simulink model "SimulinkAnalysisofCheetahTail"  (R2022a)
(part 7 of 21)

t6762 = -t4173.*(t1786+t1810+t1964+t2047+t2152-t2401-t2797-t2860-t3076+t3167-t3232-t3278+t3582+t3583-t3837+t1430.*(t539+t641).*3.36554e-3+t1181.*(t105-t465).*3.372786875e-3+t11.*t381.*(t534-t546).*3.372786875e-3);
t6763 = -t4162.*(t1692+t1899+t1910+t2152+t2155-t2401-t2936-t2962-t3031-t3147+t3307-t3387+t3582+t3583-t3837+t1430.*(t539+t641).*3.36554e-3+t1181.*(t105-t465).*3.36554e-3+t11.*t381.*(t534-t546).*3.36554e-3);
t6764 = (-t1262+t1701+t9.*t868.*(t105-t465)).*(t1786+t1810+t1964+t2047+t2152-t2401-t2797-t2860-t3076+t3167-t3232-t3278+t3582+t3583-t3837+t1430.*(t539+t641).*3.36554e-3+t1181.*(t105-t465).*3.372786875e-3+t11.*t381.*(t534-t546).*3.372786875e-3);
t6770 = -t4313.*(t1692+t1899+t1910+t2152+t2155-t2401-t2936-t2962-t3031-t3147+t3307-t3387+t3582+t3583-t3837+t1430.*(t539+t641).*3.36554e-3+t1181.*(t105-t465).*3.36554e-3+t11.*t381.*(t534-t546).*3.36554e-3);
t6772 = (t1332+t2368+t1512.*(t105-t465)).*(t1786+t1810+t1964+t2047+t2152-t2401-t2797-t2860-t3076+t3167-t3232-t3278+t3582+t3583-t3837+t1430.*(t539+t641).*3.36554e-3+t1181.*(t105-t465).*3.372786875e-3+t11.*t381.*(t534-t546).*3.372786875e-3);
t6773 = -t4392.*(t1692+t1786+t1910+t1964+t2305-t2600-t2797-t2860-t2936-t3147+t3167-t3232+t3720+t3721-t3903+t1430.*(t539+t641).*3.372816795e-3+t1181.*(t105-t465).*3.36554e-3+t11.*t381.*(t534-t546).*3.36554e-3);
t6775 = t4392.*(t1692+t1786+t1910+t1964+t2305-t2600-t2797-t2860-t2936-t3147+t3167-t3232+t3720+t3721-t3903+t1430.*(t539+t641).*3.372816795e-3+t1181.*(t105-t465).*3.36554e-3+t11.*t381.*(t534-t546).*3.36554e-3);
t6776 = (-t1331+t2317+t1510.*(t103-t544)).*(t1692+t1899+t1910+t2152+t2155-t2401-t2936-t2962-t3031-t3147+t3307-t3387+t3582+t3583-t3837+t1430.*(t539+t641).*3.36554e-3+t1181.*(t105-t465).*3.36554e-3+t11.*t381.*(t534-t546).*3.36554e-3);
t6779 = -t4408.*(t1692+t1786+t1910+t1964+t2305-t2600-t2797-t2860-t2936-t3147+t3167-t3232+t3720+t3721-t3903+t1430.*(t539+t641).*3.372816795e-3+t1181.*(t105-t465).*3.36554e-3+t11.*t381.*(t534-t546).*3.36554e-3);
t6780 = t4408.*(t1692+t1786+t1910+t1964+t2305-t2600-t2797-t2860-t2936-t3147+t3167-t3232+t3720+t3721-t3903+t1430.*(t539+t641).*3.372816795e-3+t1181.*(t105-t465).*3.36554e-3+t11.*t381.*(t534-t546).*3.36554e-3);
t6781 = -t4447.*(t1692+t1786+t1910+t1964+t2305-t2600-t2797-t2860-t2936-t3147+t3167-t3232+t3720+t3721-t3903+t1430.*(t539+t641).*3.372816795e-3+t1181.*(t105-t465).*3.36554e-3+t11.*t381.*(t534-t546).*3.36554e-3);
t6792 = t2857+t3260+t3337+t4641+t4878+t5445+t6599;
t6798 = t4203+t4298+t4306+t4747+t4991+t6557+t6628;
t3827 = -t3800;
t3895 = -t3861;
t3912 = -t3876;
t3920 = -t3891;
t3972 = -t3943;
t3973 = -t3945;
t4018 = -t3988;
t4039 = -t4017;
t4127 = -t4107;
t4183 = -t4170;
t4219 = -t4202;
t4257 = -t4243;
t4291 = -t4285;
t4314 = -t4303;
t4331 = -t4321;
t4369 = -t4362;
t4391 = -t4379;
t4397 = -t4385;
t4398 = -t4386;
t4417 = t1356+t2513+t2557;
t4443 = -t4429;
t4448 = -t4439;
t4456 = -t4451;
t4463 = -t4460;
t4510 = -t4504;
t4535 = -t4531;
t4540 = t4531./2.0;
t4544 = -t4536;
t4554 = -t4548;
t4565 = -t4559;
t4568 = -t4562;
t4579 = t4572./2.0;
t4582 = -t4577;
t4586 = t4484.*3.36554e-3;
t4590 = -t4587;
t4596 = t4498.*3.36554e-3;
t4607 = -t4601;
t4609 = -t4605;
t4627 = t4531.*3.36554e-3;
t4633 = t4536.*3.36554e-3;
t4635 = -t4624;
t4642 = t4531.*3.372786875e-3;
t4644 = t4531.*9.53094055e-4;
t4656 = -t4653;
t4658 = t4556.*3.36554e-3;
t4679 = -t4674;
t4680 = t4572.*3.36554e-3;
t4688 = t4577.*3.36554e-3;
t4689 = -t4687;
t4690 = -t4683;
t4693 = t4572.*9.52624335e-4;
t4694 = t4572.*3.372816795e-3;
t4696 = t4588.*3.36554e-3;
t4726 = t2389+t3643+t3670;
t4727 = -t4720;
t4765 = -t4761;
t4791 = -t4781;
t4792 = ITail.*t4173.*t4310;
t4793 = -t4786;
t4804 = -t4799;
t4813 = -t4810;
t4814 = t2678+t2772+t2779+t2808;
t4817 = ITail.*t4173.*t4350;
t4822 = t1116+t1700+t1821+t4383;
t4824 = t1153+t1162+t2033+t2075+t2089+t2143;
t4825 = t1157+t1244+t1959+t2086+t2137+t2165;
t4827 = ITail.*t4255.*t4350;
t4833 = t1313+t1895+t1904+t4350;
t4835 = ITail.*t4310.*t4311;
t4840 = -t4831;
t4857 = -t4844;
t4861 = -t4850;
t4863 = -t4851;
t4886 = dphi1.*t4879;
t4887 = dphi2.*t4879;
t4899 = ITail.*t4310.*t4382;
t4907 = -t4903;
t4910 = t2361+t4148+t4151;
t4916 = ITail.*t4350.*t4382;
t4917 = -t4915;
t4951 = t1948+t2017+t3989+t4021;
t4952 = t1951+t2011+t3991+t4016;
t4955 = -t4948;
t4981 = -t4974;
t4984 = -ITail.*t4409.*(t1396-t2573+t1430.*(t197-t537).*2.0);
t4985 = ITail.*t3961.*t4667;
t5001 = -t4996;
t5013 = t1467+t1479+t2559+t2623+t2652+t2659;
t5025 = -t5019;
t5028 = ITail.*t4409.*t4471;
t5034 = -ITail.*t4459.*(t1396-t2573+t1430.*(t197-t537).*2.0);
t5035 = -t5026;
t5045 = ITail.*t3961.*t4712;
t5049 = -ITail.*t4409.*(t1395-t2868+t1505.*(t534-t546).*2.0);
t5068 = ITail.*t4310.*t4592;
t5069 = -t5060;
t5071 = t59+t410+t504+t1068+t1650+t2727+t3203+t3914;
t5075 = -ITail.*t4667.*(-t1262+t1701+t9.*t868.*(t105-t465));
t5079 = t4173.*t4681;
t5087 = ITail.*t4277.*t4629;
t5089 = t1691+t1744+t2555+t2585+t2655+t2661;
t5094 = ITail.*t4459.*t4471;
t5100 = ITail.*t4310.*t4618;
t5106 = ITail.*t4350.*t4592;
t5107 = -ITail.*t4667.*(-t947+t1240.*(t105-t465)+t903.*(t534-t546));
t5108 = -ITail.*t4459.*(t1395-t2868+t1505.*(t534-t546).*2.0);
t5110 = ITail.*t4277.*t4657;
t5115 = t4173.*t4704;
t5117 = ITail.*t4313.*t4629;
t5118 = ITail.*t4459.*(t1395-t2868+t1505.*(t534-t546).*2.0);
t5124 = ITail.*t4310.*t4645;
t5132 = ITail.*t4173.*t4712;
t5134 = ITail.*t4277.*t4675;
t5138 = ITail.*t4350.*t4618;
t5140 = -ITail.*t4712.*(-t1262+t1701+t9.*t868.*(t105-t465));
t5142 = -t5136;
t5145 = ITail.*t4313.*t4657;
t5148 = ITail.*t4409.*t4578;
t5157 = t4255.*t4704;
t5162 = ITail.*t4350.*t4645;
t5168 = t4311.*t4681;
t5169 = ITail.*t4313.*t4675;
t5170 = -ITail.*t4162.*(t907+t1157-t1544+t2086+t2137+(t11.*t420.*(t214-t541))./2.0);
t5175 = t1516+t1549+t2941+t2943+t2973+t2998;
t5180 = ITail.*t4162.*(t907+t1157-t1544+t2086+t2137+(t11.*t420.*(t214-t541))./2.0);
t5183 = t1015+t1643+t1782+t2354+t3826+t3892;
t5186 = -t5176;
t5187 = t1014+t1696+t1699+t2356+t3850+t3860;
t5188 = ITail.*t4452.*t4578;
t5196 = -ITail.*t4629.*(-t1331+t2317+t1510.*(t103-t544));
t5211 = ITail.*t4077.*t4785;
t5212 = ITail.*t4459.*t4578;
t5216 = t3775+t3807+t3809+t3824;
t5221 = -ITail.*t4350.*(t995+t1064-t1506+t1598-t1763-t1774);
t5222 = -ITail.*t4657.*(-t1331+t2317+t1510.*(t103-t544));
t5226 = -t5215;
t5228 = -ITail.*t4667.*(t1332+t2368+t1512.*(t105-t465));
t5231 = t4382.*t4681;
t5233 = -t4634.*(t1396-t2573+t1430.*(t197-t537).*2.0);
t5234 = ITail.*t4657.*(-t1331+t2317+t1510.*(t103-t544));
t5235 = -ITail.*t4350.*(t820+t1121-t1435+t1997+t2000+t11.*t420.*(t214-t541));
t5243 = ITail.*t4350.*(t820+t1121-t1435+t1997+t2000+t11.*t420.*(t214-t541));
t5245 = -t5237;
t5247 = -ITail.*t4310.*(t1064+t1137-t1694+t1698-t1763-t1774);
t5248 = t1134+t1780+t1783+t2525+t3891+t3894;
t5249 = -ITail.*t4675.*(-t1331+t2317+t1510.*(t103-t544));
t5252 = t1136+t1748+t1781+t2533+t3893+t3896;
t5253 = -t5246;
t5254 = ITail.*t3961.*(t1153+t2075-t4310-(t1178.*(t105-t465))./2.0);
t5258 = t3614+t4347+t4351;
t5259 = ITail.*t4162.*t4783;
t5260 = -ITail.*t4313.*(t907+t1157-t1544+t2086+t2137+(t11.*t420.*(t214-t541))./2.0);
t5262 = ITail.*t4522.*t4578;
t5264 = ITail.*t4071.*t4820;
t5269 = ITail.*t4313.*(t907+t1157-t1544+t2086+t2137+(t11.*t420.*(t214-t541))./2.0);
t5270 = t4382.*t4704;
t5276 = -ITail.*t3961.*(t1264+t1882-t4350+(t1047.*(t105-t465))./2.0);
t5277 = -t5266;
t5279 = -t5271;
t5281 = t4471.*t4634;
t5284 = ITail.*t4310.*t4738;
t5292 = -ITail.*t4712.*(t1332+t2368+t1512.*(t105-t465));
t5295 = ITail.*t3961.*t4867;
t5296 = -t5288;
t5297 = ITail.*t3938.*t4881;
t5298 = -t4634.*(t1395-t2868+t1505.*(t534-t546).*2.0);
t5305 = -ITail.*t4350.*(t867+t1059-t1646-t1705+t1938-t2002);
t5307 = ITail.*t4162.*t4816;
t5314 = -t5306;
t5322 = ITail.*t4277.*t4783;
t5330 = ITail.*t3938.*t4900;
t5332 = ITail.*t4310.*t4770;
t5333 = ITail.*t4214.*t4820;
t5337 = ITail.*t4173.*(t1153+t2075-t4310-(t1178.*(t105-t465))./2.0);
t5339 = ITail.*(-t1331+t2317+t1510.*(t103-t544)).*(t907+t1157-t1544+t2086+t2137+(t11.*t420.*(t214-t541))./2.0);
t5341 = dphi2.*t5334;
t5343 = -ITail.*(-t1262+t1701+t9.*t868.*(t105-t465)).*(t1153+t2075-t4310-(t1178.*(t105-t465))./2.0);
t5350 = -ITail.*t4820.*(-t1355+t1789+(t9.*t868.*(t105-t465))./2.0);
t5355 = -ITail.*t4173.*(t1264+t1882-t4350+(t1047.*(t105-t465))./2.0);
t5357 = dphi2.*t5348;
t5359 = ITail.*t4277.*t4816;
t5360 = ITail.*t4173.*(t1264+t1882-t4350+(t1047.*(t105-t465))./2.0);
t5361 = ITail.*(-t1262+t1701+t9.*t868.*(t105-t465)).*(t1264+t1882-t4350+(t1047.*(t105-t465))./2.0);
t5366 = t1076+t1947+t2109+t2428+t3988+t4040;
t5371 = -ITail.*t4310.*(t1060+t1138-t1883+t1932+t2088+t1179.*(t103-t544));
t5376 = -ITail.*(-t947+t1240.*(t105-t465)+t903.*(t534-t546)).*(t1153+t2075-t4310-(t1178.*(t105-t465))./2.0);
t5377 = ITail.*t4173.*t4867;
t5381 = -t5370;
t5383 = ITail.*t4310.*(t1060+t1138-t1883+t1932+t2088+t1179.*(t103-t544));
t5388 = ITail.*t3938.*t4928;
t5389 = -ITail.*t4867.*(-t1262+t1701+t9.*t868.*(t105-t465));
t5394 = t1875+t2253+t2629+t2726+t3547+t3555;
t5395 = -ITail.*t4820.*(-t1017+(t1240.*(t105-t465))./2.0+(t903.*(t534-t546))./2.0);
t5400 = -ITail.*t4310.*(t1250-t1261+t1761-t2083-t2111+t1037.*(t103-t544));
t5402 = ITail.*(-t947+t1240.*(t105-t465)+t903.*(t534-t546)).*(t1264+t1882-t4350+(t1047.*(t105-t465))./2.0);
t5403 = t4578.*t4634;
t5408 = -t5401;
t5411 = -ITail.*t4310.*(t1053+t1332+t2368+t817.*(t214-t541)+t977.*(t103-t544)+t1512.*(t105-t465));
t5414 = -t5405;
t5415 = -t4753.*(t1396-t2573+t1430.*(t197-t537).*2.0);
t5416 = -ITail.*t4350.*(t1060+t1138-t1883+t1932+t2088+t1179.*(t103-t544));
t5418 = -ITail.*t4867.*(-t947+t1240.*(t105-t465)+t903.*(t534-t546));
t5426 = -ITail.*t4783.*(-t1331+t2317+t1510.*(t103-t544));
t5434 = t1961+t2253+t2800+t2858+t3547+t3555;
t5436 = -t5429;
t5440 = -ITail.*t4350.*(t1250-t1261+t1761-t2083-t2111+t1037.*(t103-t544));
t5442 = t1875+t2386+t2629+t2726+t3639+t3690;
t5449 = -t5437;
t5450 = ITail.*t4350.*(t1250-t1261+t1761-t2083-t2111+t1037.*(t103-t544));
t5454 = -ITail.*t4350.*(t1053+t1332+t2368+t817.*(t214-t541)+t977.*(t103-t544)+t1512.*(t105-t465));
t5462 = ITail.*t4350.*(t1053+t1332+t2368+t817.*(t214-t541)+t977.*(t103-t544)+t1512.*(t105-t465));
t5465 = t4471.*t4753;
t5467 = t4592.*t4681;
t5468 = -ITail.*t4459.*(t2436-t2536+t1510.*(t197-t537)+t1505.*(t214-t541));
t5469 = -ITail.*t4816.*(-t1331+t2317+t1510.*(t103-t544));
t5471 = ITail.*t4452.*t4785;
t5478 = ITail.*t4816.*(-t1331+t2317+t1510.*(t103-t544));
t5482 = -t4753.*(t1395-t2868+t1505.*(t534-t546).*2.0);
t5483 = t3961.*t4989;
t5487 = -t5477;
t5489 = t4753.*(t1395-t2868+t1505.*(t534-t546).*2.0);
t5495 = ITail.*t4459.*t4785;
t5496 = t4618.*t4681;
t5497 = ITail.*t4077.*t4972;
t5499 = ITail.*t4409.*t4821;
t5500 = t4592.*t4704;
t5501 = t2134+t2179+t3286+t3290+t3329+t3378;
t5508 = -t5502;
t5510 = ITail.*t4409.*t4823;
t5513 = -t5509;
t5515 = t4645.*t4681;
t5520 = t4392.*t4858;
t5526 = -ITail.*t4409.*(-t1129+t1139-t2082+t2110+t2123+t8.*t872.*(t534-t546));
t5531 = -t5521;
t5532 = t4618.*t4704;
t5534 = ITail.*t4409.*t4834;
t5535 = ITail.*t4409.*(-t1129+t1139-t2082+t2110+t2123+t8.*t872.*(t534-t546));
C = ft_12({B_cg_H,ITail,Mb,Mm,Mt,T_cg_H,dphi1,dphi2,dpsi1,dth1,dth2,dx,dy,dz,t10,t1005,t1006,t1007,t1008,t1009,t1013,t1016,t1017,t1018,t1019,t1023,t1029,t103,t1037,t1047,t105,t1050,t1053,t1059,t1060,t1064,t1071,t1072,t1075,t1077,t1078,t1079,t1084,t1086,t1088,t1097,t1099,t11,t1102,t1108,t1113,t1121,t1129,t1133,t1135,t1137,t1138,t1139,t1141,t1142,t1143,t1147,t1149,t1153,t1155,t1157,t1159,t1160,t1164,t1167,t1169,t1170,t1173,t1176,t1178,t1179,t1181,t1185,t1186,t1189,t1193,t1194,t1195,t1196,t120,t1200,t1203,t1205,t1206,t1211,t1215,t1221,t1223,t1224,t1225,t1228,t1229,t1230,t1234,t1240,t1242,t1245,t1246,t1247,t1250,t1252,t1253,t1255,t1260,t1261,t1262,t1264,t1265,t1268,t1280,t1283,t1291,t130,t1301,t1302,t1303,t1304,t1305,t1307,t1309,t1322,t1328,t1331,t1332,t1334,t1337,t1338,t134,t1343,t1344,t1345,t1348,t1352,t1354,t1355,t1360,t1362,t1365,t1366,t1368,t1370,t1371,t1373,t1374,t1378,t1381,t1382,t1384,t1386,t1388,t1389,t1391,t1393,t1394,t1395,t1396,t1397,t1406,t1412,t1413,t1415,t1421,t1426,t1427,t1430,t1431,t1433,t1435,t144,t1441,t1443,t1444,t1446,t1453,t1455,t1456,t1457,t1458,t1460,t1465,t1466,t1468,t1470,t1476,t1481,t1486,t1487,t1495,t15,t1505,t1506,t1508,t1510,t1512,t1513,t1518,t1521,t1525,t1526,t1528,t1529,t1531,t1535,t1540,t1543,t1544,t1552,t1558,t1562,t1568,t1575,t1578,t1581,t1586,t1593,t1596,t1597,t1598,t1609,t161,t1612,t1618,t1619,t162,t1620,t1621,t1624,t1627,t1628,t1633,t1634,t1635,t1637,t1639,t1640,t1645,t1646,t1651,t1652,t1654,t1655,t1656,t1657,t1659,t1660,t1661,t1664,t1665,t1667,t1672,t1674,t1676,t1678,t1680,t1681,t1682,t1683,t1685,t1692,t1693,t1694,t1695,t1698,t1701,t1702,t1703,t1705,t1706,t1716,t1718,t1719,t1720,t1721,t1722,t1725,t1727,t1730,t1734,t1735,t1736,t1737,t1739,t1741,t1742,t1746,t1747,t1748,t1751,t1752,t1759,t1761,t1763,t1764,t1771,t1774,t1777,t1778,t1779,t1781,t1784,t1785,t1786,t1787,t1788,t1789,t1790,t1792,t1799,t1800,t1801,t1802,t1806,t1809,t1810,t1813,t1832,t1836,t1840,t1843,t1846,t1851,t1853,t1855,t1857,t1858,t1859,t1860,t1865,t1866,t1867,t1882,t1883,t1888,t1890,t1896,t1898,t1899,t1900,t1907,t1910,t1915,t1917,t1918,t1928,t1929,t1932,t1938,t1939,t1942,t1943,t1945,t195,t1950,t1952,t1956,t1957,t1959,t1962,t1964,t1965,t197,t1970,t1971,t1974,t1976,t1977,t1979,t1981,t1982,t1983,t1993,t1997,t1999,t2,t2000,t2002,t2004,t2007,t2008,t2009,t2012,t2013,t2015,t2016,t2018,t2020,t2023,t2024,t2032,t2037,t2038,t2047,t2049,t2050,t2057,t2058,t2059,t2061,t2062,t2064,t2065,t2067,t2068,t2069,t2072,t2075,t2076,t2081,t2082,t2083,t2086,t2087,t2088,t2096,t2104,t2106,t2107,t2108,t2110,t2111,t2113,t2117,t2119,t2123,t2130,t2131,t2134,t2135,t2137,t2139,t214,t2141,t2147,t2148,t2150,t2152,t2153,t2155,t2156,t2158,t2161,t2174,t2175,t2178,t2183,t2186,t2188,t2189,t2190,t2191,t2192,t2196,t2197,t2202,t2203,t2206,t2208,t2210,t2212,t2215,t2218,t2220,t2222,t2223,t2225,t2227,t2237,t2240,t2241,t2242,t2243,t2247,t2248,t2249,t2254,t2255,t2257,t2259,t2260,t2263,t2268,t2269,t2271,t2274,t2276,t2281,t2282,t2285,t2286,t2287,t2289,t2293,t2305,t2308,t2312,t2316,t2317,t2319,t2322,t2325,t2329,t2334,t2336,t2338,t2339,t2341,t2342,t2343,t2345,t2347,t2348,t2352,t2358,t2360,t2361,t2364,t2368,t2376,t2387,t2388,t2389,t2390,t2391,t2397,t2399,t24,t2401,t2404,t2406,t2409,t2410,t2411,t2412,t2413,t2419,t2420,t2426,t2427,t2429,t2430,t2434,t2435,t2436,t2438,t2447,t2449,t2458,t2463,t2465,t2468,t2471,t2472,t2479,t2483,t2485,t2487,t2489,t2492,t2495,t2496,t25,t2501,t2503,t2504,t2512,t2514,t2515,t2516,t2518,t2522,t2523,t2524,t2526,t2527,t2528,t2535,t2536,t2543,t2547,t2563,t2564,t2567,t2568,t2569,t2571,t2573,t2574,t2576,t2578,t2579,t2581,t2582,t2587,t2589,t259,t2590,t2591,t2597,t2599,t26,t260,t2600,t2605,t2613,t2616,t2617,t2621,t2624,t2627,t2632,t2636,t2637,t2638,t2646,t2648,t2657,t2660,t2662,t2663,t2665,t2667,t2668,t2669,t2673,t2679,t2684,t2688,t2692,t2696,t2698,t2699,t27,t2700,t2706,t2707,t2708,t2710,t2712,t2715,t2717,t2718,t2722,t2723,t2728,t2730,t2733,t2734,t2735,t2736,t2737,t2738,t2743,t2744,t2746,t2750,t2754,t2759,t276,t2763,t277,t2778,t2783,t2785,t2787,t2790,t2791,t2792,t2794,t2796,t2797,t2798,t2799,t2803,t2805,t2811,t2816,t2817,t2818,t2819,t2821,t2823,t2824,t2825,t2829,t283,t2831,t2833,t2834,t2836,t2839,t284,t2842,t2843,t2844,t2845,t2847,t2849,t285,t2853,t286,t2860,t2861,t2868,t287,t2871,t2875,t2876,t2877,t2878,t2879,t288,t2882,t2883,t2884,t2887,t2889,t289,t2899,t290,t291,t2912,t2913,t2914,t2915,t2917,t2918,t292,t2920,t2921,t2927,t2928,t293,t2930,t2936,t2937,t294,t2942,t2944,t2945,t2950,t2952,t2954,t2956,t2962,t2963,t2965,t2970,t2972,t2977,t2978,t2981,t2982,t2989,t2994,t2996,t2997,t3,t3008,t3009,t3012,t3022,t3027,t3030,t3031,t3034,t3035,t3038,t304,t3040,t3050,t3054,t3059,t3062,t3063,t3064,t3070,t3076,t3080,t3082,t3084,t3085,t3086,t3087,t3089,t3090,t3091,t3093,t3094,t3096,t3105,t3106,t3107,t3109,t3110,t3113,t3117,t3121,t3122,t3127,t3131,t3138,t3139,t3146,t3147,t3149,t3151,t3155,t3160,t3161,t3167,t3169,t3170,t3171,t3173,t3176,t3177,t3178,t3179,t3180,t3186,t3187,t3190,t3192,t3193,t3199,t3204,t3206,t3207,t3210,t3212,t3213,t3214,t3216,t3217,t3222,t3230,t3232,t3233,t3235,t3236,t3243,t3244,t3247,t3248,t3252,t3256,t3257,t3261,t3262,t3263,t3265,t3266,t3267,t3270,t3272,t3273,t3276,t3277,t3278,t3284,t3286,t3287,t3289,t3299,t3302,t3304,t3307,t3308,t3311,t3312,t3315,t3320,t3321,t3322,t3325,t3326,t3328,t3329,t3330,t3331,t3333,t3335,t3336,t3339,t3341,t3343,t3344,t3347,t3351,t3354,t3357,t3359,t3376,t3378,t3379,t3380,t3381,t3385,t3387,t3390,t3391,t3392,t3397,t3402,t3403,t3406,t3407,t3411,t3412,t3413,t3414,t3415,t3416,t3419,t3423,t3424,t3427,t3429,t3431,t3432,t3433,t3437,t3438,t3439,t3441,t3442,t3445,t3448,t3449,t3458,t3459,t3460,t3463,t3467,t3471,t3473,t3475,t3476,t3480,t3481,t3482,t3483,t3485,t3486,t3487,t3489,t3490,t3494,t3499,t3501,t3504,t3506,t3510,t3512,t3516,t3521,t3522,t3523,t3524,t3526,t3528,t3529,t3530,t3531,t3534,t3540,t3541,t3543,t3544,t3545,t3548,t3550,t3552,t3553,t3554,t3556,t3557,t3563,t3570,t3571,t3575,t3576,t3578,t3582,t3583,t3584,t3587,t3594,t3597,t3598,t3600,t3602,t3609,t3614,t3617,t3619,t3621,t3627,t3632,t3634,t3638,t3644,t3647,t3648,t3649,t3651,t3652,t3657,t3659,t3661,t3667,t3668,t3671,t3672,t3678,t3679,t3680,t3681,t3682,t3683,t3684,t3685,t3686,t3687,t3689,t3697,t3698,t3701,t3702,t3704,t3709,t3710,t3711,t3716,t3719,t3720,t3721,t3722,t3723,t3724,t3730,t3735,t3738,t3739,t3742,t3744,t3745,t3746,t3748,t3749,t3750,t3755,t3756,t3757,t3758,t3759,t376,t3764,t3766,t3769,t377,t3770,t3771,t3772,t3773,t3774,t3777,t3779,t3780,t3784,t3787,t3791,t3792,t3793,t3794,t3797,t3798,t3802,t3804,t3805,t3808,t381,t3811,t3812,t3814,t3815,t3817,t382,t3820,t3823,t3825,t3827,t3828,t383,t3832,t3834,t3836,t3837,t3838,t3841,t3845,t3847,t3848,t3849,t3851,t3855,t3856,t3858,t3859,t3862,t3867,t3868,t3870,t3871,t3879,t3880,t3882,t3883,t3885,t3887,t3889,t3893,t3895,t3896,t3898,t390,t3900,t3902,t3903,t3906,t3907,t3908,t3909,t3912,t3915,t3916,t3918,t3920,t3921,t3923,t3925,t3926,t3928,t3929,t3930,t3931,t3932,t3933,t3934,t3936,t3937,t3938,t3939,t394,t3940,t3943,t3944,t3945,t3947,t3948,t3949,t3950,t3951,t3952,t3953,t3954,t3955,t3956,t3957,t3958,t3959,t3960,t3961,t3962,t3964,t3965,t3966,t3967,t3969,t3971,t3972,t3973,t3974,t3975,t3976,t3977,t3979,t3980,t3981,t3982,t3983,t3984,t3985,t3986,t3992,t3993,t3995,t3996,t3998,t4,t4000,t4001,t4003,t4005,t4006,t4007,t4008,t4009,t4010,t4012,t4014,t4017,t4018,t4019,t4020,t4022,t4023,t4024,t4025,t4026,t4027,t4028,t4029,t4033,t4034,t4035,t4036,t4037,t4038,t4039,t4041,t4042,t4044,t4046,t4047,t4048,t4050,t4051,t4052,t4053,t4054,t4056,t4058,t4059,t4061,t4062,t4064,t4065,t4066,t4068,t4070,t4071,t4072,t4073,t4074,t4077,t4078,t4081,t4083,t4084,t4085,t4086,t4087,t4089,t4090,t4091,t4092,t4094,t4095,t4096,t4097,t4098,t4099,t410,t4100,t4104,t4105,t4107,t4108,t4109,t411,t4111,t4112,t4115,t4116,t4117,t4119,t412,t4120,t4121,t4122,t4126,t4127,t4129,t413,t4132,t4133,t4135,t4137,t4138,t4139,t414,t4140,t4141,t4143,t4144,t4145,t4147,t415,t4152,t4153,t4154,t4155,t4156,t4157,t4160,t4162,t4164,t4165,t4169,t4170,t4171,t4173,t4174,t4179,t4182,t4183,t4184,t4186,t4187,t4188,t4189,t4190,t4195,t4196,t4197,t420,t4200,t4201,t4204,t4205,t4206,t4208,t4209,t421,t4210,t4211,t4212,t4213,t4214,t4215,t4216,t4217,t4218,t4219,t4220,t4221,t4222,t4223,t4224,t4225,t4226,t4227,t4228,t4231,t4232,t4233,t4234,t4236,t4237,t4238,t4239,t4240,t4241,t4243,t4244,t4245,t4246,t4247,t4248,t4249,t425,t4250,t4252,t4253,t4255,t4256,t4257,t4258,t4259,t4260,t4261,t4262,t4263,t4265,t4266,t4268,t4269,t4271,t4272,t4273,t4274,t4276,t4277,t4278,t4280,t4281,t4282,t4286,t4290,t4291,t4295,t4296,t430,t4300,t4301,t4302,t4303,t4304,t4305,t4307,t4308,t4309,t431,t4310,t4311,t4312,t4313,t4314,t4315,t4316,t4317,t4318,t4319,t4320,t4321,t4322,t4323,t4324,t4326,t4327,t4329,t433,t4330,t4331,t4332,t4333,t4334,t4337,t4339,t4340,t4341,t4342,t4343,t4344,t4345,t4346,t4348,t4349,t4350,t4352,t4354,t4355,t4356,t4357,t4358,t4359,t436,t4360,t4361,t4364,t4365,t4367,t4368,t4369,t4370,t4371,t4372,t4373,t4374,t4375,t4376,t4377,t4378,t4379,t4380,t4382,t4384,t4385,t4386,t4387,t4388,t4389,t4391,t4392,t4393,t4394,t4395,t4397,t4398,t4399,t44,t4400,t4401,t4402,t4403,t4404,t4405,t4406,t4407,t4408,t4409,t4411,t4412,t4413,t4414,t4415,t4416,t4417,t4418,t4419,t4420,t4421,t4422,t4424,t4425,t4427,t4428,t4429,t4431,t4432,t4433,t4434,t4435,t4437,t4438,t4439,t4440,t4442,t4443,t4444,t4447,t4448,t4449,t445,t4450,t4451,t4452,t4453,t4454,t4455,t4456,t4457,t4458,t4459,t4460,t4461,t4462,t4463,t4465,t4467,t4469,t4470,t4471,t4472,t4473,t4475,t4476,t4477,t4478,t4479,t4480,t4481,t4482,t4483,t4484,t4485,t4486,t4487,t4488,t4489,t4490,t4492,t4493,t4495,t4496,t4497,t4498,t4499,t4500,t4501,t4502,t4503,t4505,t4506,t4507,t451,t4510,t4511,t4512,t4514,t4515,t4517,t4518,t4519,t4520,t4521,t4522,t4523,t4524,t4525,t4526,t4528,t4529,t4530,t4531,t4532,t4533,t4534,t4535,t4536,t4537,t4538,t4540,t4541,t4542,t4544,t4545,t4546,t4547,t4549,t4550,t4551,t4552,t4553,t4554,t4555,t4556,t4557,t4558,t4559,t4560,t4561,t4562,t4563,t4565,t4566,t4567,t4568,t4570,t4571,t4572,t4573,t4574,t4575,t4576,t4577,t4578,t4579,t4580,t4581,t4582,t4583,t4584,t4585,t4586,t4588,t4589,t459,t4590,t4591,t4592,t4596,t4597,t4598,t4600,t4601,t4602,t4603,t4604,t4605,t4606,t4607,t4608,t4609,t4610,t4613,t4614,t4615,t4616,t4617,t4618,t4619,t4620,t4621,t4622,t4623,t4624,t4625,t4626,t4627,t4629,t4630,t4633,t4634,t4635,t4636,t4637,t4638,t4639,t4642,t4644,t4645,t4646,t4647,t4649,t465,t4651,t4652,t4655,t4656,t4657,t4658,t4659,t4660,t4661,t4662,t4663,t4664,t4665,t4666,t4667,t4668,t4669,t4672,t4673,t4674,t4675,t4678,t4679,t4680,t4681,t4682,t4684,t4685,t4686,t4688,t4689,t4690,t4693,t4694,t4695,t4696,t4697,t4698,t4700,t4701,t4702,t4704,t4705,t4706,t4707,t4708,t4709,t4710,t4711,t4712,t4713,t4722,t4723,t4724,t4727,t4729,t4732,t4733,t4735,t4736,t4737,t4738,t4742,t4746,t4749,t4750,t4751,t4752,t4753,t4754,t4755,t4756,t4758,t4759,t4761,t4764,t4765,t4766,t4769,t4770,t4771,t4772,t4773,t4775,t4776,t4780,t4783,t4784,t4785,t4786,t4787,t4788,t4789,t4790,t4791,t4792,t4793,t4796,t4799,t48,t4800,t4801,t4802,t4803,t4804,t4805,t4806,t4807,t4809,t4811,t4813,t4814,t4815,t4816,t4817,t4820,t4821,t4823,t4826,t4827,t4830,t4832,t4834,t4835,t4836,t4838,t4840,t4841,t4843,t4845,t4846,t4847,t4848,t4849,t485,t4850,t4851,t4852,t4853,t4857,t4858,t4861,t4862,t4863,t4864,t4865,t4867,t4870,t4871,t4873,t4874,t4877,t488,t4880,t4881,t4882,t4883,t4884,t4886,t4887,t4888,t4889,t4890,t4892,t4895,t4897,t4899,t49,t4900,t4901,t4904,t4906,t4907,t4908,t4909,t4911,t4912,t4913,t4914,t4916,t4917,t4922,t4923,t4924,t4925,t4926,t4927,t4928,t4929,t4931,t4932,t4933,t4934,t4936,t4937,t4938,t4939,t4940,t4941,t4942,t4943,t4944,t4945,t4946,t4947,t4949,t4950,t4951,t4952,t4953,t4954,t4955,t496,t4960,t4961,t4963,t4964,t4966,t4967,t4968,t4969,t4972,t4973,t4975,t4976,t4977,t4978,t4979,t4980,t4981,t4982,t4983,t4984,t4985,t4986,t4987,t4988,t4989,t4990,t4993,t4995,t4997,t4998,t4999,t5,t50,t5000,t5001,t5002,t5004,t5005,t5006,t5007,t5008,t5009,t501,t5010,t5012,t5013,t5014,t5016,t5017,t5018,t502,t5021,t5022,t5023,t5024,t5025,t5027,t5028,t5030,t5031,t5032,t5033,t5034,t5035,t5036,t5038,t5039,t504,t5040,t5041,t5042,t5045,t5046,t5047,t5048,t5049,t5050,t5051,t5052,t5053,t5054,t5055,t5057,t5058,t5059,t5061,t5062,t5063,t5064,t5066,t5067,t5068,t5069,t5071,t5072,t5074,t5075,t5076,t5077,t5078,t5079,t5080,t5082,t5083,t5084,t5085,t5087,t5088,t5089,t5090,t5092,t5093,t5094,t5095,t5098,t5099,t51,t5100,t5101,t5102,t5103,t5104,t5106,t5107,t5109,t5110,t5111,t5112,t5114,t5115,t5117,t5118,t5120,t5121,t5123,t5124,t5126,t5128,t5131,t5132,t5134,t5135,t5136,t5137,t5138,t5139,t5140,t5142,t5143,t5144,t5145,t5146,t5148,t5149,t5150,t5152,t5153,t5154,t5155,t5156,t5157,t5158,t5161,t5162,t5163,t5165,t5166,t5167,t5168,t5169,t5171,t5172,t5173,t5174,t5175,t5177,t5178,t5179,t5180,t5182,t5183,t5184,t5185,t5186,t5187,t5188,t519,t5190,t5191,t5193,t5194,t5196,t5197,t5198,t5199,t5202,t5203,t5204,t5205,t5206,t5207,t5208,t5211,t5212,t5214,t5216,t5217,t5218,t5220,t5221,t5223,t5224,t5225,t5226,t5227,t5228,t5229,t523,t5231,t5232,t5233,t5234,t5235,t5238,t5239,t524,t5240,t5241,t5243,t5244,t5245,t5247,t5248,t5249,t5250,t5251,t5252,t5253,t5254,t5256,t5259,t5260,t5262,t5263,t5264,t5265,t5266,t5268,t5269,t527,t5270,t5272,t5274,t5275,t5276,t5277,t5279,t5280,t5281,t5284,t5285,t5286,t5287,t5288,t5289,t5290,t5291,t5292,t5293,t5294,t5295,t5296,t5297,t5298,t5299,t530,t5300,t5301,t5302,t5304,t5305,t5306,t5307,t5308,t5309,t5310,t5311,t5312,t5313,t5314,t5316,t5317,t5318,t5319,t5321,t5322,t5324,t5325,t5326,t5327,t5328,t5329,t5330,t5332,t5333,t5335,t5336,t5337,t5338,t5339,t534,t5340,t5341,t5343,t5344,t5345,t5346,t5347,t5349,t5350,t5351,t5352,t5353,t5354,t5356,t5357,t5358,t5359,t5360,t5361,t5363,t5364,t5366,t5368,t5369,t537,t5370,t5371,t5372,t5374,t5376,t5377,t5378,t5379,t5380,t5381,t5382,t5383,t5384,t5385,t5386,t5388,t5389,t539,t5391,t5392,t5393,t5394,t5395,t5396,t5398,t5399,t54,t5400,t5402,t5403,t5404,t5405,t5406,t5407,t5408,t5409,t541,t5411,t5412,t5413,t5414,t5415,t5416,t5417,t5418,t5419,t542,t5420,t5421,t5422,t5423,t5425,t5426,t5427,t5428,t5430,t5431,t5434,t5435,t5436,t5438,t5439,t544,t5441,t5442,t5443,t5444,t5447,t5448,t5449,t5450,t5452,t5453,t5455,t5456,t5458,t5459,t546,t5460,t5461,t5462,t5463,t5464,t5465,t5467,t5468,t5470,t5471,t5474,t5475,t5476,t5478,t5480,t5481,t5483,t5484,t5486,t5487,t5488,t5489,t5490,t5492,t5493,t5494,t5495,t5496,t5497,t5498,t5499,t55,t550,t5500,t5502,t5508,t5509,t5510,t5511,t5513,t5514,t5515,t5516,t5519,t5520,t5521,t5523,t5524,t5527,t5528,t553,t5530,t5531,t5532,t5533,t5534,t5535,t5536,t5538,t5539,t5540,t5542,t5543,t5546,t5547,t5548,t5550,t5551,t5552,t5553,t5556,t5557,t5563,t5565,t5566,t5569,t557,t5571,t5573,t5575,t5576,t5578,t558,t5580,t5582,t5585,t5588,t5592,t5597,t5598,t5599,t56,t5601,t5602,t5603,t5606,t5607,t5616,t5618,t5619,t5620,t5622,t5623,t5627,t5629,t5631,t5632,t5633,t5638,t5642,t5644,t5648,t5657,t5658,t5659,t5660,t5661,t5662,t5663,t5664,t5667,t5668,t5670,t5672,t5674,t5677,t5678,t5682,t5684,t5685,t5686,t5687,t5688,t5689,t5690,t5691,t5692,t5693,t5694,t5696,t5697,t5699,t5704,t5705,t5706,t5707,t5709,t5710,t5712,t5713,t5715,t5717,t5721,t5722,t5724,t5726,t573,t5730,t5731,t5733,t5734,t5738,t574,t5741,t5745,t5749,t575,t5754,t5756,t5761,t5763,t5771,t5772,t5776,t5778,t5779,t5780,t5781,t5785,t5786,t5788,t5789,t5791,t5792,t5793,t5795,t5798,t5800,t5805,t5808,t5809,t5814,t5815,t5818,t5820,t5823,t5824,t5826,t5829,t5832,t5835,t5837,t5840,t5841,t5843,t5845,t5846,t5847,t5848,t5855,t5857,t5859,t5862,t5867,t5868,t5869,t587,t5870,t5874,t5880,t5881,t5887,t5889,t5891,t5894,t5895,t5897,t59,t5901,t5905,t5908,t5909,t5910,t5915,t5916,t5917,t5919,t5923,t5925,t5926,t5932,t5933,t5935,t5936,t5939,t5941,t5947,t5949,t595,t5959,t5960,t5963,t5964,t5967,t5970,t5971,t5973,t5980,t5981,t5982,t5983,t5984,t5985,t5986,t5988,t5989,t5990,t5991,t5992,t5996,t5998,t6000,t6001,t6009,t6010,t6013,t6014,t6015,t6021,t6024,t6026,t6029,t603,t6030,t6036,t6039,t6042,t6045,t6049,t6051,t6052,t6056,t6057,t6058,t6066,t6069,t6074,t6075,t6086,t6089,t6090,t6091,t6099,t61,t6101,t6104,t6105,t6106,t6111,t6117,t6125,t6128,t6129,t6138,t614,t6140,t6143,t6150,t6158,t6161,t6164,t6166,t6171,t6174,t6176,t6182,t6183,t6191,t6195,t6196,t6197,t6198,t6199,t6204,t6205,t6211,t6219,t6221,t6222,t6225,t6229,t6230,t6231,t6234,t6236,t6240,t6241,t6249,t6253,t6258,t6261,t6264,t6268,t6273,t6274,t6275,t6277,t6278,t628,t6281,t6282,t6284,t629,t6290,t6292,t6295,t6296,t6303,t6304,t6309,t6311,t6314,t6315,t6316,t6317,t6320,t6330,t6332,t634,t6345,t6347,t6351,t6354,t6356,t6361,t6365,t6369,t6370,t6372,t6385,t6388,t6389,t6391,t6393,t6399,t6400,t6405,t6406,t6409,t641,t6410,t6413,t6421,t6422,t6430,t6433,t6434,t6439,t6443,t6446,t6447,t6448,t6449,t6450,t6455,t6460,t6471,t6482,t6483,t6484,t6485,t6486,t6487,t6495,t6497,t65,t650,t6501,t6506,t651,t6510,t6526,t6531,t6538,t6539,t6549,t655,t6550,t6552,t6555,t6562,t6565,t6567,t657,t6571,t6580,t6581,t6584,t6588,t6602,t6611,t6612,t6613,t6614,t6615,t6616,t6617,t6618,t6619,t6620,t6629,t6630,t6634,t6635,t6636,t6637,t6638,t664,t6640,t6641,t6645,t6646,t6647,t665,t6653,t6656,t666,t6669,t667,t6673,t6677,t668,t6681,t669,t6699,t6709,t6729,t6739,t6743,t6745,t675,t6754,t6755,t6756,t6762,t6763,t6764,t6770,t6772,t6773,t6775,t6776,t6779,t6780,t6781,t6792,t6798,t68,t693,t7,t71,t721,t724,t73,t731,t732,t736,t741,t753,t754,t755,t757,t765,t769,t772,t774,t776,t778,t795,t797,t799,t8,t802,t803,t806,t817,t818,t820,t828,t831,t838,t843,t846,t847,t850,t851,t852,t853,t855,t865,t867,t868,t870,t871,t872,t876,t886,t888,t9,t901,t902,t903,t904,t907,t909,t914,t925,t926,t947,t949,t952,t955,t957,t964,t972,t977,t983,t991,t992,t993,t994,t995});
end
function C = ft_12(ct)
B_cg_H = ct{1};
ITail = ct{2};
Mb = ct{3};
Mm = ct{4};
Mt = ct{5};
T_cg_H = ct{6};
dphi1 = ct{7};
dphi2 = ct{8};
dpsi1 = ct{9};
dth1 = ct{10};
dth2 = ct{11};
dx = ct{12};
dy = ct{13};
dz = ct{14};
t10 = ct{15};
t1005 = ct{16};
t1006 = ct{17};
t1007 = ct{18};
t1008 = ct{19};
t1009 = ct{20};
t1013 = ct{21};
t1016 = ct{22};
t1017 = ct{23};
t1018 = ct{24};
t1019 = ct{25};
t1023 = ct{26};
t1029 = ct{27};
t103 = ct{28};
t1037 = ct{29};
t1047 = ct{30};
t105 = ct{31};
t1050 = ct{32};
t1053 = ct{33};
t1059 = ct{34};
t1060 = ct{35};
t1064 = ct{36};
t1071 = ct{37};
t1072 = ct{38};
t1075 = ct{39};
t1077 = ct{40};
t1078 = ct{41};
t1079 = ct{42};
t1084 = ct{43};
t1086 = ct{44};
t1088 = ct{45};
t1097 = ct{46};
t1099 = ct{47};
t11 = ct{48};
t1102 = ct{49};
t1108 = ct{50};
t1113 = ct{51};
t1121 = ct{52};
t1129 = ct{53};
t1133 = ct{54};
t1135 = ct{55};
t1137 = ct{56};
t1138 = ct{57};
t1139 = ct{58};
t1141 = ct{59};
t1142 = ct{60};
t1143 = ct{61};
t1147 = ct{62};
t1149 = ct{63};
t1153 = ct{64};
t1155 = ct{65};
t1157 = ct{66};
t1159 = ct{67};
t1160 = ct{68};
t1164 = ct{69};
t1167 = ct{70};
t1169 = ct{71};
t1170 = ct{72};
t1173 = ct{73};
t1176 = ct{74};
t1178 = ct{75};
t1179 = ct{76};
t1181 = ct{77};
t1185 = ct{78};
t1186 = ct{79};
t1189 = ct{80};
t1193 = ct{81};
t1194 = ct{82};
t1195 = ct{83};
t1196 = ct{84};
t120 = ct{85};
t1200 = ct{86};
t1203 = ct{87};
t1205 = ct{88};
t1206 = ct{89};
t1211 = ct{90};
t1215 = ct{91};
t1221 = ct{92};
t1223 = ct{93};
t1224 = ct{94};
t1225 = ct{95};
t1228 = ct{96};
t1229 = ct{97};
t1230 = ct{98};
t1234 = ct{99};
t1240 = ct{100};
t1242 = ct{101};
t1245 = ct{102};
t1246 = ct{103};
t1247 = ct{104};
t1250 = ct{105};
t1252 = ct{106};
t1253 = ct{107};
t1255 = ct{108};
t1260 = ct{109};
t1261 = ct{110};
t1262 = ct{111};
t1264 = ct{112};
t1265 = ct{113};
t1268 = ct{114};
t1280 = ct{115};
t1283 = ct{116};
t1291 = ct{117};
t130 = ct{118};
t1301 = ct{119};
t1302 = ct{120};
t1303 = ct{121};
t1304 = ct{122};
t1305 = ct{123};
t1307 = ct{124};
t1309 = ct{125};
t1322 = ct{126};
t1328 = ct{127};
t1331 = ct{128};
t1332 = ct{129};
t1334 = ct{130};
t1337 = ct{131};
t1338 = ct{132};
t134 = ct{133};
t1343 = ct{134};
t1344 = ct{135};
t1345 = ct{136};
t1348 = ct{137};
t1352 = ct{138};
t1354 = ct{139};
t1355 = ct{140};
t1360 = ct{141};
t1362 = ct{142};
t1365 = ct{143};
t1366 = ct{144};
t1368 = ct{145};
t1370 = ct{146};
t1371 = ct{147};
t1373 = ct{148};
t1374 = ct{149};
t1378 = ct{150};
t1381 = ct{151};
t1382 = ct{152};
t1384 = ct{153};
t1386 = ct{154};
t1388 = ct{155};
t1389 = ct{156};
t1391 = ct{157};
t1393 = ct{158};
t1394 = ct{159};
t1395 = ct{160};
t1396 = ct{161};
t1397 = ct{162};
t1406 = ct{163};
t1412 = ct{164};
t1413 = ct{165};
t1415 = ct{166};
t1421 = ct{167};
t1426 = ct{168};
t1427 = ct{169};
t1430 = ct{170};
t1431 = ct{171};
t1433 = ct{172};
t1435 = ct{173};
t144 = ct{174};
t1441 = ct{175};
t1443 = ct{176};
t1444 = ct{177};
t1446 = ct{178};
t1453 = ct{179};
t1455 = ct{180};
t1456 = ct{181};
t1457 = ct{182};
t1458 = ct{183};
t1460 = ct{184};
t1465 = ct{185};
t1466 = ct{186};
t1468 = ct{187};
t1470 = ct{188};
t1476 = ct{189};
t1481 = ct{190};
t1486 = ct{191};
t1487 = ct{192};
t1495 = ct{193};
t15 = ct{194};
t1505 = ct{195};
t1506 = ct{196};
t1508 = ct{197};
t1510 = ct{198};
t1512 = ct{199};
t1513 = ct{200};
t1518 = ct{201};
t1521 = ct{202};
t1525 = ct{203};
t1526 = ct{204};
t1528 = ct{205};
t1529 = ct{206};
t1531 = ct{207};
t1535 = ct{208};
t1540 = ct{209};
t1543 = ct{210};
t1544 = ct{211};
t1552 = ct{212};
t1558 = ct{213};
t1562 = ct{214};
t1568 = ct{215};
t1575 = ct{216};
t1578 = ct{217};
t1581 = ct{218};
t1586 = ct{219};
t1593 = ct{220};
t1596 = ct{221};
t1597 = ct{222};
t1598 = ct{223};
t1609 = ct{224};
t161 = ct{225};
t1612 = ct{226};
t1618 = ct{227};
t1619 = ct{228};
t162 = ct{229};
t1620 = ct{230};
t1621 = ct{231};
t1624 = ct{232};
t1627 = ct{233};
t1628 = ct{234};
t1633 = ct{235};
t1634 = ct{236};
t1635 = ct{237};
t1637 = ct{238};
t1639 = ct{239};
t1640 = ct{240};
t1645 = ct{241};
t1646 = ct{242};
t1651 = ct{243};
t1652 = ct{244};
t1654 = ct{245};
t1655 = ct{246};
t1656 = ct{247};
t1657 = ct{248};
t1659 = ct{249};
t1660 = ct{250};
t1661 = ct{251};
t1664 = ct{252};
t1665 = ct{253};
t1667 = ct{254};
t1672 = ct{255};
t1674 = ct{256};
t1676 = ct{257};
t1678 = ct{258};
t1680 = ct{259};
t1681 = ct{260};
t1682 = ct{261};
t1683 = ct{262};
t1685 = ct{263};
t1692 = ct{264};
t1693 = ct{265};
t1694 = ct{266};
t1695 = ct{267};
t1698 = ct{268};
t1701 = ct{269};
t1702 = ct{270};
t1703 = ct{271};
t1705 = ct{272};
t1706 = ct{273};
t1716 = ct{274};
t1718 = ct{275};
t1719 = ct{276};
t1720 = ct{277};
t1721 = ct{278};
t1722 = ct{279};
t1725 = ct{280};
t1727 = ct{281};
t1730 = ct{282};
t1734 = ct{283};
t1735 = ct{284};
t1736 = ct{285};
t1737 = ct{286};
t1739 = ct{287};
t1741 = ct{288};
t1742 = ct{289};
t1746 = ct{290};
t1747 = ct{291};
t1748 = ct{292};
t1751 = ct{293};
t1752 = ct{294};
t1759 = ct{295};
t1761 = ct{296};
t1763 = ct{297};
t1764 = ct{298};
t1771 = ct{299};
t1774 = ct{300};
t1777 = ct{301};
t1778 = ct{302};
t1779 = ct{303};
t1781 = ct{304};
t1784 = ct{305};
t1785 = ct{306};
t1786 = ct{307};
t1787 = ct{308};
t1788 = ct{309};
t1789 = ct{310};
t1790 = ct{311};
t1792 = ct{312};
t1799 = ct{313};
t1800 = ct{314};
t1801 = ct{315};
t1802 = ct{316};
t1806 = ct{317};
t1809 = ct{318};
t1810 = ct{319};
t1813 = ct{320};
t1832 = ct{321};
t1836 = ct{322};
t1840 = ct{323};
t1843 = ct{324};
t1846 = ct{325};
t1851 = ct{326};
t1853 = ct{327};
t1855 = ct{328};
t1857 = ct{329};
t1858 = ct{330};
t1859 = ct{331};
t1860 = ct{332};
t1865 = ct{333};
t1866 = ct{334};
t1867 = ct{335};
t1882 = ct{336};
t1883 = ct{337};
t1888 = ct{338};
t1890 = ct{339};
t1896 = ct{340};
t1898 = ct{341};
t1899 = ct{342};
t1900 = ct{343};
t1907 = ct{344};
t1910 = ct{345};
t1915 = ct{346};
t1917 = ct{347};
t1918 = ct{348};
t1928 = ct{349};
t1929 = ct{350};
t1932 = ct{351};
t1938 = ct{352};
t1939 = ct{353};
t1942 = ct{354};
t1943 = ct{355};
t1945 = ct{356};
t195 = ct{357};
t1950 = ct{358};
t1952 = ct{359};
t1956 = ct{360};
t1957 = ct{361};
t1959 = ct{362};
t1962 = ct{363};
t1964 = ct{364};
t1965 = ct{365};
t197 = ct{366};
t1970 = ct{367};
t1971 = ct{368};
t1974 = ct{369};
t1976 = ct{370};
t1977 = ct{371};
t1979 = ct{372};
t1981 = ct{373};
t1982 = ct{374};
t1983 = ct{375};
t1993 = ct{376};
t1997 = ct{377};
t1999 = ct{378};
t2 = ct{379};
t2000 = ct{380};
t2002 = ct{381};
t2004 = ct{382};
t2007 = ct{383};
t2008 = ct{384};
t2009 = ct{385};
t2012 = ct{386};
t2013 = ct{387};
t2015 = ct{388};
t2016 = ct{389};
t2018 = ct{390};
t2020 = ct{391};
t2023 = ct{392};
t2024 = ct{393};
t2032 = ct{394};
t2037 = ct{395};
t2038 = ct{396};
t2047 = ct{397};
t2049 = ct{398};
t2050 = ct{399};
t2057 = ct{400};
t2058 = ct{401};
t2059 = ct{402};
t2061 = ct{403};
t2062 = ct{404};
t2064 = ct{405};
t2065 = ct{406};
t2067 = ct{407};
t2068 = ct{408};
t2069 = ct{409};
t2072 = ct{410};
t2075 = ct{411};
t2076 = ct{412};
t2081 = ct{413};
t2082 = ct{414};
t2083 = ct{415};
t2086 = ct{416};
t2087 = ct{417};
t2088 = ct{418};
t2096 = ct{419};
t2104 = ct{420};
t2106 = ct{421};
t2107 = ct{422};
t2108 = ct{423};
t2110 = ct{424};
t2111 = ct{425};
t2113 = ct{426};
t2117 = ct{427};
t2119 = ct{428};
t2123 = ct{429};
t2130 = ct{430};
t2131 = ct{431};
t2134 = ct{432};
t2135 = ct{433};
t2137 = ct{434};
t2139 = ct{435};
t214 = ct{436};
t2141 = ct{437};
t2147 = ct{438};
t2148 = ct{439};
t2150 = ct{440};
t2152 = ct{441};
t2153 = ct{442};
t2155 = ct{443};
t2156 = ct{444};
t2158 = ct{445};
t2161 = ct{446};
t2174 = ct{447};
t2175 = ct{448};
t2178 = ct{449};
t2183 = ct{450};
t2186 = ct{451};
t2188 = ct{452};
t2189 = ct{453};
t2190 = ct{454};
t2191 = ct{455};
t2192 = ct{456};
t2196 = ct{457};
t2197 = ct{458};
t2202 = ct{459};
t2203 = ct{460};
t2206 = ct{461};
t2208 = ct{462};
t2210 = ct{463};
t2212 = ct{464};
t2215 = ct{465};
t2218 = ct{466};
t2220 = ct{467};
t2222 = ct{468};
t2223 = ct{469};
t2225 = ct{470};
t2227 = ct{471};
t2237 = ct{472};
t2240 = ct{473};
t2241 = ct{474};
t2242 = ct{475};
t2243 = ct{476};
t2247 = ct{477};
t2248 = ct{478};
t2249 = ct{479};
t2254 = ct{480};
t2255 = ct{481};
t2257 = ct{482};
t2259 = ct{483};
t2260 = ct{484};
t2263 = ct{485};
t2268 = ct{486};
t2269 = ct{487};
t2271 = ct{488};
t2274 = ct{489};
t2276 = ct{490};
t2281 = ct{491};
t2282 = ct{492};
t2285 = ct{493};
t2286 = ct{494};
t2287 = ct{495};
t2289 = ct{496};
t2293 = ct{497};
t2305 = ct{498};
t2308 = ct{499};
t2312 = ct{500};
t2316 = ct{501};
t2317 = ct{502};
t2319 = ct{503};
t2322 = ct{504};
t2325 = ct{505};
t2329 = ct{506};
t2334 = ct{507};
t2336 = ct{508};
t2338 = ct{509};
t2339 = ct{510};
t2341 = ct{511};
t2342 = ct{512};
t2343 = ct{513};
t2345 = ct{514};
t2347 = ct{515};
t2348 = ct{516};
t2352 = ct{517};
t2358 = ct{518};
t2360 = ct{519};
t2361 = ct{520};
t2364 = ct{521};
t2368 = ct{522};
t2376 = ct{523};
t2387 = ct{524};
t2388 = ct{525};
t2389 = ct{526};
t2390 = ct{527};
t2391 = ct{528};
t2397 = ct{529};
t2399 = ct{530};
t24 = ct{531};
t2401 = ct{532};
t2404 = ct{533};
t2406 = ct{534};
t2409 = ct{535};
t2410 = ct{536};
t2411 = ct{537};
t2412 = ct{538};
t2413 = ct{539};
t2419 = ct{540};
t2420 = ct{541};
t2426 = ct{542};
t2427 = ct{543};
t2429 = ct{544};
t2430 = ct{545};
t2434 = ct{546};
t2435 = ct{547};
t2436 = ct{548};
t2438 = ct{549};
t2447 = ct{550};
t2449 = ct{551};
t2458 = ct{552};
t2463 = ct{553};
t2465 = ct{554};
t2468 = ct{555};
t2471 = ct{556};
t2472 = ct{557};
t2479 = ct{558};
t2483 = ct{559};
t2485 = ct{560};
t2487 = ct{561};
t2489 = ct{562};
t2492 = ct{563};
t2495 = ct{564};
t2496 = ct{565};
t25 = ct{566};
t2501 = ct{567};
t2503 = ct{568};
t2504 = ct{569};
t2512 = ct{570};
t2514 = ct{571};
t2515 = ct{572};
t2516 = ct{573};
t2518 = ct{574};
t2522 = ct{575};
t2523 = ct{576};
t2524 = ct{577};
t2526 = ct{578};
t2527 = ct{579};
t2528 = ct{580};
t2535 = ct{581};
t2536 = ct{582};
t2543 = ct{583};
t2547 = ct{584};
t2563 = ct{585};
t2564 = ct{586};
t2567 = ct{587};
t2568 = ct{588};
t2569 = ct{589};
t2571 = ct{590};
t2573 = ct{591};
t2574 = ct{592};
t2576 = ct{593};
t2578 = ct{594};
t2579 = ct{595};
t2581 = ct{596};
t2582 = ct{597};
t2587 = ct{598};
t2589 = ct{599};
t259 = ct{600};
t2590 = ct{601};
t2591 = ct{602};
t2597 = ct{603};
t2599 = ct{604};
t26 = ct{605};
t260 = ct{606};
t2600 = ct{607};
t2605 = ct{608};
t2613 = ct{609};
t2616 = ct{610};
t2617 = ct{611};
t2621 = ct{612};
t2624 = ct{613};
t2627 = ct{614};
t2632 = ct{615};
t2636 = ct{616};
t2637 = ct{617};
t2638 = ct{618};
t2646 = ct{619};
t2648 = ct{620};
t2657 = ct{621};
t2660 = ct{622};
t2662 = ct{623};
t2663 = ct{624};
t2665 = ct{625};
t2667 = ct{626};
t2668 = ct{627};
t2669 = ct{628};
t2673 = ct{629};
t2679 = ct{630};
t2684 = ct{631};
t2688 = ct{632};
t2692 = ct{633};
t2696 = ct{634};
t2698 = ct{635};
t2699 = ct{636};
t27 = ct{637};
t2700 = ct{638};
t2706 = ct{639};
t2707 = ct{640};
t2708 = ct{641};
t2710 = ct{642};
t2712 = ct{643};
t2715 = ct{644};
t2717 = ct{645};
t2718 = ct{646};
t2722 = ct{647};
t2723 = ct{648};
t2728 = ct{649};
t2730 = ct{650};
t2733 = ct{651};
t2734 = ct{652};
t2735 = ct{653};
t2736 = ct{654};
t2737 = ct{655};
t2738 = ct{656};
t2743 = ct{657};
t2744 = ct{658};
t2746 = ct{659};
t2750 = ct{660};
t2754 = ct{661};
t2759 = ct{662};
t276 = ct{663};
t2763 = ct{664};
t277 = ct{665};
t2778 = ct{666};
t2783 = ct{667};
t2785 = ct{668};
t2787 = ct{669};
t2790 = ct{670};
t2791 = ct{671};
t2792 = ct{672};
t2794 = ct{673};
t2796 = ct{674};
t2797 = ct{675};
t2798 = ct{676};
t2799 = ct{677};
t2803 = ct{678};
t2805 = ct{679};
t2811 = ct{680};
t2816 = ct{681};
t2817 = ct{682};
t2818 = ct{683};
t2819 = ct{684};
t2821 = ct{685};
t2823 = ct{686};
t2824 = ct{687};
t2825 = ct{688};
t2829 = ct{689};
t283 = ct{690};
t2831 = ct{691};
t2833 = ct{692};
t2834 = ct{693};
t2836 = ct{694};
t2839 = ct{695};
t284 = ct{696};
t2842 = ct{697};
t2843 = ct{698};
t2844 = ct{699};
t2845 = ct{700};
t2847 = ct{701};
t2849 = ct{702};
t285 = ct{703};
t2853 = ct{704};
t286 = ct{705};
t2860 = ct{706};
t2861 = ct{707};
t2868 = ct{708};
t287 = ct{709};
t2871 = ct{710};
t2875 = ct{711};
t2876 = ct{712};
t2877 = ct{713};
t2878 = ct{714};
t2879 = ct{715};
t288 = ct{716};
t2882 = ct{717};
t2883 = ct{718};
t2884 = ct{719};
t2887 = ct{720};
t2889 = ct{721};
t289 = ct{722};
t2899 = ct{723};
t290 = ct{724};
t291 = ct{725};
t2912 = ct{726};
t2913 = ct{727};
t2914 = ct{728};
t2915 = ct{729};
t2917 = ct{730};
t2918 = ct{731};
t292 = ct{732};
t2920 = ct{733};
t2921 = ct{734};
t2927 = ct{735};
t2928 = ct{736};
t293 = ct{737};
t2930 = ct{738};
t2936 = ct{739};
t2937 = ct{740};
t294 = ct{741};
t2942 = ct{742};
t2944 = ct{743};
t2945 = ct{744};
t2950 = ct{745};
t2952 = ct{746};
t2954 = ct{747};
t2956 = ct{748};
t2962 = ct{749};
t2963 = ct{750};
t2965 = ct{751};
t2970 = ct{752};
t2972 = ct{753};
t2977 = ct{754};
t2978 = ct{755};
t2981 = ct{756};
t2982 = ct{757};
t2989 = ct{758};
t2994 = ct{759};
t2996 = ct{760};
t2997 = ct{761};
t3 = ct{762};
t3008 = ct{763};
t3009 = ct{764};
t3012 = ct{765};
t3022 = ct{766};
t3027 = ct{767};
t3030 = ct{768};
t3031 = ct{769};
t3034 = ct{770};
t3035 = ct{771};
t3038 = ct{772};
t304 = ct{773};
t3040 = ct{774};
t3050 = ct{775};
t3054 = ct{776};
t3059 = ct{777};
t3062 = ct{778};
t3063 = ct{779};
t3064 = ct{780};
t3070 = ct{781};
t3076 = ct{782};
t3080 = ct{783};
t3082 = ct{784};
t3084 = ct{785};
t3085 = ct{786};
t3086 = ct{787};
t3087 = ct{788};
t3089 = ct{789};
t3090 = ct{790};
t3091 = ct{791};
t3093 = ct{792};
t3094 = ct{793};
t3096 = ct{794};
t3105 = ct{795};
t3106 = ct{796};
t3107 = ct{797};
t3109 = ct{798};
t3110 = ct{799};
t3113 = ct{800};
t3117 = ct{801};
t3121 = ct{802};
t3122 = ct{803};
t3127 = ct{804};
t3131 = ct{805};
t3138 = ct{806};
t3139 = ct{807};
t3146 = ct{808};
t3147 = ct{809};
t3149 = ct{810};
t3151 = ct{811};
t3155 = ct{812};
t3160 = ct{813};
t3161 = ct{814};
t3167 = ct{815};
t3169 = ct{816};
t3170 = ct{817};
t3171 = ct{818};
t3173 = ct{819};
t3176 = ct{820};
t3177 = ct{821};
t3178 = ct{822};
t3179 = ct{823};
t3180 = ct{824};
t3186 = ct{825};
t3187 = ct{826};
t3190 = ct{827};
t3192 = ct{828};
t3193 = ct{829};
t3199 = ct{830};
t3204 = ct{831};
t3206 = ct{832};
t3207 = ct{833};
t3210 = ct{834};
t3212 = ct{835};
t3213 = ct{836};
t3214 = ct{837};
t3216 = ct{838};
t3217 = ct{839};
t3222 = ct{840};
t3230 = ct{841};
t3232 = ct{842};
t3233 = ct{843};
t3235 = ct{844};
t3236 = ct{845};
t3243 = ct{846};
t3244 = ct{847};
t3247 = ct{848};
t3248 = ct{849};
t3252 = ct{850};
t3256 = ct{851};
t3257 = ct{852};
t3261 = ct{853};
t3262 = ct{854};
t3263 = ct{855};
t3265 = ct{856};
t3266 = ct{857};
t3267 = ct{858};
t3270 = ct{859};
t3272 = ct{860};
t3273 = ct{861};
t3276 = ct{862};
t3277 = ct{863};
t3278 = ct{864};
t3284 = ct{865};
t3286 = ct{866};
t3287 = ct{867};
t3289 = ct{868};
t3299 = ct{869};
t3302 = ct{870};
t3304 = ct{871};
t3307 = ct{872};
t3308 = ct{873};
t3311 = ct{874};
t3312 = ct{875};
t3315 = ct{876};
t3320 = ct{877};
t3321 = ct{878};
t3322 = ct{879};
t3325 = ct{880};
t3326 = ct{881};
t3328 = ct{882};
t3329 = ct{883};
t3330 = ct{884};
t3331 = ct{885};
t3333 = ct{886};
t3335 = ct{887};
t3336 = ct{888};
t3339 = ct{889};
t3341 = ct{890};
t3343 = ct{891};
t3344 = ct{892};
t3347 = ct{893};
t3351 = ct{894};
t3354 = ct{895};
t3357 = ct{896};
t3359 = ct{897};
t3376 = ct{898};
t3378 = ct{899};
t3379 = ct{900};
t3380 = ct{901};
t3381 = ct{902};
t3385 = ct{903};
t3387 = ct{904};
t3390 = ct{905};
t3391 = ct{906};
t3392 = ct{907};
t3397 = ct{908};
t3402 = ct{909};
t3403 = ct{910};
t3406 = ct{911};
t3407 = ct{912};
t3411 = ct{913};
t3412 = ct{914};
t3413 = ct{915};
t3414 = ct{916};
t3415 = ct{917};
t3416 = ct{918};
t3419 = ct{919};
t3423 = ct{920};
t3424 = ct{921};
t3427 = ct{922};
t3429 = ct{923};
t3431 = ct{924};
t3432 = ct{925};
t3433 = ct{926};
t3437 = ct{927};
t3438 = ct{928};
t3439 = ct{929};
t3441 = ct{930};
t3442 = ct{931};
t3445 = ct{932};
t3448 = ct{933};
t3449 = ct{934};
t3458 = ct{935};
t3459 = ct{936};
t3460 = ct{937};
t3463 = ct{938};
t3467 = ct{939};
t3471 = ct{940};
t3473 = ct{941};
t3475 = ct{942};
t3476 = ct{943};
t3480 = ct{944};
t3481 = ct{945};
t3482 = ct{946};
t3483 = ct{947};
t3485 = ct{948};
t3486 = ct{949};
t3487 = ct{950};
t3489 = ct{951};
t3490 = ct{952};
t3494 = ct{953};
t3499 = ct{954};
t3501 = ct{955};
t3504 = ct{956};
t3506 = ct{957};
t3510 = ct{958};
t3512 = ct{959};
t3516 = ct{960};
t3521 = ct{961};
t3522 = ct{962};
t3523 = ct{963};
t3524 = ct{964};
t3526 = ct{965};
t3528 = ct{966};
t3529 = ct{967};
t3530 = ct{968};
t3531 = ct{969};
t3534 = ct{970};
t3540 = ct{971};
t3541 = ct{972};
t3543 = ct{973};
t3544 = ct{974};
t3545 = ct{975};
t3548 = ct{976};
t3550 = ct{977};
t3552 = ct{978};
t3553 = ct{979};
t3554 = ct{980};
t3556 = ct{981};
t3557 = ct{982};
t3563 = ct{983};
t3570 = ct{984};
t3571 = ct{985};
t3575 = ct{986};
t3576 = ct{987};
t3578 = ct{988};
t3582 = ct{989};
t3583 = ct{990};
t3584 = ct{991};
t3587 = ct{992};
t3594 = ct{993};
t3597 = ct{994};
t3598 = ct{995};
t3600 = ct{996};
t3602 = ct{997};
t3609 = ct{998};
t3614 = ct{999};
t3617 = ct{1000};
t3619 = ct{1001};
t3621 = ct{1002};
t3627 = ct{1003};
t3632 = ct{1004};
t3634 = ct{1005};
t3638 = ct{1006};
t3644 = ct{1007};
t3647 = ct{1008};
t3648 = ct{1009};
t3649 = ct{1010};
t3651 = ct{1011};
t3652 = ct{1012};
t3657 = ct{1013};
t3659 = ct{1014};
t3661 = ct{1015};
t3667 = ct{1016};
t3668 = ct{1017};
t3671 = ct{1018};
t3672 = ct{1019};
t3678 = ct{1020};
t3679 = ct{1021};
t3680 = ct{1022};
t3681 = ct{1023};
t3682 = ct{1024};
t3683 = ct{1025};
t3684 = ct{1026};
t3685 = ct{1027};
t3686 = ct{1028};
t3687 = ct{1029};
t3689 = ct{1030};
t3697 = ct{1031};
t3698 = ct{1032};
t3701 = ct{1033};
t3702 = ct{1034};
t3704 = ct{1035};
t3709 = ct{1036};
t3710 = ct{1037};
t3711 = ct{1038};
t3716 = ct{1039};
t3719 = ct{1040};
t3720 = ct{1041};
t3721 = ct{1042};
t3722 = ct{1043};
t3723 = ct{1044};
t3724 = ct{1045};
t3730 = ct{1046};
t3735 = ct{1047};
t3738 = ct{1048};
t3739 = ct{1049};
t3742 = ct{1050};
t3744 = ct{1051};
t3745 = ct{1052};
t3746 = ct{1053};
t3748 = ct{1054};
t3749 = ct{1055};
t3750 = ct{1056};
t3755 = ct{1057};
t3756 = ct{1058};
t3757 = ct{1059};
t3758 = ct{1060};
t3759 = ct{1061};
t376 = ct{1062};
t3764 = ct{1063};
t3766 = ct{1064};
t3769 = ct{1065};
t377 = ct{1066};
t3770 = ct{1067};
t3771 = ct{1068};
t3772 = ct{1069};
t3773 = ct{1070};
t3774 = ct{1071};
t3777 = ct{1072};
t3779 = ct{1073};
t3780 = ct{1074};
t3784 = ct{1075};
t3787 = ct{1076};
t3791 = ct{1077};
t3792 = ct{1078};
t3793 = ct{1079};
t3794 = ct{1080};
t3797 = ct{1081};
t3798 = ct{1082};
t3802 = ct{1083};
t3804 = ct{1084};
t3805 = ct{1085};
t3808 = ct{1086};
t381 = ct{1087};
t3811 = ct{1088};
t3812 = ct{1089};
t3814 = ct{1090};
t3815 = ct{1091};
t3817 = ct{1092};
t382 = ct{1093};
t3820 = ct{1094};
t3823 = ct{1095};
t3825 = ct{1096};
t3827 = ct{1097};
t3828 = ct{1098};
t383 = ct{1099};
t3832 = ct{1100};
t3834 = ct{1101};
t3836 = ct{1102};
t3837 = ct{1103};
t3838 = ct{1104};
t3841 = ct{1105};
t3845 = ct{1106};
t3847 = ct{1107};
t3848 = ct{1108};
t3849 = ct{1109};
t3851 = ct{1110};
t3855 = ct{1111};
t3856 = ct{1112};
t3858 = ct{1113};
t3859 = ct{1114};
t3862 = ct{1115};
t3867 = ct{1116};
t3868 = ct{1117};
t3870 = ct{1118};
t3871 = ct{1119};
t3879 = ct{1120};
t3880 = ct{1121};
t3882 = ct{1122};
t3883 = ct{1123};
t3885 = ct{1124};
t3887 = ct{1125};
t3889 = ct{1126};
t3893 = ct{1127};
t3895 = ct{1128};
t3896 = ct{1129};
t3898 = ct{1130};
t390 = ct{1131};
t3900 = ct{1132};
t3902 = ct{1133};
t3903 = ct{1134};
t3906 = ct{1135};
t3907 = ct{1136};
t3908 = ct{1137};
t3909 = ct{1138};
t3912 = ct{1139};
t3915 = ct{1140};
t3916 = ct{1141};
t3918 = ct{1142};
t3920 = ct{1143};
t3921 = ct{1144};
t3923 = ct{1145};
t3925 = ct{1146};
t3926 = ct{1147};
t3928 = ct{1148};
t3929 = ct{1149};
t3930 = ct{1150};
t3931 = ct{1151};
t3932 = ct{1152};
t3933 = ct{1153};
t3934 = ct{1154};
t3936 = ct{1155};
t3937 = ct{1156};
t3938 = ct{1157};
t3939 = ct{1158};
t394 = ct{1159};
t3940 = ct{1160};
t3943 = ct{1161};
t3944 = ct{1162};
t3945 = ct{1163};
t3947 = ct{1164};
t3948 = ct{1165};
t3949 = ct{1166};
t3950 = ct{1167};
t3951 = ct{1168};
t3952 = ct{1169};
t3953 = ct{1170};
t3954 = ct{1171};
t3955 = ct{1172};
t3956 = ct{1173};
t3957 = ct{1174};
t3958 = ct{1175};
t3959 = ct{1176};
t3960 = ct{1177};
t3961 = ct{1178};
t3962 = ct{1179};
t3964 = ct{1180};
t3965 = ct{1181};
t3966 = ct{1182};
t3967 = ct{1183};
t3969 = ct{1184};
t3971 = ct{1185};
t3972 = ct{1186};
t3973 = ct{1187};
t3974 = ct{1188};
t3975 = ct{1189};
t3976 = ct{1190};
t3977 = ct{1191};
t3979 = ct{1192};
t3980 = ct{1193};
t3981 = ct{1194};
t3982 = ct{1195};
t3983 = ct{1196};
t3984 = ct{1197};
t3985 = ct{1198};
t3986 = ct{1199};
t3992 = ct{1200};
t3993 = ct{1201};
t3995 = ct{1202};
t3996 = ct{1203};
t3998 = ct{1204};
t4 = ct{1205};
t4000 = ct{1206};
t4001 = ct{1207};
t4003 = ct{1208};
t4005 = ct{1209};
t4006 = ct{1210};
t4007 = ct{1211};
t4008 = ct{1212};
t4009 = ct{1213};
t4010 = ct{1214};
t4012 = ct{1215};
t4014 = ct{1216};
t4017 = ct{1217};
t4018 = ct{1218};
t4019 = ct{1219};
t4020 = ct{1220};
t4022 = ct{1221};
t4023 = ct{1222};
t4024 = ct{1223};
t4025 = ct{1224};
t4026 = ct{1225};
t4027 = ct{1226};
t4028 = ct{1227};
t4029 = ct{1228};
t4033 = ct{1229};
t4034 = ct{1230};
t4035 = ct{1231};
t4036 = ct{1232};
t4037 = ct{1233};
t4038 = ct{1234};
t4039 = ct{1235};
t4041 = ct{1236};
t4042 = ct{1237};
t4044 = ct{1238};
t4046 = ct{1239};
t4047 = ct{1240};
t4048 = ct{1241};
t4050 = ct{1242};
t4051 = ct{1243};
t4052 = ct{1244};
t4053 = ct{1245};
t4054 = ct{1246};
t4056 = ct{1247};
t4058 = ct{1248};
t4059 = ct{1249};
t4061 = ct{1250};
t4062 = ct{1251};
t4064 = ct{1252};
t4065 = ct{1253};
t4066 = ct{1254};
t4068 = ct{1255};
t4070 = ct{1256};
t4071 = ct{1257};
t4072 = ct{1258};
t4073 = ct{1259};
t4074 = ct{1260};
t4077 = ct{1261};
t4078 = ct{1262};
t4081 = ct{1263};
t4083 = ct{1264};
t4084 = ct{1265};
t4085 = ct{1266};
t4086 = ct{1267};
t4087 = ct{1268};
t4089 = ct{1269};
t4090 = ct{1270};
t4091 = ct{1271};
t4092 = ct{1272};
t4094 = ct{1273};
t4095 = ct{1274};
t4096 = ct{1275};
t4097 = ct{1276};
t4098 = ct{1277};
t4099 = ct{1278};
t410 = ct{1279};
t4100 = ct{1280};
t4104 = ct{1281};
t4105 = ct{1282};
t4107 = ct{1283};
t4108 = ct{1284};
t4109 = ct{1285};
t411 = ct{1286};
t4111 = ct{1287};
t4112 = ct{1288};
t4115 = ct{1289};
t4116 = ct{1290};
t4117 = ct{1291};
t4119 = ct{1292};
t412 = ct{1293};
t4120 = ct{1294};
t4121 = ct{1295};
t4122 = ct{1296};
t4126 = ct{1297};
t4127 = ct{1298};
t4129 = ct{1299};
t413 = ct{1300};
t4132 = ct{1301};
t4133 = ct{1302};
t4135 = ct{1303};
t4137 = ct{1304};
t4138 = ct{1305};
t4139 = ct{1306};
t414 = ct{1307};
t4140 = ct{1308};
t4141 = ct{1309};
t4143 = ct{1310};
t4144 = ct{1311};
t4145 = ct{1312};
t4147 = ct{1313};
t415 = ct{1314};
t4152 = ct{1315};
t4153 = ct{1316};
t4154 = ct{1317};
t4155 = ct{1318};
t4156 = ct{1319};
t4157 = ct{1320};
t4160 = ct{1321};
t4162 = ct{1322};
t4164 = ct{1323};
t4165 = ct{1324};
t4169 = ct{1325};
t4170 = ct{1326};
t4171 = ct{1327};
t4173 = ct{1328};
t4174 = ct{1329};
t4179 = ct{1330};
t4182 = ct{1331};
t4183 = ct{1332};
t4184 = ct{1333};
t4186 = ct{1334};
t4187 = ct{1335};
t4188 = ct{1336};
t4189 = ct{1337};
t4190 = ct{1338};
t4195 = ct{1339};
t4196 = ct{1340};
t4197 = ct{1341};
t420 = ct{1342};
t4200 = ct{1343};
t4201 = ct{1344};
t4204 = ct{1345};
t4205 = ct{1346};
t4206 = ct{1347};
t4208 = ct{1348};
t4209 = ct{1349};
t421 = ct{1350};
t4210 = ct{1351};
t4211 = ct{1352};
t4212 = ct{1353};
t4213 = ct{1354};
t4214 = ct{1355};
t4215 = ct{1356};
t4216 = ct{1357};
t4217 = ct{1358};
t4218 = ct{1359};
t4219 = ct{1360};
t4220 = ct{1361};
t4221 = ct{1362};
t4222 = ct{1363};
t4223 = ct{1364};
t4224 = ct{1365};
t4225 = ct{1366};
t4226 = ct{1367};
t4227 = ct{1368};
t4228 = ct{1369};
t4231 = ct{1370};
t4232 = ct{1371};
t4233 = ct{1372};
t4234 = ct{1373};
t4236 = ct{1374};
t4237 = ct{1375};
t4238 = ct{1376};
t4239 = ct{1377};
t4240 = ct{1378};
t4241 = ct{1379};
t4243 = ct{1380};
t4244 = ct{1381};
t4245 = ct{1382};
t4246 = ct{1383};
t4247 = ct{1384};
t4248 = ct{1385};
t4249 = ct{1386};
t425 = ct{1387};
t4250 = ct{1388};
t4252 = ct{1389};
t4253 = ct{1390};
t4255 = ct{1391};
t4256 = ct{1392};
t4257 = ct{1393};
t4258 = ct{1394};
t4259 = ct{1395};
t4260 = ct{1396};
t4261 = ct{1397};
t4262 = ct{1398};
t4263 = ct{1399};
t4265 = ct{1400};
t4266 = ct{1401};
t4268 = ct{1402};
t4269 = ct{1403};
t4271 = ct{1404};
t4272 = ct{1405};
t4273 = ct{1406};
t4274 = ct{1407};
t4276 = ct{1408};
t4277 = ct{1409};
t4278 = ct{1410};
t4280 = ct{1411};
t4281 = ct{1412};
t4282 = ct{1413};
t4286 = ct{1414};
t4290 = ct{1415};
t4291 = ct{1416};
t4295 = ct{1417};
t4296 = ct{1418};
t430 = ct{1419};
t4300 = ct{1420};
t4301 = ct{1421};
t4302 = ct{1422};
t4303 = ct{1423};
t4304 = ct{1424};
t4305 = ct{1425};
t4307 = ct{1426};
t4308 = ct{1427};
t4309 = ct{1428};
t431 = ct{1429};
t4310 = ct{1430};
t4311 = ct{1431};
t4312 = ct{1432};
t4313 = ct{1433};
t4314 = ct{1434};
t4315 = ct{1435};
t4316 = ct{1436};
t4317 = ct{1437};
t4318 = ct{1438};
t4319 = ct{1439};
t4320 = ct{1440};
t4321 = ct{1441};
t4322 = ct{1442};
t4323 = ct{1443};
t4324 = ct{1444};
t4326 = ct{1445};
t4327 = ct{1446};
t4329 = ct{1447};
t433 = ct{1448};
t4330 = ct{1449};
t4331 = ct{1450};
t4332 = ct{1451};
t4333 = ct{1452};
t4334 = ct{1453};
t4337 = ct{1454};
t4339 = ct{1455};
t4340 = ct{1456};
t4341 = ct{1457};
t4342 = ct{1458};
t4343 = ct{1459};
t4344 = ct{1460};
t4345 = ct{1461};
t4346 = ct{1462};
t4348 = ct{1463};
t4349 = ct{1464};
t4350 = ct{1465};
t4352 = ct{1466};
t4354 = ct{1467};
t4355 = ct{1468};
t4356 = ct{1469};
t4357 = ct{1470};
t4358 = ct{1471};
t4359 = ct{1472};
t436 = ct{1473};
t4360 = ct{1474};
t4361 = ct{1475};
t4364 = ct{1476};
t4365 = ct{1477};
t4367 = ct{1478};
t4368 = ct{1479};
t4369 = ct{1480};
t4370 = ct{1481};
t4371 = ct{1482};
t4372 = ct{1483};
t4373 = ct{1484};
t4374 = ct{1485};
t4375 = ct{1486};
t4376 = ct{1487};
t4377 = ct{1488};
t4378 = ct{1489};
t4379 = ct{1490};
t4380 = ct{1491};
t4382 = ct{1492};
t4384 = ct{1493};
t4385 = ct{1494};
t4386 = ct{1495};
t4387 = ct{1496};
t4388 = ct{1497};
t4389 = ct{1498};
t4391 = ct{1499};
t4392 = ct{1500};
t4393 = ct{1501};
t4394 = ct{1502};
t4395 = ct{1503};
t4397 = ct{1504};
t4398 = ct{1505};
t4399 = ct{1506};
t44 = ct{1507};
t4400 = ct{1508};
t4401 = ct{1509};
t4402 = ct{1510};
t4403 = ct{1511};
t4404 = ct{1512};
t4405 = ct{1513};
t4406 = ct{1514};
t4407 = ct{1515};
t4408 = ct{1516};
t4409 = ct{1517};
t4411 = ct{1518};
t4412 = ct{1519};
t4413 = ct{1520};
t4414 = ct{1521};
t4415 = ct{1522};
t4416 = ct{1523};
t4417 = ct{1524};
t4418 = ct{1525};
t4419 = ct{1526};
t4420 = ct{1527};
t4421 = ct{1528};
t4422 = ct{1529};
t4424 = ct{1530};
t4425 = ct{1531};
t4427 = ct{1532};
t4428 = ct{1533};
t4429 = ct{1534};
t4431 = ct{1535};
t4432 = ct{1536};
t4433 = ct{1537};
t4434 = ct{1538};
t4435 = ct{1539};
t4437 = ct{1540};
t4438 = ct{1541};
t4439 = ct{1542};
t4440 = ct{1543};
t4442 = ct{1544};
t4443 = ct{1545};
t4444 = ct{1546};
t4447 = ct{1547};
t4448 = ct{1548};
t4449 = ct{1549};
t445 = ct{1550};
t4450 = ct{1551};
t4451 = ct{1552};
t4452 = ct{1553};
t4453 = ct{1554};
t4454 = ct{1555};
t4455 = ct{1556};
t4456 = ct{1557};
t4457 = ct{1558};
t4458 = ct{1559};
t4459 = ct{1560};
t4460 = ct{1561};
t4461 = ct{1562};
t4462 = ct{1563};
t4463 = ct{1564};
t4465 = ct{1565};
t4467 = ct{1566};
t4469 = ct{1567};
t4470 = ct{1568};
t4471 = ct{1569};
t4472 = ct{1570};
t4473 = ct{1571};
t4475 = ct{1572};
t4476 = ct{1573};
t4477 = ct{1574};
t4478 = ct{1575};
t4479 = ct{1576};
t4480 = ct{1577};
t4481 = ct{1578};
t4482 = ct{1579};
t4483 = ct{1580};
t4484 = ct{1581};
t4485 = ct{1582};
t4486 = ct{1583};
t4487 = ct{1584};
t4488 = ct{1585};
t4489 = ct{1586};
t4490 = ct{1587};
t4492 = ct{1588};
t4493 = ct{1589};
t4495 = ct{1590};
t4496 = ct{1591};
t4497 = ct{1592};
t4498 = ct{1593};
t4499 = ct{1594};
t4500 = ct{1595};
t4501 = ct{1596};
t4502 = ct{1597};
t4503 = ct{1598};
t4505 = ct{1599};
t4506 = ct{1600};
t4507 = ct{1601};
t451 = ct{1602};
t4510 = ct{1603};
t4511 = ct{1604};
t4512 = ct{1605};
t4514 = ct{1606};
t4515 = ct{1607};
t4517 = ct{1608};
t4518 = ct{1609};
t4519 = ct{1610};
t4520 = ct{1611};
t4521 = ct{1612};
t4522 = ct{1613};
t4523 = ct{1614};
t4524 = ct{1615};
t4525 = ct{1616};
t4526 = ct{1617};
t4528 = ct{1618};
t4529 = ct{1619};
t4530 = ct{1620};
t4531 = ct{1621};
t4532 = ct{1622};
t4533 = ct{1623};
t4534 = ct{1624};
t4535 = ct{1625};
t4536 = ct{1626};
t4537 = ct{1627};
t4538 = ct{1628};
t4540 = ct{1629};
t4541 = ct{1630};
t4542 = ct{1631};
t4544 = ct{1632};
t4545 = ct{1633};
t4546 = ct{1634};
t4547 = ct{1635};
t4549 = ct{1636};
t4550 = ct{1637};
t4551 = ct{1638};
t4552 = ct{1639};
t4553 = ct{1640};
t4554 = ct{1641};
t4555 = ct{1642};
t4556 = ct{1643};
t4557 = ct{1644};
t4558 = ct{1645};
t4559 = ct{1646};
t4560 = ct{1647};
t4561 = ct{1648};
t4562 = ct{1649};
t4563 = ct{1650};
t4565 = ct{1651};
t4566 = ct{1652};
t4567 = ct{1653};
t4568 = ct{1654};
t4570 = ct{1655};
t4571 = ct{1656};
t4572 = ct{1657};
t4573 = ct{1658};
t4574 = ct{1659};
t4575 = ct{1660};
t4576 = ct{1661};
t4577 = ct{1662};
t4578 = ct{1663};
t4579 = ct{1664};
t4580 = ct{1665};
t4581 = ct{1666};
t4582 = ct{1667};
t4583 = ct{1668};
t4584 = ct{1669};
t4585 = ct{1670};
t4586 = ct{1671};
t4588 = ct{1672};
t4589 = ct{1673};
t459 = ct{1674};
t4590 = ct{1675};
t4591 = ct{1676};
t4592 = ct{1677};
t4596 = ct{1678};
t4597 = ct{1679};
t4598 = ct{1680};
t4600 = ct{1681};
t4601 = ct{1682};
t4602 = ct{1683};
t4603 = ct{1684};
t4604 = ct{1685};
t4605 = ct{1686};
t4606 = ct{1687};
t4607 = ct{1688};
t4608 = ct{1689};
t4609 = ct{1690};
t4610 = ct{1691};
t4613 = ct{1692};
t4614 = ct{1693};
t4615 = ct{1694};
t4616 = ct{1695};
t4617 = ct{1696};
t4618 = ct{1697};
t4619 = ct{1698};
t4620 = ct{1699};
t4621 = ct{1700};
t4622 = ct{1701};
t4623 = ct{1702};
t4624 = ct{1703};
t4625 = ct{1704};
t4626 = ct{1705};
t4627 = ct{1706};
t4629 = ct{1707};
t4630 = ct{1708};
t4633 = ct{1709};
t4634 = ct{1710};
t4635 = ct{1711};
t4636 = ct{1712};
t4637 = ct{1713};
t4638 = ct{1714};
t4639 = ct{1715};
t4642 = ct{1716};
t4644 = ct{1717};
t4645 = ct{1718};
t4646 = ct{1719};
t4647 = ct{1720};
t4649 = ct{1721};
t465 = ct{1722};
t4651 = ct{1723};
t4652 = ct{1724};
t4655 = ct{1725};
t4656 = ct{1726};
t4657 = ct{1727};
t4658 = ct{1728};
t4659 = ct{1729};
t4660 = ct{1730};
t4661 = ct{1731};
t4662 = ct{1732};
t4663 = ct{1733};
t4664 = ct{1734};
t4665 = ct{1735};
t4666 = ct{1736};
t4667 = ct{1737};
t4668 = ct{1738};
t4669 = ct{1739};
t4672 = ct{1740};
t4673 = ct{1741};
t4674 = ct{1742};
t4675 = ct{1743};
t4678 = ct{1744};
t4679 = ct{1745};
t4680 = ct{1746};
t4681 = ct{1747};
t4682 = ct{1748};
t4684 = ct{1749};
t4685 = ct{1750};
t4686 = ct{1751};
t4688 = ct{1752};
t4689 = ct{1753};
t4690 = ct{1754};
t4693 = ct{1755};
t4694 = ct{1756};
t4695 = ct{1757};
t4696 = ct{1758};
t4697 = ct{1759};
t4698 = ct{1760};
t4700 = ct{1761};
t4701 = ct{1762};
t4702 = ct{1763};
t4704 = ct{1764};
t4705 = ct{1765};
t4706 = ct{1766};
t4707 = ct{1767};
t4708 = ct{1768};
t4709 = ct{1769};
t4710 = ct{1770};
t4711 = ct{1771};
t4712 = ct{1772};
t4713 = ct{1773};
t4722 = ct{1774};
t4723 = ct{1775};
t4724 = ct{1776};
t4727 = ct{1777};
t4729 = ct{1778};
t4732 = ct{1779};
t4733 = ct{1780};
t4735 = ct{1781};
t4736 = ct{1782};
t4737 = ct{1783};
t4738 = ct{1784};
t4742 = ct{1785};
t4746 = ct{1786};
t4749 = ct{1787};
t4750 = ct{1788};
t4751 = ct{1789};
t4752 = ct{1790};
t4753 = ct{1791};
t4754 = ct{1792};
t4755 = ct{1793};
t4756 = ct{1794};
t4758 = ct{1795};
t4759 = ct{1796};
t4761 = ct{1797};
t4764 = ct{1798};
t4765 = ct{1799};
t4766 = ct{1800};
t4769 = ct{1801};
t4770 = ct{1802};
t4771 = ct{1803};
t4772 = ct{1804};
t4773 = ct{1805};
t4775 = ct{1806};
t4776 = ct{1807};
t4780 = ct{1808};
t4783 = ct{1809};
t4784 = ct{1810};
t4785 = ct{1811};
t4786 = ct{1812};
t4787 = ct{1813};
t4788 = ct{1814};
t4789 = ct{1815};
t4790 = ct{1816};
t4791 = ct{1817};
t4792 = ct{1818};
t4793 = ct{1819};
t4796 = ct{1820};
t4799 = ct{1821};
t48 = ct{1822};
t4800 = ct{1823};
t4801 = ct{1824};
t4802 = ct{1825};
t4803 = ct{1826};
t4804 = ct{1827};
t4805 = ct{1828};
t4806 = ct{1829};
t4807 = ct{1830};
t4809 = ct{1831};
t4811 = ct{1832};
t4813 = ct{1833};
t4814 = ct{1834};
t4815 = ct{1835};
t4816 = ct{1836};
t4817 = ct{1837};
t4820 = ct{1838};
t4821 = ct{1839};
t4823 = ct{1840};
t4826 = ct{1841};
t4827 = ct{1842};
t4830 = ct{1843};
t4832 = ct{1844};
t4834 = ct{1845};
t4835 = ct{1846};
t4836 = ct{1847};
t4838 = ct{1848};
t4840 = ct{1849};
t4841 = ct{1850};
t4843 = ct{1851};
t4845 = ct{1852};
t4846 = ct{1853};
t4847 = ct{1854};
t4848 = ct{1855};
t4849 = ct{1856};
t485 = ct{1857};
t4850 = ct{1858};
t4851 = ct{1859};
t4852 = ct{1860};
t4853 = ct{1861};
t4857 = ct{1862};
t4858 = ct{1863};
t4861 = ct{1864};
t4862 = ct{1865};
t4863 = ct{1866};
t4864 = ct{1867};
t4865 = ct{1868};
t4867 = ct{1869};
t4870 = ct{1870};
t4871 = ct{1871};
t4873 = ct{1872};
t4874 = ct{1873};
t4877 = ct{1874};
t488 = ct{1875};
t4880 = ct{1876};
t4881 = ct{1877};
t4882 = ct{1878};
t4883 = ct{1879};
t4884 = ct{1880};
t4886 = ct{1881};
t4887 = ct{1882};
t4888 = ct{1883};
t4889 = ct{1884};
t4890 = ct{1885};
t4892 = ct{1886};
t4895 = ct{1887};
t4897 = ct{1888};
t4899 = ct{1889};
t49 = ct{1890};
t4900 = ct{1891};
t4901 = ct{1892};
t4904 = ct{1893};
t4906 = ct{1894};
t4907 = ct{1895};
t4908 = ct{1896};
t4909 = ct{1897};
t4911 = ct{1898};
t4912 = ct{1899};
t4913 = ct{1900};
t4914 = ct{1901};
t4916 = ct{1902};
t4917 = ct{1903};
t4922 = ct{1904};
t4923 = ct{1905};
t4924 = ct{1906};
t4925 = ct{1907};
t4926 = ct{1908};
t4927 = ct{1909};
t4928 = ct{1910};
t4929 = ct{1911};
t4931 = ct{1912};
t4932 = ct{1913};
t4933 = ct{1914};
t4934 = ct{1915};
t4936 = ct{1916};
t4937 = ct{1917};
t4938 = ct{1918};
t4939 = ct{1919};
t4940 = ct{1920};
t4941 = ct{1921};
t4942 = ct{1922};
t4943 = ct{1923};
t4944 = ct{1924};
t4945 = ct{1925};
t4946 = ct{1926};
t4947 = ct{1927};
t4949 = ct{1928};
t4950 = ct{1929};
t4951 = ct{1930};
t4952 = ct{1931};
t4953 = ct{1932};
t4954 = ct{1933};
t4955 = ct{1934};
t496 = ct{1935};
t4960 = ct{1936};
t4961 = ct{1937};
t4963 = ct{1938};
t4964 = ct{1939};
t4966 = ct{1940};
t4967 = ct{1941};
t4968 = ct{1942};
t4969 = ct{1943};
t4972 = ct{1944};
t4973 = ct{1945};
t4975 = ct{1946};
t4976 = ct{1947};
t4977 = ct{1948};
t4978 = ct{1949};
t4979 = ct{1950};
t4980 = ct{1951};
t4981 = ct{1952};
t4982 = ct{1953};
t4983 = ct{1954};
t4984 = ct{1955};
t4985 = ct{1956};
t4986 = ct{1957};
t4987 = ct{1958};
t4988 = ct{1959};
t4989 = ct{1960};
t4990 = ct{1961};
t4993 = ct{1962};
t4995 = ct{1963};
t4997 = ct{1964};
t4998 = ct{1965};
t4999 = ct{1966};
t5 = ct{1967};
t50 = ct{1968};
t5000 = ct{1969};
t5001 = ct{1970};
t5002 = ct{1971};
t5004 = ct{1972};
t5005 = ct{1973};
t5006 = ct{1974};
t5007 = ct{1975};
t5008 = ct{1976};
t5009 = ct{1977};
t501 = ct{1978};
t5010 = ct{1979};
t5012 = ct{1980};
t5013 = ct{1981};
t5014 = ct{1982};
t5016 = ct{1983};
t5017 = ct{1984};
t5018 = ct{1985};
t502 = ct{1986};
t5021 = ct{1987};
t5022 = ct{1988};
t5023 = ct{1989};
t5024 = ct{1990};
t5025 = ct{1991};
t5027 = ct{1992};
t5028 = ct{1993};
t5030 = ct{1994};
t5031 = ct{1995};
t5032 = ct{1996};
t5033 = ct{1997};
t5034 = ct{1998};
t5035 = ct{1999};
t5036 = ct{2000};
t5038 = ct{2001};
t5039 = ct{2002};
t504 = ct{2003};
t5040 = ct{2004};
t5041 = ct{2005};
t5042 = ct{2006};
t5045 = ct{2007};
t5046 = ct{2008};
t5047 = ct{2009};
t5048 = ct{2010};
t5049 = ct{2011};
t5050 = ct{2012};
t5051 = ct{2013};
t5052 = ct{2014};
t5053 = ct{2015};
t5054 = ct{2016};
t5055 = ct{2017};
t5057 = ct{2018};
t5058 = ct{2019};
t5059 = ct{2020};
t5061 = ct{2021};
t5062 = ct{2022};
t5063 = ct{2023};
t5064 = ct{2024};
t5066 = ct{2025};
t5067 = ct{2026};
t5068 = ct{2027};
t5069 = ct{2028};
t5071 = ct{2029};
t5072 = ct{2030};
t5074 = ct{2031};
t5075 = ct{2032};
t5076 = ct{2033};
t5077 = ct{2034};
t5078 = ct{2035};
t5079 = ct{2036};
t5080 = ct{2037};
t5082 = ct{2038};
t5083 = ct{2039};
t5084 = ct{2040};
t5085 = ct{2041};
t5087 = ct{2042};
t5088 = ct{2043};
t5089 = ct{2044};
t5090 = ct{2045};
t5092 = ct{2046};
t5093 = ct{2047};
t5094 = ct{2048};
t5095 = ct{2049};
t5098 = ct{2050};
t5099 = ct{2051};
t51 = ct{2052};
t5100 = ct{2053};
t5101 = ct{2054};
t5102 = ct{2055};
t5103 = ct{2056};
t5104 = ct{2057};
t5106 = ct{2058};
t5107 = ct{2059};
t5109 = ct{2060};
t5110 = ct{2061};
t5111 = ct{2062};
t5112 = ct{2063};
t5114 = ct{2064};
t5115 = ct{2065};
t5117 = ct{2066};
t5118 = ct{2067};
t5120 = ct{2068};
t5121 = ct{2069};
t5123 = ct{2070};
t5124 = ct{2071};
t5126 = ct{2072};
t5128 = ct{2073};
t5131 = ct{2074};
t5132 = ct{2075};
t5134 = ct{2076};
t5135 = ct{2077};
t5136 = ct{2078};
t5137 = ct{2079};
t5138 = ct{2080};
t5139 = ct{2081};
t5140 = ct{2082};
t5142 = ct{2083};
t5143 = ct{2084};
t5144 = ct{2085};
t5145 = ct{2086};
t5146 = ct{2087};
t5148 = ct{2088};
t5149 = ct{2089};
t5150 = ct{2090};
t5152 = ct{2091};
t5153 = ct{2092};
t5154 = ct{2093};
t5155 = ct{2094};
t5156 = ct{2095};
t5157 = ct{2096};
t5158 = ct{2097};
t5161 = ct{2098};
t5162 = ct{2099};
t5163 = ct{2100};
t5165 = ct{2101};
t5166 = ct{2102};
t5167 = ct{2103};
t5168 = ct{2104};
t5169 = ct{2105};
t5171 = ct{2106};
t5172 = ct{2107};
t5173 = ct{2108};
t5174 = ct{2109};
t5175 = ct{2110};
t5177 = ct{2111};
t5178 = ct{2112};
t5179 = ct{2113};
t5180 = ct{2114};
t5182 = ct{2115};
t5183 = ct{2116};
t5184 = ct{2117};
t5185 = ct{2118};
t5186 = ct{2119};
t5187 = ct{2120};
t5188 = ct{2121};
t519 = ct{2122};
t5190 = ct{2123};
t5191 = ct{2124};
t5193 = ct{2125};
t5194 = ct{2126};
t5196 = ct{2127};
t5197 = ct{2128};
t5198 = ct{2129};
t5199 = ct{2130};
t5202 = ct{2131};
t5203 = ct{2132};
t5204 = ct{2133};
t5205 = ct{2134};
t5206 = ct{2135};
t5207 = ct{2136};
t5208 = ct{2137};
t5211 = ct{2138};
t5212 = ct{2139};
t5214 = ct{2140};
t5216 = ct{2141};
t5217 = ct{2142};
t5218 = ct{2143};
t5220 = ct{2144};
t5221 = ct{2145};
t5223 = ct{2146};
t5224 = ct{2147};
t5225 = ct{2148};
t5226 = ct{2149};
t5227 = ct{2150};
t5228 = ct{2151};
t5229 = ct{2152};
t523 = ct{2153};
t5231 = ct{2154};
t5232 = ct{2155};
t5233 = ct{2156};
t5234 = ct{2157};
t5235 = ct{2158};
t5238 = ct{2159};
t5239 = ct{2160};
t524 = ct{2161};
t5240 = ct{2162};
t5241 = ct{2163};
t5243 = ct{2164};
t5244 = ct{2165};
t5245 = ct{2166};
t5247 = ct{2167};
t5248 = ct{2168};
t5249 = ct{2169};
t5250 = ct{2170};
t5251 = ct{2171};
t5252 = ct{2172};
t5253 = ct{2173};
t5254 = ct{2174};
t5256 = ct{2175};
t5259 = ct{2176};
t5260 = ct{2177};
t5262 = ct{2178};
t5263 = ct{2179};
t5264 = ct{2180};
t5265 = ct{2181};
t5266 = ct{2182};
t5268 = ct{2183};
t5269 = ct{2184};
t527 = ct{2185};
t5270 = ct{2186};
t5272 = ct{2187};
t5274 = ct{2188};
t5275 = ct{2189};
t5276 = ct{2190};
t5277 = ct{2191};
t5279 = ct{2192};
t5280 = ct{2193};
t5281 = ct{2194};
t5284 = ct{2195};
t5285 = ct{2196};
t5286 = ct{2197};
t5287 = ct{2198};
t5288 = ct{2199};
t5289 = ct{2200};
t5290 = ct{2201};
t5291 = ct{2202};
t5292 = ct{2203};
t5293 = ct{2204};
t5294 = ct{2205};
t5295 = ct{2206};
t5296 = ct{2207};
t5297 = ct{2208};
t5298 = ct{2209};
t5299 = ct{2210};
t530 = ct{2211};
t5300 = ct{2212};
t5301 = ct{2213};
t5302 = ct{2214};
t5304 = ct{2215};
t5305 = ct{2216};
t5306 = ct{2217};
t5307 = ct{2218};
t5308 = ct{2219};
t5309 = ct{2220};
t5310 = ct{2221};
t5311 = ct{2222};
t5312 = ct{2223};
t5313 = ct{2224};
t5314 = ct{2225};
t5316 = ct{2226};
t5317 = ct{2227};
t5318 = ct{2228};
t5319 = ct{2229};
t5321 = ct{2230};
t5322 = ct{2231};
t5324 = ct{2232};
t5325 = ct{2233};
t5326 = ct{2234};
t5327 = ct{2235};
t5328 = ct{2236};
t5329 = ct{2237};
t5330 = ct{2238};
t5332 = ct{2239};
t5333 = ct{2240};
t5335 = ct{2241};
t5336 = ct{2242};
t5337 = ct{2243};
t5338 = ct{2244};
t5339 = ct{2245};
t534 = ct{2246};
t5340 = ct{2247};
t5341 = ct{2248};
t5343 = ct{2249};
t5344 = ct{2250};
t5345 = ct{2251};
t5346 = ct{2252};
t5347 = ct{2253};
t5349 = ct{2254};
t5350 = ct{2255};
t5351 = ct{2256};
t5352 = ct{2257};
t5353 = ct{2258};
t5354 = ct{2259};
t5356 = ct{2260};
t5357 = ct{2261};
t5358 = ct{2262};
t5359 = ct{2263};
t5360 = ct{2264};
t5361 = ct{2265};
t5363 = ct{2266};
t5364 = ct{2267};
t5366 = ct{2268};
t5368 = ct{2269};
t5369 = ct{2270};
t537 = ct{2271};
t5370 = ct{2272};
t5371 = ct{2273};
t5372 = ct{2274};
t5374 = ct{2275};
t5376 = ct{2276};
t5377 = ct{2277};
t5378 = ct{2278};
t5379 = ct{2279};
t5380 = ct{2280};
t5381 = ct{2281};
t5382 = ct{2282};
t5383 = ct{2283};
t5384 = ct{2284};
t5385 = ct{2285};
t5386 = ct{2286};
t5388 = ct{2287};
t5389 = ct{2288};
t539 = ct{2289};
t5391 = ct{2290};
t5392 = ct{2291};
t5393 = ct{2292};
t5394 = ct{2293};
t5395 = ct{2294};
t5396 = ct{2295};
t5398 = ct{2296};
t5399 = ct{2297};
t54 = ct{2298};
t5400 = ct{2299};
t5402 = ct{2300};
t5403 = ct{2301};
t5404 = ct{2302};
t5405 = ct{2303};
t5406 = ct{2304};
t5407 = ct{2305};
t5408 = ct{2306};
t5409 = ct{2307};
t541 = ct{2308};
t5411 = ct{2309};
t5412 = ct{2310};
t5413 = ct{2311};
t5414 = ct{2312};
t5415 = ct{2313};
t5416 = ct{2314};
t5417 = ct{2315};
t5418 = ct{2316};
t5419 = ct{2317};
t542 = ct{2318};
t5420 = ct{2319};
t5421 = ct{2320};
t5422 = ct{2321};
t5423 = ct{2322};
t5425 = ct{2323};
t5426 = ct{2324};
t5427 = ct{2325};
t5428 = ct{2326};
t5430 = ct{2327};
t5431 = ct{2328};
t5434 = ct{2329};
t5435 = ct{2330};
t5436 = ct{2331};
t5438 = ct{2332};
t5439 = ct{2333};
t544 = ct{2334};
t5441 = ct{2335};
t5442 = ct{2336};
t5443 = ct{2337};
t5444 = ct{2338};
t5447 = ct{2339};
t5448 = ct{2340};
t5449 = ct{2341};
t5450 = ct{2342};
t5452 = ct{2343};
t5453 = ct{2344};
t5455 = ct{2345};
t5456 = ct{2346};
t5458 = ct{2347};
t5459 = ct{2348};
t546 = ct{2349};
t5460 = ct{2350};
t5461 = ct{2351};
t5462 = ct{2352};
t5463 = ct{2353};
t5464 = ct{2354};
t5465 = ct{2355};
t5467 = ct{2356};
t5468 = ct{2357};
t5470 = ct{2358};
t5471 = ct{2359};
t5474 = ct{2360};
t5475 = ct{2361};
t5476 = ct{2362};
t5478 = ct{2363};
t5480 = ct{2364};
t5481 = ct{2365};
t5483 = ct{2366};
t5484 = ct{2367};
t5486 = ct{2368};
t5487 = ct{2369};
t5488 = ct{2370};
t5489 = ct{2371};
t5490 = ct{2372};
t5492 = ct{2373};
t5493 = ct{2374};
t5494 = ct{2375};
t5495 = ct{2376};
t5496 = ct{2377};
t5497 = ct{2378};
t5498 = ct{2379};
t5499 = ct{2380};
t55 = ct{2381};
t550 = ct{2382};
t5500 = ct{2383};
t5502 = ct{2384};
t5508 = ct{2385};
t5509 = ct{2386};
t5510 = ct{2387};
t5511 = ct{2388};
t5513 = ct{2389};
t5514 = ct{2390};
t5515 = ct{2391};
t5516 = ct{2392};
t5519 = ct{2393};
t5520 = ct{2394};
t5521 = ct{2395};
t5523 = ct{2396};
t5524 = ct{2397};
t5527 = ct{2398};
t5528 = ct{2399};
t553 = ct{2400};
t5530 = ct{2401};
t5531 = ct{2402};
t5532 = ct{2403};
t5533 = ct{2404};
t5534 = ct{2405};
t5535 = ct{2406};
t5536 = ct{2407};
t5538 = ct{2408};
t5539 = ct{2409};
t5540 = ct{2410};
t5542 = ct{2411};
t5543 = ct{2412};
t5546 = ct{2413};
t5547 = ct{2414};
t5548 = ct{2415};
t5550 = ct{2416};
t5551 = ct{2417};
t5552 = ct{2418};
t5553 = ct{2419};
t5556 = ct{2420};
t5557 = ct{2421};
t5563 = ct{2422};
t5565 = ct{2423};
t5566 = ct{2424};
t5569 = ct{2425};
t557 = ct{2426};
t5571 = ct{2427};
t5573 = ct{2428};
t5575 = ct{2429};
t5576 = ct{2430};
t5578 = ct{2431};
t558 = ct{2432};
t5580 = ct{2433};
t5582 = ct{2434};
t5585 = ct{2435};
t5588 = ct{2436};
t5592 = ct{2437};
t5597 = ct{2438};
t5598 = ct{2439};
t5599 = ct{2440};
t56 = ct{2441};
t5601 = ct{2442};
t5602 = ct{2443};
t5603 = ct{2444};
t5606 = ct{2445};
t5607 = ct{2446};
t5616 = ct{2447};
t5618 = ct{2448};
t5619 = ct{2449};
t5620 = ct{2450};
t5622 = ct{2451};
t5623 = ct{2452};
t5627 = ct{2453};
t5629 = ct{2454};
t5631 = ct{2455};
t5632 = ct{2456};
t5633 = ct{2457};
t5638 = ct{2458};
t5642 = ct{2459};
t5644 = ct{2460};
t5648 = ct{2461};
t5657 = ct{2462};
t5658 = ct{2463};
t5659 = ct{2464};
t5660 = ct{2465};
t5661 = ct{2466};
t5662 = ct{2467};
t5663 = ct{2468};
t5664 = ct{2469};
t5667 = ct{2470};
t5668 = ct{2471};
t5670 = ct{2472};
t5672 = ct{2473};
t5674 = ct{2474};
t5677 = ct{2475};
t5678 = ct{2476};
t5682 = ct{2477};
t5684 = ct{2478};
t5685 = ct{2479};
t5686 = ct{2480};
t5687 = ct{2481};
t5688 = ct{2482};
t5689 = ct{2483};
t5690 = ct{2484};
t5691 = ct{2485};
t5692 = ct{2486};
t5693 = ct{2487};
t5694 = ct{2488};
t5696 = ct{2489};
t5697 = ct{2490};
t5699 = ct{2491};
t5704 = ct{2492};
t5705 = ct{2493};
t5706 = ct{2494};
t5707 = ct{2495};
t5709 = ct{2496};
t5710 = ct{2497};
t5712 = ct{2498};
t5713 = ct{2499};
t5715 = ct{2500};
t5717 = ct{2501};
t5721 = ct{2502};
t5722 = ct{2503};
t5724 = ct{2504};
t5726 = ct{2505};
t573 = ct{2506};
t5730 = ct{2507};
t5731 = ct{2508};
t5733 = ct{2509};
t5734 = ct{2510};
t5738 = ct{2511};
t574 = ct{2512};
t5741 = ct{2513};
t5745 = ct{2514};
t5749 = ct{2515};
t575 = ct{2516};
t5754 = ct{2517};
t5756 = ct{2518};
t5761 = ct{2519};
t5763 = ct{2520};
t5771 = ct{2521};
t5772 = ct{2522};
t5776 = ct{2523};
t5778 = ct{2524};
t5779 = ct{2525};
t5780 = ct{2526};
t5781 = ct{2527};
t5785 = ct{2528};
t5786 = ct{2529};
t5788 = ct{2530};
t5789 = ct{2531};
t5791 = ct{2532};
t5792 = ct{2533};
t5793 = ct{2534};
t5795 = ct{2535};
t5798 = ct{2536};
t5800 = ct{2537};
t5805 = ct{2538};
t5808 = ct{2539};
t5809 = ct{2540};
t5814 = ct{2541};
t5815 = ct{2542};
t5818 = ct{2543};
t5820 = ct{2544};
t5823 = ct{2545};
t5824 = ct{2546};
t5826 = ct{2547};
t5829 = ct{2548};
t5832 = ct{2549};
t5835 = ct{2550};
t5837 = ct{2551};
t5840 = ct{2552};
t5841 = ct{2553};
t5843 = ct{2554};
t5845 = ct{2555};
t5846 = ct{2556};
t5847 = ct{2557};
t5848 = ct{2558};
t5855 = ct{2559};
t5857 = ct{2560};
t5859 = ct{2561};
t5862 = ct{2562};
t5867 = ct{2563};
t5868 = ct{2564};
t5869 = ct{2565};
t587 = ct{2566};
t5870 = ct{2567};
t5874 = ct{2568};
t5880 = ct{2569};
t5881 = ct{2570};
t5887 = ct{2571};
t5889 = ct{2572};
t5891 = ct{2573};
t5894 = ct{2574};
t5895 = ct{2575};
t5897 = ct{2576};
t59 = ct{2577};
t5901 = ct{2578};
t5905 = ct{2579};
t5908 = ct{2580};
t5909 = ct{2581};
t5910 = ct{2582};
t5915 = ct{2583};
t5916 = ct{2584};
t5917 = ct{2585};
t5919 = ct{2586};
t5923 = ct{2587};
t5925 = ct{2588};
t5926 = ct{2589};
t5932 = ct{2590};
t5933 = ct{2591};
t5935 = ct{2592};
t5936 = ct{2593};
t5939 = ct{2594};
t5941 = ct{2595};
t5947 = ct{2596};
t5949 = ct{2597};
t595 = ct{2598};
t5959 = ct{2599};
t5960 = ct{2600};
t5963 = ct{2601};
t5964 = ct{2602};
t5967 = ct{2603};
t5970 = ct{2604};
t5971 = ct{2605};
t5973 = ct{2606};
t5980 = ct{2607};
t5981 = ct{2608};
t5982 = ct{2609};
t5983 = ct{2610};
t5984 = ct{2611};
t5985 = ct{2612};
t5986 = ct{2613};
t5988 = ct{2614};
t5989 = ct{2615};
t5990 = ct{2616};
t5991 = ct{2617};
t5992 = ct{2618};
t5996 = ct{2619};
t5998 = ct{2620};
t6000 = ct{2621};
t6001 = ct{2622};
t6009 = ct{2623};
t6010 = ct{2624};
t6013 = ct{2625};
t6014 = ct{2626};
t6015 = ct{2627};
t6021 = ct{2628};
t6024 = ct{2629};
t6026 = ct{2630};
t6029 = ct{2631};
t603 = ct{2632};
t6030 = ct{2633};
t6036 = ct{2634};
t6039 = ct{2635};
t6042 = ct{2636};
t6045 = ct{2637};
t6049 = ct{2638};
t6051 = ct{2639};
t6052 = ct{2640};
t6056 = ct{2641};
t6057 = ct{2642};
t6058 = ct{2643};
t6066 = ct{2644};
t6069 = ct{2645};
t6074 = ct{2646};
t6075 = ct{2647};
t6086 = ct{2648};
t6089 = ct{2649};
t6090 = ct{2650};
t6091 = ct{2651};
t6099 = ct{2652};
t61 = ct{2653};
t6101 = ct{2654};
t6104 = ct{2655};
t6105 = ct{2656};
t6106 = ct{2657};
t6111 = ct{2658};
t6117 = ct{2659};
t6125 = ct{2660};
t6128 = ct{2661};
t6129 = ct{2662};
t6138 = ct{2663};
t614 = ct{2664};
t6140 = ct{2665};
t6143 = ct{2666};
t6150 = ct{2667};
t6158 = ct{2668};
t6161 = ct{2669};
t6164 = ct{2670};
t6166 = ct{2671};
t6171 = ct{2672};
t6174 = ct{2673};
t6176 = ct{2674};
t6182 = ct{2675};
t6183 = ct{2676};
t6191 = ct{2677};
t6195 = ct{2678};
t6196 = ct{2679};
t6197 = ct{2680};
t6198 = ct{2681};
t6199 = ct{2682};
t6204 = ct{2683};
t6205 = ct{2684};
t6211 = ct{2685};
t6219 = ct{2686};
t6221 = ct{2687};
t6222 = ct{2688};
t6225 = ct{2689};
t6229 = ct{2690};
t6230 = ct{2691};
t6231 = ct{2692};
t6234 = ct{2693};
t6236 = ct{2694};
t6240 = ct{2695};
t6241 = ct{2696};
t6249 = ct{2697};
t6253 = ct{2698};
t6258 = ct{2699};
t6261 = ct{2700};
t6264 = ct{2701};
t6268 = ct{2702};
t6273 = ct{2703};
t6274 = ct{2704};
t6275 = ct{2705};
t6277 = ct{2706};
t6278 = ct{2707};
t628 = ct{2708};
t6281 = ct{2709};
t6282 = ct{2710};
t6284 = ct{2711};
t629 = ct{2712};
t6290 = ct{2713};
t6292 = ct{2714};
t6295 = ct{2715};
t6296 = ct{2716};
t6303 = ct{2717};
t6304 = ct{2718};
t6309 = ct{2719};
t6311 = ct{2720};
t6314 = ct{2721};
t6315 = ct{2722};
t6316 = ct{2723};
t6317 = ct{2724};
t6320 = ct{2725};
t6330 = ct{2726};
t6332 = ct{2727};
t634 = ct{2728};
t6345 = ct{2729};
t6347 = ct{2730};
t6351 = ct{2731};
t6354 = ct{2732};
t6356 = ct{2733};
t6361 = ct{2734};
t6365 = ct{2735};
t6369 = ct{2736};
t6370 = ct{2737};
t6372 = ct{2738};
t6385 = ct{2739};
t6388 = ct{2740};
t6389 = ct{2741};
t6391 = ct{2742};
t6393 = ct{2743};
t6399 = ct{2744};
t6400 = ct{2745};
t6405 = ct{2746};
t6406 = ct{2747};
t6409 = ct{2748};
t641 = ct{2749};
t6410 = ct{2750};
t6413 = ct{2751};
t6421 = ct{2752};
t6422 = ct{2753};
t6430 = ct{2754};
t6433 = ct{2755};
t6434 = ct{2756};
t6439 = ct{2757};
t6443 = ct{2758};
t6446 = ct{2759};
t6447 = ct{2760};
t6448 = ct{2761};
t6449 = ct{2762};
t6450 = ct{2763};
t6455 = ct{2764};
t6460 = ct{2765};
t6471 = ct{2766};
t6482 = ct{2767};
t6483 = ct{2768};
t6484 = ct{2769};
t6485 = ct{2770};
t6486 = ct{2771};
t6487 = ct{2772};
t6495 = ct{2773};
t6497 = ct{2774};
t65 = ct{2775};
t650 = ct{2776};
t6501 = ct{2777};
t6506 = ct{2778};
t651 = ct{2779};
t6510 = ct{2780};
t6526 = ct{2781};
t6531 = ct{2782};
t6538 = ct{2783};
t6539 = ct{2784};
t6549 = ct{2785};
t655 = ct{2786};
t6550 = ct{2787};
t6552 = ct{2788};
t6555 = ct{2789};
t6562 = ct{2790};
t6565 = ct{2791};
t6567 = ct{2792};
t657 = ct{2793};
t6571 = ct{2794};
t6580 = ct{2795};
t6581 = ct{2796};
t6584 = ct{2797};
t6588 = ct{2798};
t6602 = ct{2799};
t6611 = ct{2800};
t6612 = ct{2801};
t6613 = ct{2802};
t6614 = ct{2803};
t6615 = ct{2804};
t6616 = ct{2805};
t6617 = ct{2806};
t6618 = ct{2807};
t6619 = ct{2808};
t6620 = ct{2809};
t6629 = ct{2810};
t6630 = ct{2811};
t6634 = ct{2812};
t6635 = ct{2813};
t6636 = ct{2814};
t6637 = ct{2815};
t6638 = ct{2816};
t664 = ct{2817};
t6640 = ct{2818};
t6641 = ct{2819};
t6645 = ct{2820};
t6646 = ct{2821};
t6647 = ct{2822};
t665 = ct{2823};
t6653 = ct{2824};
t6656 = ct{2825};
t666 = ct{2826};
t6669 = ct{2827};
t667 = ct{2828};
t6673 = ct{2829};
t6677 = ct{2830};
t668 = ct{2831};
t6681 = ct{2832};
t669 = ct{2833};
t6699 = ct{2834};
t6709 = ct{2835};
t6729 = ct{2836};
t6739 = ct{2837};
t6743 = ct{2838};
t6745 = ct{2839};
t675 = ct{2840};
t6754 = ct{2841};
t6755 = ct{2842};
t6756 = ct{2843};
t6762 = ct{2844};
t6763 = ct{2845};
t6764 = ct{2846};
t6770 = ct{2847};
t6772 = ct{2848};
t6773 = ct{2849};
t6775 = ct{2850};
t6776 = ct{2851};
t6779 = ct{2852};
t6780 = ct{2853};
t6781 = ct{2854};
t6792 = ct{2855};
t6798 = ct{2856};
t68 = ct{2857};
t693 = ct{2858};
t7 = ct{2859};
t71 = ct{2860};
t721 = ct{2861};
t724 = ct{2862};
t73 = ct{2863};
t731 = ct{2864};
t732 = ct{2865};
t736 = ct{2866};
t741 = ct{2867};
t753 = ct{2868};
t754 = ct{2869};
t755 = ct{2870};
t757 = ct{2871};
t765 = ct{2872};
t769 = ct{2873};
t772 = ct{2874};
t774 = ct{2875};
t776 = ct{2876};
t778 = ct{2877};
t795 = ct{2878};
t797 = ct{2879};
t799 = ct{2880};
t8 = ct{2881};
t802 = ct{2882};
t803 = ct{2883};
t806 = ct{2884};
t817 = ct{2885};
t818 = ct{2886};
t820 = ct{2887};
t828 = ct{2888};
t831 = ct{2889};
t838 = ct{2890};
t843 = ct{2891};
t846 = ct{2892};
t847 = ct{2893};
t850 = ct{2894};
t851 = ct{2895};
t852 = ct{2896};
t853 = ct{2897};
t855 = ct{2898};
t865 = ct{2899};
t867 = ct{2900};
t868 = ct{2901};
t870 = ct{2902};
t871 = ct{2903};
t872 = ct{2904};
t876 = ct{2905};
t886 = ct{2906};
t888 = ct{2907};
t9 = ct{2908};
t901 = ct{2909};
t902 = ct{2910};
t903 = ct{2911};
t904 = ct{2912};
t907 = ct{2913};
t909 = ct{2914};
t914 = ct{2915};
t925 = ct{2916};
t926 = ct{2917};
t947 = ct{2918};
t949 = ct{2919};
t952 = ct{2920};
t955 = ct{2921};
t957 = ct{2922};
t964 = ct{2923};
t972 = ct{2924};
t977 = ct{2925};
t983 = ct{2926};
t991 = ct{2927};
t992 = ct{2928};
t993 = ct{2929};
t994 = ct{2930};
t995 = ct{2931};
t5541 = ITail.*t4522.*t4785;
t5544 = t4408.*t4858;
t5545 = ITail.*t4409.*t4849;
t5549 = -t5540;
t5554 = t4578.*t4737;
t5555 = t4645.*t4704;
t5558 = ITail.*t4459.*t4821;
t5560 = ITail.*t4077.*t5022;
t5561 = -t5550;
t5562 = t2255+t2343+t3315+t3402+t3429+t3459;
t5570 = -t5563;
t5574 = -t4989.*(-t1262+t1701+t9.*t868.*(t105-t465));
t5577 = ITail.*t4408.*t4881;
t5581 = ITail.*t4392.*t4900;
t5584 = t4447.*t4858;
t5586 = t4500.*t4820;
t5589 = -t5580;
t5590 = t4555.*t4785;
t5591 = t4578.*t4753;
t5593 = ITail.*t4459.*t4830;
t5594 = -ITail.*t4459.*(-t1129+t1139-t2082+t2110+t2123+t8.*t872.*(t534-t546));
t5600 = ITail.*t4459.*t4834;
t5604 = ITail.*t4447.*t4881;
t5605 = t2249+t2515+t3059+t3187+t3730+t3755;
t5609 = ITail.*t4409.*t4897;
t5610 = t3570+t4520+t4528;
t5611 = -t5603;
t5613 = -t4989.*(-t947+t1240.*(t105-t465)+t903.*(t534-t546));
t5615 = ITail.*t4459.*t4849;
t5617 = t4277.*t4980;
t5621 = -t4704.*(t995+t1064-t1506+t1598-t1763-t1774);
t5624 = ITail.*t4447.*t4900;
t5625 = t4476.*t4858;
t5628 = -t4704.*(t820+t1121-t1435+t1997+t2000+t11.*t420.*(t214-t541));
t5630 = t4578.*t4787;
t5634 = -t5627;
t5635 = ITail.*t4392.*t4928;
t5636 = t4704.*(t820+t1121-t1435+t1997+t2000+t11.*t420.*(t214-t541));
t5637 = t4551.*t4820;
t5639 = t846+t955+t957+t1716+t1943+t1950+t4749;
t5640 = -t4681.*(t1064+t1137-t1694+t1698-t1763-t1774);
t5641 = t4277.*t5006;
t5643 = t4313.*t4980;
t5649 = ITail.*t4476.*t4881;
t5653 = ITail.*t4409.*t4923;
t5656 = ITail.*t4409.*t4922;
t5665 = ITail.*t4408.*t4928;
t5669 = t4277.*t5023;
t5675 = -t5667;
t5679 = ITail.*t4476.*t4900;
t5681 = t4681.*t4738;
t5683 = t4313.*t5006;
t5695 = -t5686;
t5698 = -t5693;
t5700 = t4313.*t5023;
t5701 = -t4704.*(t867+t1059-t1646-t1705+t1938-t2002);
t5711 = ITail.*t4459.*t4922;
t5714 = -t5710;
t5718 = -t4980.*(-t1331+t2317+t1510.*(t103-t544));
t5719 = -t4989.*(t1332+t2368+t1512.*(t105-t465));
t5720 = t4681.*t4770;
t5723 = -t4820.*(-t2388+t3008+t9.*t868.*(t105-t465).*9.53094055e-4);
t5725 = ITail.*t4409.*t4972;
t5727 = dphi1.*t5721;
t5728 = dphi1.*t5722;
t5729 = dx.*t5722;
t5732 = ITail.*t4476.*t4928;
t5735 = t4634.*t4821;
t5736 = -t5006.*(-t1331+t2317+t1510.*(t103-t544));
t5737 = -t5733;
t5739 = t5006.*(-t1331+t2317+t1510.*(t103-t544));
t5742 = -t4820.*(-t1974+t1240.*(t105-t465).*9.53094055e-4+t903.*(t534-t546).*9.53094055e-4);
t5743 = t4634.*t4823;
t5746 = -t5741;
t5748 = -t4681.*(t1060+t1138-t1883+t1932+t2088+t1179.*(t103-t544));
t5750 = -t5023.*(-t1331+t2317+t1510.*(t103-t544));
t5751 = t2590+t2616+t3668+t3698+t3738+t3764;
t5752 = -t4634.*(-t1129+t1139-t2082+t2110+t2123+t8.*t872.*(t534-t546));
t5753 = t4681.*(t1060+t1138-t1883+t1932+t2088+t1179.*(t103-t544));
t5755 = t4634.*t4834;
t5758 = ITail.*t4459.*t4972;
t5759 = t4634.*(-t1129+t1139-t2082+t2110+t2123+t8.*t872.*(t534-t546));
t5760 = -ITail.*t4409.*(t1176-t1366+t2434+t2435-t2899+t1430.*(t539+t641));
t5762 = ITail.*t4409.*t5022;
t5765 = -t4681.*(t1250-t1261+t1761-t2083-t2111+t1037.*(t103-t544));
t5766 = ITail.*t4409.*(t1176-t1366+t2434+t2435-t2899+t1430.*(t539+t641));
t5767 = -t5761;
t5768 = t4634.*t4849;
t5769 = t3961.*t5304;
t5770 = t3938.*t5313;
t5774 = -t4681.*(t1053+t1332+t2368+t817.*(t214-t541)+t977.*(t103-t544)+t1512.*(t105-t465));
t5775 = -t4704.*(t1060+t1138-t1883+t1932+t2088+t1179.*(t103-t544));
t5782 = t3900+t4572+t4589;
t5783 = ITail.*t4452.*t5022;
t5794 = -t4704.*(t1250-t1261+t1761-t2083-t2111+t1037.*(t103-t544));
t5797 = ITail.*t4522.*t4972;
t5799 = t2884+t2954+t3689+t3723+t3742+t3766;
t5801 = -t4753.*(t2436-t2536+t1510.*(t197-t537)+t1505.*(t214-t541));
t5802 = t4704.*(t1250-t1261+t1761-t2083-t2111+t1037.*(t103-t544));
t5803 = t4737.*t4785;
t5804 = -t4704.*(t1053+t1332+t2368+t817.*(t214-t541)+t977.*(t103-t544)+t1512.*(t105-t465));
t5807 = -ITail.*t4459.*(t1176-t1366+t2434+t2435-t2899+t1430.*(t539+t641));
t5811 = t4634.*t4897;
t5813 = t4704.*(t1053+t1332+t2368+t817.*(t214-t541)+t977.*(t103-t544)+t1512.*(t105-t465));
t5821 = dth1.*t5818;
t5827 = t4753.*t4785;
t5828 = t4555.*t4972;
t5831 = -ITail.*t4409.*(t1365-t1443+t2829-t2831-t2833+t1505.*(t534-t546));
t5833 = t4173.*t5304;
t5834 = -t5304.*(-t1262+t1701+t9.*t868.*(t105-t465));
t5836 = ITail.*t4522.*t5022;
t5838 = t4634.*t4923;
t5839 = t4634.*t4922;
t5850 = t4785.*t4787;
t5852 = -t5848;
t5853 = t2648+t2707+t3867+t3871+t3885+t3898;
t5856 = t4753.*t4821;
t5858 = t4555.*t5022;
t5860 = -ITail.*t4459.*(t1365-t1443+t2829-t2831-t2833+t1505.*(t534-t546));
t5863 = -t5859;
t5865 = ITail.*t4459.*(t1365-t1443+t2829-t2831-t2833+t1505.*(t534-t546));
t5871 = t4753.*t4830;
t5872 = -t4753.*(-t1129+t1139-t2082+t2110+t2123+t8.*t872.*(t534-t546));
t5873 = t4162.*t5392;
t5875 = t4753.*t4834;
t5883 = t4634.*t4972;
t5885 = t4753.*t4849;
t5890 = t3961.*(t2134-t2147+t3286+t3329+t3378-t1178.*(t105-t465).*9.53094055e-4);
t5898 = -t5891;
t5902 = -t5897;
t5904 = t3961.*t5519;
t5911 = -t4634.*(t1176-t1366+t2434+t2435-t2899+t1430.*(t539+t641));
t5912 = t4634.*t5022;
t5913 = -t5304.*(t1332+t2368+t1512.*(t105-t465));
t5914 = t4634.*(t1176-t1366+t2434+t2435-t2899+t1430.*(t539+t641));
t5920 = t4162.*t5474;
t5921 = -t5916;
t5924 = t4313.*t5392;
t5928 = -t5919;
t5930 = -t5923;
t5937 = t4408.*t5313;
t5938 = t3938.*t5597;
t5945 = t4753.*t4922;
t5946 = t4173.*(t2134-t2147+t3286+t3329+t3378-t1178.*(t105-t465).*9.53094055e-4);
t5948 = -(-t1262+t1701+t9.*t868.*(t105-t465)).*(t2134-t2147+t3286+t3329+t3378-t1178.*(t105-t465).*9.53094055e-4);
t5951 = t4162.*t5514;
t5953 = t4447.*t5313;
t5955 = t4173.*t5519;
t5956 = t4277.*t5474;
t5958 = -t5519.*(-t1262+t1701+t9.*t868.*(t105-t465));
t5962 = -(-t947+t1240.*(t105-t465)+t903.*(t534-t546)).*(t2134-t2147+t3286+t3329+t3378-t1178.*(t105-t465).*9.53094055e-4);
t5965 = -t4634.*(t1365-t1443+t2829-t2831-t2833+t1505.*(t534-t546));
t5968 = -t5392.*(-t1331+t2317+t1510.*(t103-t544));
t5969 = -t5964;
t5972 = -t5967;
t5974 = t4476.*t5313;
t5975 = -t5519.*(-t947+t1240.*(t105-t465)+t903.*(t534-t546));
t5976 = t4277.*t5514;
t5977 = t5519.*(-t947+t1240.*(t105-t465)+t903.*(t534-t546));
t5978 = t4753.*t4972;
t5987 = t4737.*t5022;
t5993 = t4787.*t4972;
t5994 = -t4753.*(t1176-t1366+t2434+t2435-t2899+t1430.*(t539+t641));
t5995 = -t5474.*(-t1331+t2317+t1510.*(t103-t544));
t6002 = t3938.*(t2590+t2616-t3627+t3698+t3738+t3764);
t6003 = -t5514.*(-t1331+t2317+t1510.*(t103-t544));
t6004 = -t6001;
t6006 = t4787.*t5022;
t6008 = t5514.*(-t1331+t2317+t1510.*(t103-t544));
t6011 = dphi1.*t6009;
t6016 = t650+t1406+t1476+t1508+t2673+t3322+t3473+t4157+t4195;
t6017 = -t4753.*(t1365-t1443+t2829-t2831-t2833+t1505.*(t534-t546));
t6018 = -t6015;
t6022 = t4753.*(t1365-t1443+t2829-t2831-t2833+t1505.*(t534-t546));
t6023 = t3938.*t5793;
t6027 = t4392.*t5597;
t6028 = -t6026;
t6031 = -t6030;
t6032 = t3961.*t5823;
t6037 = t4447.*t5597;
t6043 = t4162.*t5780;
t6054 = t4476.*t5597;
t6059 = t4173.*t5823;
t6060 = -t6056;
t6062 = -t5823.*(-t1262+t1701+t9.*t868.*(t105-t465));
t6064 = t4277.*t5780;
t6071 = -t5823.*(-t947+t1240.*(t105-t465)+t903.*(t534-t546));
t6073 = t4313.*t5780;
t6079 = t4392.*(t2590+t2616-t3627+t3698+t3738+t3764);
t6088 = t4447.*(t2590+t2616-t3627+t3698+t3738+t3764);
t6092 = -t5780.*(-t1331+t2317+t1510.*(t103-t544));
t6095 = t4392.*t5793;
t6103 = t4408.*t5793;
t6110 = t1982+t2004+t2358+t3146+t3151+t3193+t3236+t3820+t3838;
t6113 = t4476.*(t2590+t2616-t3627+t3698+t3738+t3764);
t6114 = t4392.*t5829;
t6116 = t4447.*t5793;
t6118 = t4408.*t5829;
t6120 = t1971+t2004+t2543+t3193+t3236+t3351+t3359+t3794+t3817;
t6121 = t1865+t2186+t2543+t3212+t3217+t3336+t3390+t3794+t3817;
t6122 = t1865+t2004+t2750+t3193+t3212+t3217+t3236+t3845+t3870;
t6124 = t1982+t2004+t2599+t3146+t3151+t3193+t3236+t3887+t3918;
t6127 = t4447.*t5829;
t6137 = t2130+t2178+t2358+t3277+t3284+t3328+t3376+t3820+t3838;
t6144 = t4476.*t5829;
t6160 = dth1.*(-t1077+t1748+t1781-t2429+t3893+t3896-t4987);
t6173 = t1133+t2012+t2018+t2523+t4017+t4022+t4979;
t6181 = -t4578.*(t2449.*3.36554e-3+t3490+t3544+t3545-t4001-t4034);
t6184 = t3967.*t6104;
t6188 = t4173.*t6090;
t6189 = t4162.*t6089;
t6190 = t4164.*t6089;
t6201 = -t6197;
t6202 = -t6198;
t6203 = -t6199;
t6206 = t4173.*t6105;
t6207 = t4162.*t6104;
t6208 = t4237.*t6089;
t6210 = t4162.*t6111;
t6212 = t4255.*t6090;
t6216 = t3961.*t6138;
t6217 = t2824+t3522+t4272+t4281+t4524+t4534;
t6218 = t4237.*t6104;
t6220 = t4255.*t6105;
t6223 = -t6219;
t6224 = -t6221;
t6228 = t4311.*t6090;
t6233 = t4277.*t6111;
t6235 = -t6231;
t6238 = -t6236;
t6239 = t3521+t3571+t4290+t4308+t4483+t4498;
t6243 = t4313.*t6111;
t6245 = t4173.*t6138;
t6248 = -t6138.*(-t1262+t1701+t9.*t868.*(t105-t465));
t6250 = -t6089.*(t1260-t2364+t1430.*(t105-t465));
t6251 = t6089.*(t1260-t2364+t1430.*(t105-t465));
t6252 = t2823+t3235+t4387+t4399+t4484+t4499;
t6255 = -t6138.*(-t947+t1240.*(t105-t465)+t903.*(t534-t546));
t6257 = t6138.*(-t947+t1240.*(t105-t465)+t903.*(t534-t546));
t6259 = -t6104.*(t1260-t2364+t1430.*(t105-t465));
t6260 = t4382.*t6105;
t6265 = -t6091.*(t1396-t2573+t1430.*(t197-t537).*2.0);
t6267 = -t6111.*(-t1331+t2317+t1510.*(t103-t544));
t6269 = t6091.*(t1396-t2573+t1430.*(t197-t537).*2.0);
t6271 = t6111.*(-t1331+t2317+t1510.*(t103-t544));
t6272 = -t6268;
t6276 = -t4820.*(t2449.*3.372786875e-3+t3544+t3545+t3598-t3934-t3966);
t6279 = -t6275;
t6280 = -t6106.*(t1396-t2573+t1430.*(t197-t537).*2.0);
t6283 = -t6282;
t6285 = t4471.*t6091;
t6286 = t4454.*t6104;
t6289 = t4392.*t6125;
t6293 = -t6091.*(t1395-t2868+t1505.*(t534-t546).*2.0);
t6294 = -t6292;
t6298 = t4408.*t6125;
t6299 = t6091.*(t1395-t2868+t1505.*(t534-t546).*2.0);
t6302 = t4471.*t6106;
t6305 = -t6104.*(-t1018+t1426+t1431-t1446+t3.*t496.*(t105-t465));
t6307 = t4447.*t6125;
t6308 = -t6106.*(t1395-t2868+t1505.*(t534-t546).*2.0);
t6310 = t6106.*(t1395-t2868+t1505.*(t534-t546).*2.0);
t6312 = t3499+t3805+t4352+t4364+t4530+t4542;
t6319 = t4476.*t6125;
t6322 = -t6320;
t6323 = t4575.*t6089;
t6324 = t4578.*t6091;
t6325 = t4581.*t6089;
t6328 = t4592.*t6090;
t6333 = t4575.*t6104;
t6334 = t4578.*t6106;
t6335 = t4618.*t6090;
t6336 = t4592.*t6105;
t6337 = -t6104.*(t1019-t1651+t1702+t3.*t818.*(t105-t465)+t3.*t872.*(t103-t544));
t6339 = t4638.*t6089;
t6340 = t4645.*t6090;
t6341 = -t6089.*(t1751+t2308+t964.*(t105-t465)+t1430.*(t103-t544));
t6343 = t6089.*(t1751+t2308+t964.*(t105-t465)+t1430.*(t103-t544));
t6344 = t4618.*t6105;
t6346 = -t4578.*(-t1865+t1970+t2708+t3161-t3236-t3845-t3870+t1240.*(t105-t465).*3.36554e-3+t903.*(t534-t546).*3.36554e-3);
t6348 = t4638.*t6104;
t6349 = -t4972.*(t2449.*3.36554e-3+t3490+t3544+t3545-t4001-t4034);
t6350 = t4645.*t6105;
t6353 = -t6104.*(t1751+t2308+t964.*(t105-t465)+t1430.*(t103-t544));
t6355 = t4672.*t6089;
t6358 = t4686.*t6089;
t6359 = -t6090.*(t995+t1064-t1506+t1598-t1763-t1774);
t6360 = t4695.*t6089;
t6362 = t6090.*(t995+t1064-t1506+t1598-t1763-t1774);
t6363 = -t6090.*(t820+t1121-t1435+t1997+t2000+t11.*t420.*(t214-t541));
t6364 = t4672.*t6104;
t6366 = t6090.*(t820+t1121-t1435+t1997+t2000+t11.*t420.*(t214-t541));
t6367 = t4686.*t6104;
t6368 = -t6089.*(t1260-t1328-t1427-t1441+t1706+t9.*t870.*(t105-t465));
t6371 = -t5022.*(t2449.*3.36554e-3+t3490+t3544+t3545-t4001-t4034);
t6373 = -t6369;
t6375 = -t6105.*(t995+t1064-t1506+t1598-t1763-t1774);
t6378 = -t6105.*(t820+t1121-t1435+t1997+t2000+t11.*t420.*(t214-t541));
t6379 = t6105.*(t820+t1121-t1435+t1997+t2000+t11.*t420.*(t214-t541));
t6380 = -t6089.*(t753+t991-t1771-t1957+t1181.*(t105-t465)+t11.*t381.*(t534-t546));
t6381 = -t6090.*(t1064+t1137-t1694+t1698-t1763-t1774);
t6382 = t6090.*(t1064+t1137-t1694+t1698-t1763-t1774);
t6383 = -t6090.*(t867+t1059-t1646-t1705+t1938-t2002);
t6386 = -t6104.*(t753+t991-t1771-t1957+t1181.*(t105-t465)+t11.*t381.*(t534-t546));
t6387 = t4738.*t6090;
t6392 = -t6105.*(t867+t1059-t1646-t1705+t1938-t2002);
t6394 = -t6391;
t6395 = -t6091.*(t2436-t2536+t1510.*(t197-t537)+t1505.*(t214-t541));
t6396 = t6091.*(t2436-t2536+t1510.*(t197-t537)+t1505.*(t214-t541));
t6397 = t3339+t3804+t4478+t4480+t4556+t4563;
t6398 = t4770.*t6090;
t6401 = -t6400;
t6402 = t4785.*t6091;
t6403 = -t6106.*(t2436-t2536+t1510.*(t197-t537)+t1505.*(t214-t541));
t6404 = t6089.*(t1079+t1956-t4277-t1178.*(t105-t465));
t6407 = t4785.*t6106;
t6408 = -t6089.*(t1185+t1813-t4313+t1047.*(t105-t465));
t6411 = t6104.*(t1079+t1956-t4277-t1178.*(t105-t465));
t6412 = t4820.*t6089;
t6414 = t4821.*t6091;
t6416 = -t6105.*(t1060+t1138-t1883+t1932+t2088+t1179.*(t103-t544));
t6418 = -t6104.*(t1185+t1813-t4313+t1047.*(t105-t465));
t6420 = t4823.*t6091;
t6423 = -t4785.*(-t1865+t1970+t2708+t3161-t3236-t3845-t3870+t1240.*(t105-t465).*3.36554e-3+t903.*(t534-t546).*3.36554e-3);
t6424 = -t6105.*(t1250-t1261+t1761-t2083-t2111+t1037.*(t103-t544));
t6425 = t4830.*t6091;
t6426 = t4820.*t6104;
t6427 = t6105.*(t1250-t1261+t1761-t2083-t2111+t1037.*(t103-t544));
t6428 = t4821.*t6106;
t6429 = -t6105.*(t1053+t1332+t2368+t817.*(t214-t541)+t977.*(t103-t544)+t1512.*(t105-t465));
t6432 = t6105.*(t1053+t1332+t2368+t817.*(t214-t541)+t977.*(t103-t544)+t1512.*(t105-t465));
t6435 = t4830.*t6106;
t6436 = -t6106.*(-t1129+t1139-t2082+t2110+t2123+t8.*t872.*(t534-t546));
t6437 = -t6434;
t6438 = t4834.*t6106;
t6440 = -t4820.*(t1970-t1971+t2487+t3161-t3236-t3794-t3817+t1240.*(t105-t465).*3.372786875e-3+t903.*(t534-t546).*3.372786875e-3);
t6441 = t4849.*t6106;
t6442 = -t6439;
t6444 = -t6443;
t6445 = t4897.*t6091;
t6451 = t4923.*t6091;
t6452 = t4922.*t6091;
t6454 = t4922.*t6106;
t6456 = t2982+t2989+t3035+t3038+t3179+t3213+t3214+t3257+t3779+t3808+t3812+t3825;
t6457 = t2982+t2989+t3173+t3176+t3179+t3214+t3381+t3411+t3651+t3710+t3711+t3748;
t6458 = t3035+t3038+t3117+t3127+t3213+t3257+t3273+t3354+t3651+t3710+t3711+t3748;
t6461 = t4972.*t6106;
t6463 = -t6091.*(t1176-t1366+t2434+t2435-t2899+t1430.*(t539+t641));
t6464 = t5022.*t6091;
t6469 = -t4972.*(-t1865+t1970+t2708+t3161-t3236-t3845-t3870+t1240.*(t105-t465).*3.36554e-3+t903.*(t534-t546).*3.36554e-3);
t6470 = -t6106.*(t1176-t1366+t2434+t2435-t2899+t1430.*(t539+t641));
t6473 = t1160+t1211+t1621+t1659+t2817+t2853+t3925+t3958+t4029+t4053+t4377+t4380;
t6474 = t1164+t1200+t1621+t1659+t2792+t2882+t3925+t3958+t4035+t4046+t4377+t4380;
t6478 = t3961.*t6388;
t6479 = -t5022.*(-t1865+t1970+t2708+t3161-t3236-t3845-t3870+t1240.*(t105-t465).*3.36554e-3+t903.*(t534-t546).*3.36554e-3);
t6480 = -t6091.*(t1365-t1443+t2829-t2831-t2833+t1505.*(t534-t546));
t6481 = t6091.*(t1365-t1443+t2829-t2831-t2833+t1505.*(t534-t546));
t6488 = t3938.*t6399;
t6489 = -t6106.*(t1365-t1443+t2829-t2831-t2833+t1505.*(t534-t546));
t6491 = t6106.*(t1365-t1443+t2829-t2831-t2833+t1505.*(t534-t546));
t6498 = t4162.*t6389;
t6499 = t4173.*t6388;
t6500 = t3961.*t6409;
t6502 = -t6388.*(-t947+t1240.*(t105-t465)+t903.*(t534-t546));
t6503 = t3938.*t6422;
t6504 = t6388.*(-t947+t1240.*(t105-t465)+t903.*(t534-t546));
t6505 = t4277.*t6389;
t6507 = t4162.*t6410;
t6508 = t4173.*t6409;
t6509 = -t6409.*(-t1262+t1701+t9.*t868.*(t105-t465));
t6511 = t1415+t1529+t1656+t1721+t3091+t3171+t3945+t3984+t4092+t4109+t4386+t4389;
t6512 = -t6510;
t6513 = t1458+t1486+t1655+t1719+t3107+t3149+t3943+t3979+t4095+t4104+t4385+t4388;
t6516 = -t6388.*(t1332+t2368+t1512.*(t105-t465));
t6519 = -t6389.*(-t1331+t2317+t1510.*(t103-t544));
t6520 = t6388.*(t1332+t2368+t1512.*(t105-t465));
t6523 = t6389.*(-t1331+t2317+t1510.*(t103-t544));
t6525 = t4313.*t6410;
t6527 = t4392.*t6399;
t6529 = t4408.*t6399;
t6532 = -t6531;
t6533 = -t6409.*(t1332+t2368+t1512.*(t105-t465));
t6534 = -t6410.*(-t1331+t2317+t1510.*(t103-t544));
t6536 = t6410.*(-t1331+t2317+t1510.*(t103-t544));
t6540 = t4392.*t6422;
t6541 = dth1.*t6539;
t6542 = dth1.*t6538;
t6543 = t4476.*t6399;
t6547 = t4408.*t6422;
t6551 = t4447.*t6422;
t6561 = t3938.*t6487;
t6563 = t3961.*t6486;
t6569 = t4433+t4754+t4766+t5662;
t6572 = -t6486.*(-t1262+t1701+t9.*t868.*(t105-t465));
t6577 = -t6486.*(-t947+t1240.*(t105-t465)+t903.*(t534-t546));
t6578 = t4277.*t6485;
t6583 = t4313.*t6485;
t6585 = t1836+t1999+t2064+t2081+t2119+t2613+t2696+t2723+t2783+t3093+t3190+t3210+t3230+t3272+t3276+t3320+t3343;
t6586 = t1674+t2064+t2081+t2183+t2263+t2409+t2483+t2504+t2581+t3244+t3272+t3276+t3320+t3335+t3343+t3380+t3385;
t6587 = t1674+t1999+t2119+t2242+t2260+t2409+t2483+t2504+t2581+t3093+t3190+t3210+t3230+t3441+t3442+t3476+t3480;
t6590 = t1737+t1739+t1859+t2009+t3681+t3759+t4044+t4066+t4244+t4261+t4411+t4413;
t6591 = t1680+t1801+t1859+t2009+t3683+t3758+t4044+t4066+t4246+t4260+t4411+t4413;
t6592 = t1736+t1741+t1900+t1945+t3619+t3798+t4050+t4062+t4226+t4266+t4405+t4419;
t6593 = t1683+t1800+t1900+t1945+t3687+t3757+t4050+t4062+t4249+t4259+t4405+t4419;
t6598 = -t6486.*(t1332+t2368+t1512.*(t105-t465));
t6601 = -t6485.*(-t1331+t2317+t1510.*(t103-t544));
t6603 = t6485.*(-t1331+t2317+t1510.*(t103-t544));
t6604 = t2050+t2257+t2287+t2411+t2495+t2698+t2710+t2736+t2744+t2928+t3063+t3089+t3090+t3267+t3308+t3326+t3344;
t6605 = t4408.*t6487;
t6607 = t1888+t2399+t2411+t2430+t2485+t2492+t2495+t2522+t2535+t3063+t3085+t3089+t3243+t3267+t3308+t3482+t3485;
t6608 = t1888+t2257+t2287+t2485+t2492+t2522+t2535+t2624+t2722+t2928+t3090+t3204+t3233+t3326+t3344+t3406+t3463;
t6609 = t4447.*t6487;
t6610 = t4476.*t6487;
t6631 = t850+t1006+t1457+t1468+t1543+t1562+t1633+t2223+t2668+t3106+t3216+t3416+t3540+t3702+t4094+t4122+t4174+t4209;
t6632 = dy.*t6630;
t6654 = t847+t851+t1627+t1634+t1637+t1678+t1682+t1735+t2662+t2669+t3554+t3685+t3686+t3797+t4221+t4248+t4252+t4265;
t6658 = t3938.*t6613;
t6659 = dphi1.*t6656;
t6661 = t3961.*t6611;
t6664 = t3938.*t6617;
t6666 = t3938.*t6619;
t6668 = t3961.*t6615;
t6675 = t4173.*t6611;
t6676 = t4162.*t6612;
t6679 = -t6611.*(-t1262+t1701+t9.*t868.*(t105-t465));
t6682 = -t3938.*(t1832.*3.36554e-3+t1866.*3.372816795e-3-t1962+t1983+t2287-t2322-t2472+t2479+t2512+t2571+t2722+t2803+t3122+t3326+t3344-t3357+t3423+t496.*(t214-t541).*3.36554e-3);
t6683 = t6611.*(-t1262+t1701+t9.*t868.*(t105-t465));
t6684 = t4173.*t6614;
t6685 = t3961.*t6620;
t6686 = -t3961.*(t1832.*3.372786875e-3+t1866.*3.36554e-3-t1962+t2131+t2287+t2339-t2463+t2495+t2571-t2679+t2692+t2945+t2981-t3252+t3311+t3326+t3344+t496.*(t214-t541).*3.36554e-3);
t6689 = -t6614.*(-t1262+t1701+t9.*t868.*(t105-t465));
t6690 = t4173.*t6615;
t6691 = t4162.*t6616;
t6693 = t4162.*t6618;
t6694 = t3961.*(t1832.*3.372786875e-3+t1866.*3.36554e-3-t1962+t2131+t2287+t2339-t2463+t2495+t2571-t2679+t2692+t2945+t2981-t3252+t3311+t3326+t3344+t496.*(t214-t541).*3.36554e-3);
t6700 = -t6614.*(-t947+t1240.*(t105-t465)+t903.*(t534-t546));
t6701 = -t6615.*(-t947+t1240.*(t105-t465)+t903.*(t534-t546));
t6702 = t6615.*(-t947+t1240.*(t105-t465)+t903.*(t534-t546));
t6703 = t4277.*t6616;
t6704 = t4277.*t6618;
t6706 = t4313.*t6612;
t6710 = t4173.*t6620;
t6711 = -t4173.*(t1832.*3.372786875e-3+t1866.*3.36554e-3-t1962+t2131+t2287+t2339-t2463+t2495+t2571-t2679+t2692+t2945+t2981-t3252+t3311+t3326+t3344+t496.*(t214-t541).*3.36554e-3);
t6712 = -t4162.*(t1832.*3.36554e-3+t1866.*3.36554e-3+t1983-t2150-t2322+t2339+t2430-t2472+t2479+t2495+t2785+t2803+t2981-t3252+t3311+t3482+t3485+t496.*(t214-t541).*3.367829185e-3);
t6713 = -t6620.*(-t1262+t1701+t9.*t868.*(t105-t465));
t6714 = t4173.*(t1832.*3.372786875e-3+t1866.*3.36554e-3-t1962+t2131+t2287+t2339-t2463+t2495+t2571-t2679+t2692+t2945+t2981-t3252+t3311+t3326+t3344+t496.*(t214-t541).*3.36554e-3);
t6715 = t4162.*(t1832.*3.36554e-3+t1866.*3.36554e-3+t1983-t2150-t2322+t2339+t2430-t2472+t2479+t2495+t2785+t2803+t2981-t3252+t3311+t3482+t3485+t496.*(t214-t541).*3.367829185e-3);
t6716 = t4313.*t6618;
t6718 = (-t947+t1240.*(t105-t465)+t903.*(t534-t546)).*(t1832.*3.372786875e-3+t1866.*3.36554e-3-t1962+t2131+t2287+t2339-t2463+t2495+t2571-t2679+t2692+t2945+t2981-t3252+t3311+t3326+t3344+t496.*(t214-t541).*3.36554e-3);
t6720 = -t6611.*(t1332+t2368+t1512.*(t105-t465));
t6721 = t4392.*t6613;
t6722 = -t4277.*(t1832.*3.36554e-3+t1866.*3.36554e-3+t1983-t2150-t2322+t2339+t2430-t2472+t2479+t2495+t2785+t2803+t2981-t3252+t3311+t3482+t3485+t496.*(t214-t541).*3.367829185e-3);
t6723 = -t6612.*(-t1331+t2317+t1510.*(t103-t544));
t6724 = -t6614.*(t1332+t2368+t1512.*(t105-t465));
t6725 = t4408.*t6613;
t6726 = -t6615.*(t1332+t2368+t1512.*(t105-t465));
t6727 = t4392.*t6617;
t6728 = t4392.*t6619;
t6730 = t6615.*(t1332+t2368+t1512.*(t105-t465));
t6731 = -t6616.*(-t1331+t2317+t1510.*(t103-t544));
t6732 = t4447.*t6613;
t6733 = t3938.*t6637;
t6734 = t4408.*t6617;
t6736 = t3961.*t6635;
t6737 = t4447.*t6619;
t6738 = -t6620.*(t1332+t2368+t1512.*(t105-t465));
t6740 = (t1332+t2368+t1512.*(t105-t465)).*(t1832.*3.372786875e-3+t1866.*3.36554e-3-t1962+t2131+t2287+t2339-t2463+t2495+t2571-t2679+t2692+t2945+t2981-t3252+t3311+t3326+t3344+t496.*(t214-t541).*3.36554e-3);
t6741 = -t4392.*(t1832.*3.36554e-3+t1866.*3.372816795e-3-t1962+t1983+t2287-t2322-t2472+t2479+t2512+t2571+t2722+t2803+t3122+t3326+t3344-t3357+t3423+t496.*(t214-t541).*3.36554e-3);
t6742 = -t6739;
t6744 = (-t1331+t2317+t1510.*(t103-t544)).*(t1832.*3.36554e-3+t1866.*3.36554e-3+t1983-t2150-t2322+t2339+t2430-t2472+t2479+t2495+t2785+t2803+t2981-t3252+t3311+t3482+t3485+t496.*(t214-t541).*3.367829185e-3);
t6746 = t4476.*t6617;
t6747 = t4476.*t6619;
t6748 = -t4408.*(t1832.*3.36554e-3+t1866.*3.372816795e-3-t1962+t1983+t2287-t2322-t2472+t2479+t2512+t2571+t2722+t2803+t3122+t3326+t3344-t3357+t3423+t496.*(t214-t541).*3.36554e-3);
t6750 = t4162.*t6636;
t6751 = t4173.*t6635;
t6757 = -t6635.*(-t947+t1240.*(t105-t465)+t903.*(t534-t546));
t6758 = t6635.*(-t947+t1240.*(t105-t465)+t903.*(t534-t546));
t6759 = t4277.*t6636;
t6760 = -t4476.*(t1832.*3.36554e-3+t1866.*3.372816795e-3-t1962+t1983+t2287-t2322-t2472+t2479+t2512+t2571+t2722+t2803+t3122+t3326+t3344-t3357+t3423+t496.*(t214-t541).*3.36554e-3);
t6761 = t4476.*(t1832.*3.36554e-3+t1866.*3.372816795e-3-t1962+t1983+t2287-t2322-t2472+t2479+t2512+t2571+t2722+t2803+t3122+t3326+t3344-t3357+t3423+t496.*(t214-t541).*3.36554e-3);
t6765 = -t6635.*(t1332+t2368+t1512.*(t105-t465));
t6766 = t4392.*t6637;
t6767 = -t6636.*(-t1331+t2317+t1510.*(t103-t544));
t6768 = t6636.*(-t1331+t2317+t1510.*(t103-t544));
t6769 = t4408.*t6637;
t6774 = t4476.*t6637;
t6778 = -t6776;
t6785 = t4871+t4884+t5660+t5824;
t6797 = t4188+t4295+t4304+t4746+t4999+t6555+t6629;
t4543 = -t4540;
t4631 = -t4627;
t4640 = -t4633;
t4648 = -t4642;
t4650 = -t4644;
t4691 = -t4688;
t4797 = -t4792;
t4819 = -t4817;
t4868 = t1695+t1752+t3849+t3895;
t4869 = t1155+t1788+t1890+t4417;
t4893 = -t4886;
C = ft_13({B_cg_H,ITail,Mb,Mm,Mt,T_cg_H,dphi1,dphi2,dpsi1,dth1,dth2,dx,dy,dz,t10,t1005,t1007,t1008,t1009,t1013,t1016,t1017,t1018,t1019,t1023,t1029,t103,t1037,t1047,t105,t1050,t1053,t1059,t1060,t1064,t1071,t1072,t1075,t1078,t1079,t1084,t1086,t1088,t1097,t1099,t11,t1102,t1108,t1113,t1121,t1129,t1135,t1137,t1138,t1139,t1141,t1142,t1143,t1147,t1149,t1153,t1157,t1159,t1167,t1169,t1170,t1173,t1176,t1178,t1179,t1181,t1185,t1186,t1189,t1193,t1194,t1195,t1196,t120,t1203,t1205,t1206,t1215,t1221,t1223,t1224,t1225,t1228,t1229,t1230,t1234,t1240,t1242,t1245,t1246,t1247,t1250,t1252,t1253,t1255,t1260,t1261,t1262,t1264,t1265,t1268,t1280,t1283,t1291,t130,t1301,t1302,t1303,t1304,t1305,t1307,t1309,t1322,t1328,t1331,t1332,t1334,t1337,t1338,t134,t1343,t1344,t1345,t1348,t1352,t1354,t1355,t1360,t1362,t1365,t1366,t1368,t1370,t1371,t1373,t1374,t1378,t1381,t1382,t1384,t1386,t1388,t1389,t1391,t1393,t1394,t1395,t1396,t1397,t1412,t1413,t1415,t1421,t1426,t1427,t1430,t1431,t1433,t1435,t144,t1441,t1443,t1444,t1446,t1453,t1455,t1456,t1458,t1460,t1465,t1466,t1470,t1481,t1486,t1487,t1495,t15,t1505,t1506,t1510,t1512,t1513,t1518,t1521,t1525,t1526,t1528,t1529,t1531,t1535,t1540,t1544,t1552,t1558,t1568,t1575,t1578,t1581,t1586,t1593,t1596,t1597,t1598,t1609,t161,t1612,t1618,t1619,t162,t1620,t1624,t1628,t1635,t1639,t1640,t1645,t1646,t1651,t1652,t1654,t1657,t1660,t1661,t1664,t1665,t1667,t1672,t1676,t1681,t1685,t1692,t1693,t1694,t1698,t1701,t1702,t1703,t1705,t1706,t1718,t1720,t1722,t1725,t1727,t1730,t1734,t1735,t1742,t1746,t1747,t1751,t1759,t1761,t1763,t1764,t1771,t1774,t1777,t1778,t1779,t1784,t1785,t1786,t1787,t1789,t1790,t1792,t1799,t1802,t1806,t1809,t1810,t1813,t1832,t1840,t1843,t1846,t1851,t1853,t1855,t1857,t1858,t1860,t1865,t1866,t1867,t1882,t1883,t1896,t1898,t1899,t1907,t1910,t1915,t1917,t1918,t1928,t1929,t1932,t1938,t1939,t1942,t195,t1952,t1956,t1957,t1959,t1962,t1964,t1965,t197,t1970,t1971,t1974,t1976,t1977,t1979,t1981,t1983,t1993,t1997,t2,t2000,t2002,t2007,t2008,t2013,t2015,t2016,t2020,t2023,t2024,t2032,t2037,t2038,t2047,t2049,t2057,t2058,t2059,t2061,t2062,t2064,t2065,t2067,t2068,t2069,t2072,t2075,t2076,t2082,t2083,t2086,t2087,t2088,t2096,t2104,t2106,t2107,t2108,t2110,t2111,t2113,t2117,t2123,t2131,t2134,t2135,t2137,t2139,t214,t2141,t2147,t2148,t2150,t2152,t2153,t2155,t2156,t2158,t2161,t2174,t2175,t2188,t2189,t2190,t2191,t2192,t2196,t2197,t2202,t2203,t2206,t2208,t2210,t2212,t2215,t2218,t2220,t2222,t2225,t2227,t2237,t2240,t2241,t2242,t2243,t2247,t2248,t2254,t2259,t2268,t2269,t2271,t2274,t2276,t2281,t2282,t2285,t2286,t2287,t2289,t2293,t2305,t2308,t2312,t2316,t2317,t2319,t2322,t2325,t2329,t2334,t2336,t2338,t2339,t2341,t2342,t2345,t2347,t2348,t2352,t2360,t2361,t2364,t2368,t2376,t2387,t2388,t2389,t2390,t2391,t2397,t24,t2401,t2404,t2406,t2409,t2410,t2412,t2413,t2419,t2420,t2426,t2427,t2430,t2434,t2435,t2436,t2438,t2447,t2449,t2458,t2463,t2465,t2468,t2471,t2472,t2479,t2483,t2487,t2489,t2495,t2496,t25,t2501,t2503,t2504,t2512,t2514,t2516,t2518,t2524,t2526,t2527,t2528,t2536,t2547,t2563,t2564,t2567,t2568,t2569,t2571,t2573,t2574,t2576,t2578,t2579,t2582,t2587,t2589,t259,t2590,t2591,t2597,t26,t260,t2600,t2605,t2613,t2616,t2617,t2621,t2627,t2632,t2636,t2637,t2638,t2646,t2657,t2660,t2663,t2665,t2667,t2669,t2679,t2684,t2688,t2692,t2696,t2699,t27,t2700,t2706,t2708,t2712,t2715,t2717,t2718,t2722,t2723,t2728,t2730,t2733,t2734,t2735,t2737,t2738,t2743,t2746,t2754,t2759,t276,t2763,t277,t2778,t2785,t2787,t2790,t2791,t2794,t2796,t2797,t2798,t2799,t2803,t2805,t2811,t2816,t2818,t2819,t2821,t2823,t2824,t2825,t2829,t283,t2831,t2833,t2834,t2836,t2839,t284,t2842,t2843,t2844,t2845,t2847,t2849,t285,t286,t2860,t2861,t2868,t287,t2871,t2875,t2876,t2877,t2878,t2879,t288,t2883,t2887,t2889,t289,t2899,t290,t291,t2912,t2913,t2914,t2915,t2917,t2918,t292,t2920,t2921,t2927,t293,t2930,t2936,t2937,t294,t2942,t2944,t2945,t2950,t2952,t2956,t2962,t2963,t2965,t2970,t2972,t2977,t2978,t2981,t2994,t2996,t2997,t3,t3008,t3009,t3012,t3022,t3027,t3030,t3031,t3034,t304,t3040,t3050,t3054,t3062,t3064,t3070,t3076,t3080,t3082,t3084,t3086,t3087,t3091,t3093,t3094,t3096,t3105,t3107,t3109,t3110,t3113,t3121,t3122,t3131,t3138,t3139,t3147,t3149,t3155,t3160,t3161,t3167,t3169,t3170,t3171,t3177,t3178,t3180,t3186,t3192,t3199,t3206,t3207,t3222,t3232,t3235,t3236,t3244,t3247,t3248,t3252,t3256,t3261,t3262,t3263,t3265,t3266,t3270,t3276,t3278,t3286,t3287,t3289,t3299,t3302,t3304,t3307,t3311,t3312,t3315,t3321,t3325,t3326,t3329,t3330,t3331,t3333,t3341,t3344,t3347,t3357,t3378,t3379,t3387,t3390,t3391,t3392,t3397,t3403,t3407,t3412,t3413,t3414,t3415,t3419,t3423,t3424,t3427,t3431,t3432,t3433,t3437,t3438,t3439,t3442,t3445,t3448,t3449,t3458,t3460,t3467,t3471,t3475,t3481,t3482,t3483,t3485,t3486,t3487,t3489,t3490,t3494,t3499,t3501,t3504,t3506,t3510,t3512,t3516,t3521,t3522,t3523,t3524,t3526,t3528,t3529,t3530,t3531,t3534,t3541,t3543,t3544,t3545,t3548,t3550,t3552,t3553,t3556,t3557,t3563,t3575,t3576,t3578,t3582,t3583,t3584,t3587,t3594,t3597,t3598,t3600,t3602,t3609,t3614,t3617,t3621,t3627,t3632,t3634,t3638,t3644,t3647,t3648,t3649,t3652,t3657,t3659,t3661,t3667,t3671,t3672,t3678,t3679,t3680,t3682,t3684,t3697,t3698,t3701,t3704,t3709,t3716,t3719,t3720,t3721,t3722,t3724,t3735,t3738,t3739,t3744,t3745,t3746,t3749,t3750,t3756,t376,t3764,t3769,t377,t3770,t3771,t3772,t3773,t3774,t3777,t3780,t3784,t3787,t3791,t3792,t3793,t3794,t3802,t381,t3811,t3814,t3815,t3817,t382,t3823,t3827,t3828,t383,t3832,t3834,t3836,t3837,t3841,t3845,t3847,t3848,t3851,t3855,t3856,t3858,t3859,t3862,t3868,t3870,t3879,t3880,t3882,t3883,t3889,t390,t3902,t3903,t3906,t3907,t3908,t3909,t3912,t3915,t3916,t3920,t3921,t3923,t3926,t3928,t3929,t3930,t3931,t3932,t3933,t3934,t3936,t3937,t3938,t3939,t394,t3940,t3944,t3947,t3948,t3949,t3950,t3951,t3952,t3953,t3954,t3955,t3956,t3957,t3959,t3960,t3961,t3962,t3964,t3965,t3966,t3967,t3969,t3971,t3972,t3973,t3974,t3975,t3976,t3977,t3980,t3981,t3982,t3983,t3985,t3986,t3992,t3993,t3995,t3996,t3998,t4,t4000,t4001,t4003,t4005,t4006,t4007,t4008,t4009,t4010,t4012,t4014,t4018,t4019,t4020,t4023,t4024,t4025,t4026,t4027,t4028,t4033,t4034,t4036,t4037,t4038,t4039,t4041,t4042,t4047,t4048,t4051,t4052,t4054,t4056,t4058,t4059,t4061,t4064,t4065,t4068,t4070,t4071,t4072,t4073,t4074,t4077,t4078,t4081,t4083,t4084,t4085,t4086,t4087,t4089,t4090,t4091,t4092,t4095,t4096,t4097,t4098,t4099,t410,t4100,t4104,t4105,t4107,t4108,t4109,t411,t4111,t4112,t4115,t4116,t4117,t4119,t412,t4120,t4121,t4126,t4127,t4129,t413,t4132,t4133,t4135,t4137,t4138,t4139,t414,t4140,t4141,t4143,t4144,t4145,t4147,t415,t4152,t4153,t4154,t4155,t4156,t4160,t4162,t4164,t4165,t4169,t4170,t4171,t4173,t4179,t4182,t4183,t4184,t4186,t4187,t4189,t4190,t4196,t4197,t420,t4200,t4201,t4204,t4205,t4206,t4208,t421,t4210,t4211,t4212,t4213,t4214,t4215,t4216,t4217,t4218,t4219,t4220,t4222,t4223,t4224,t4225,t4227,t4228,t4231,t4232,t4233,t4234,t4236,t4237,t4238,t4239,t4240,t4241,t4243,t4245,t4247,t425,t4250,t4253,t4255,t4256,t4257,t4258,t4262,t4263,t4268,t4269,t4271,t4272,t4273,t4274,t4276,t4277,t4278,t4280,t4281,t4282,t4286,t4291,t4296,t430,t4300,t4301,t4302,t4303,t4305,t4307,t4309,t431,t4310,t4311,t4312,t4313,t4314,t4315,t4316,t4317,t4318,t4319,t4320,t4321,t4322,t4323,t4324,t4326,t4327,t4329,t433,t4330,t4331,t4332,t4333,t4334,t4337,t4339,t4340,t4341,t4342,t4343,t4344,t4345,t4346,t4348,t4349,t4350,t4352,t4354,t4355,t4356,t4357,t4358,t4359,t436,t4360,t4361,t4365,t4367,t4368,t4369,t4370,t4371,t4372,t4373,t4374,t4375,t4376,t4378,t4379,t4382,t4384,t4391,t4392,t4393,t4394,t4395,t4397,t4398,t4399,t44,t4400,t4401,t4402,t4403,t4404,t4406,t4407,t4408,t4409,t4412,t4414,t4415,t4416,t4418,t4420,t4421,t4422,t4424,t4425,t4427,t4428,t4429,t4431,t4432,t4434,t4435,t4437,t4438,t4439,t4440,t4442,t4443,t4444,t4447,t4448,t4449,t445,t4450,t4451,t4452,t4453,t4454,t4455,t4456,t4457,t4458,t4459,t4460,t4461,t4462,t4463,t4465,t4467,t4469,t4470,t4471,t4472,t4473,t4475,t4476,t4477,t4479,t4480,t4481,t4482,t4483,t4484,t4485,t4486,t4487,t4488,t4489,t4490,t4492,t4493,t4495,t4496,t4497,t4498,t4500,t4501,t4502,t4503,t4505,t4506,t4507,t451,t4510,t4511,t4512,t4514,t4515,t4517,t4518,t4519,t4521,t4522,t4523,t4525,t4526,t4528,t4529,t4531,t4532,t4533,t4535,t4536,t4537,t4538,t4540,t4541,t4542,t4543,t4544,t4545,t4546,t4547,t4549,t4550,t4551,t4552,t4553,t4554,t4555,t4556,t4557,t4558,t4559,t4560,t4561,t4562,t4565,t4566,t4567,t4568,t4570,t4571,t4573,t4574,t4575,t4576,t4577,t4578,t4579,t4580,t4581,t4582,t4583,t4584,t4585,t4586,t4588,t459,t4590,t4591,t4592,t4596,t4597,t4598,t4600,t4601,t4602,t4603,t4604,t4605,t4606,t4607,t4608,t4609,t4610,t4613,t4614,t4615,t4616,t4617,t4618,t4619,t4620,t4621,t4622,t4623,t4624,t4625,t4626,t4629,t4630,t4631,t4634,t4635,t4636,t4637,t4638,t4639,t4640,t4644,t4645,t4646,t4647,t4648,t4649,t465,t4650,t4651,t4652,t4655,t4656,t4657,t4658,t4659,t4660,t4661,t4662,t4663,t4664,t4665,t4666,t4667,t4668,t4669,t4672,t4673,t4674,t4675,t4678,t4679,t4680,t4681,t4682,t4684,t4685,t4686,t4689,t4690,t4691,t4693,t4694,t4695,t4696,t4697,t4698,t4700,t4701,t4702,t4704,t4705,t4706,t4707,t4708,t4709,t4710,t4711,t4712,t4713,t4722,t4723,t4724,t4727,t4729,t4732,t4733,t4735,t4736,t4737,t4738,t4742,t4750,t4751,t4752,t4753,t4755,t4756,t4758,t4759,t4761,t4764,t4765,t4769,t4770,t4771,t4772,t4773,t4775,t4776,t4780,t4783,t4784,t4785,t4786,t4787,t4788,t4789,t4790,t4791,t4793,t4796,t4797,t4799,t48,t4800,t4801,t4802,t4803,t4804,t4805,t4806,t4807,t4809,t4811,t4813,t4814,t4815,t4816,t4819,t4820,t4821,t4823,t4826,t4827,t4830,t4832,t4834,t4835,t4836,t4838,t4840,t4841,t4843,t4845,t4846,t4847,t4848,t4849,t485,t4850,t4851,t4852,t4853,t4857,t4858,t4861,t4862,t4863,t4864,t4865,t4867,t4868,t4870,t4873,t4874,t4877,t488,t4880,t4881,t4882,t4883,t4887,t4888,t4889,t4890,t4892,t4893,t4895,t4897,t4899,t49,t4900,t4901,t4904,t4906,t4907,t4908,t4909,t4911,t4912,t4913,t4914,t4916,t4917,t4922,t4923,t4924,t4925,t4926,t4927,t4928,t4929,t4931,t4932,t4933,t4934,t4936,t4937,t4938,t4939,t4940,t4941,t4942,t4943,t4944,t4945,t4946,t4947,t4949,t4950,t4951,t4952,t4953,t4954,t4955,t496,t4960,t4961,t4963,t4964,t4966,t4967,t4968,t4969,t4972,t4973,t4975,t4976,t4977,t4978,t4980,t4981,t4982,t4983,t4984,t4985,t4986,t4988,t4989,t4990,t4993,t4995,t4997,t4998,t5,t50,t5000,t5001,t5002,t5004,t5005,t5006,t5007,t5008,t5009,t501,t5010,t5012,t5013,t5014,t5016,t5017,t5018,t502,t5021,t5022,t5023,t5024,t5025,t5027,t5028,t5030,t5031,t5032,t5033,t5034,t5035,t5036,t5038,t5039,t504,t5040,t5041,t5042,t5045,t5046,t5047,t5048,t5049,t5050,t5051,t5052,t5053,t5054,t5055,t5057,t5058,t5059,t5061,t5062,t5063,t5064,t5066,t5067,t5068,t5069,t5071,t5072,t5074,t5075,t5076,t5077,t5078,t5079,t5080,t5082,t5083,t5084,t5085,t5087,t5088,t5089,t5090,t5092,t5093,t5094,t5095,t5098,t5099,t51,t5100,t5101,t5102,t5103,t5104,t5106,t5107,t5109,t5110,t5111,t5112,t5114,t5115,t5117,t5118,t5120,t5121,t5123,t5124,t5126,t5128,t5131,t5132,t5134,t5135,t5136,t5137,t5138,t5139,t5140,t5142,t5143,t5144,t5145,t5146,t5148,t5149,t5150,t5152,t5153,t5154,t5155,t5156,t5157,t5158,t5161,t5162,t5163,t5165,t5166,t5167,t5168,t5169,t5171,t5172,t5173,t5174,t5175,t5177,t5178,t5179,t5180,t5182,t5183,t5184,t5185,t5186,t5187,t5188,t519,t5190,t5191,t5193,t5194,t5196,t5197,t5198,t5199,t5202,t5203,t5204,t5205,t5206,t5207,t5208,t5211,t5212,t5214,t5216,t5217,t5218,t5220,t5221,t5223,t5224,t5225,t5226,t5227,t5228,t5229,t523,t5231,t5232,t5233,t5234,t5235,t5238,t5239,t524,t5240,t5241,t5243,t5244,t5245,t5247,t5248,t5249,t5250,t5251,t5252,t5253,t5254,t5256,t5259,t5260,t5262,t5263,t5264,t5265,t5266,t5268,t5269,t527,t5270,t5272,t5274,t5275,t5276,t5277,t5279,t5280,t5281,t5284,t5285,t5286,t5287,t5288,t5289,t5290,t5291,t5292,t5293,t5294,t5295,t5296,t5297,t5298,t5299,t530,t5300,t5301,t5302,t5304,t5305,t5306,t5307,t5308,t5309,t5310,t5311,t5312,t5313,t5314,t5316,t5317,t5318,t5319,t5321,t5322,t5324,t5325,t5326,t5327,t5328,t5329,t5330,t5332,t5333,t5335,t5336,t5337,t5338,t5339,t534,t5340,t5341,t5343,t5344,t5345,t5346,t5347,t5349,t5350,t5351,t5352,t5353,t5354,t5356,t5357,t5358,t5359,t5360,t5361,t5363,t5364,t5366,t5368,t5369,t537,t5370,t5371,t5372,t5374,t5376,t5377,t5378,t5379,t5380,t5381,t5382,t5383,t5384,t5385,t5386,t5388,t5389,t539,t5391,t5392,t5393,t5394,t5395,t5396,t5398,t5399,t54,t5400,t5402,t5403,t5404,t5405,t5406,t5407,t5408,t5409,t541,t5411,t5412,t5413,t5414,t5415,t5416,t5417,t5418,t5419,t542,t5420,t5421,t5422,t5423,t5425,t5426,t5427,t5428,t5430,t5431,t5434,t5435,t5436,t5438,t5439,t544,t5441,t5442,t5443,t5444,t5447,t5448,t5449,t5450,t5452,t5453,t5455,t5456,t5458,t5459,t546,t5460,t5461,t5462,t5463,t5464,t5465,t5467,t5468,t5470,t5471,t5474,t5475,t5476,t5478,t5480,t5481,t5483,t5484,t5486,t5487,t5488,t5489,t5490,t5492,t5493,t5494,t5495,t5496,t5497,t5498,t5499,t55,t550,t5500,t5502,t5508,t5509,t5510,t5511,t5513,t5514,t5515,t5516,t5519,t5520,t5521,t5523,t5524,t5527,t5528,t553,t5530,t5531,t5532,t5533,t5534,t5535,t5536,t5538,t5539,t5541,t5542,t5543,t5544,t5545,t5546,t5547,t5548,t5549,t5551,t5552,t5553,t5554,t5555,t5556,t5557,t5558,t5560,t5561,t5565,t5566,t5569,t557,t5570,t5571,t5573,t5574,t5575,t5576,t5577,t5578,t558,t5581,t5582,t5584,t5585,t5586,t5588,t5589,t5590,t5591,t5592,t5593,t5594,t5597,t5598,t5599,t56,t5600,t5601,t5602,t5603,t5604,t5606,t5607,t5609,t5611,t5613,t5615,t5616,t5617,t5618,t5619,t5620,t5621,t5622,t5623,t5624,t5625,t5627,t5628,t5629,t5630,t5631,t5632,t5633,t5634,t5635,t5636,t5637,t5638,t5640,t5641,t5642,t5643,t5644,t5648,t5649,t5653,t5656,t5657,t5658,t5659,t5660,t5661,t5663,t5664,t5665,t5667,t5668,t5669,t5670,t5672,t5674,t5675,t5677,t5678,t5679,t5681,t5682,t5683,t5684,t5685,t5687,t5688,t5689,t5690,t5691,t5692,t5694,t5695,t5696,t5697,t5698,t5699,t5700,t5701,t5704,t5705,t5706,t5707,t5709,t5711,t5712,t5713,t5714,t5715,t5717,t5718,t5719,t5720,t5723,t5724,t5725,t5726,t5727,t5728,t5729,t573,t5730,t5731,t5732,t5733,t5734,t5735,t5737,t5738,t5739,t574,t5742,t5743,t5745,t5746,t5748,t5749,t575,t5750,t5753,t5754,t5755,t5756,t5758,t5759,t5760,t5762,t5763,t5765,t5766,t5767,t5768,t5769,t5770,t5771,t5772,t5774,t5775,t5776,t5778,t5779,t5780,t5781,t5782,t5783,t5785,t5786,t5788,t5789,t5791,t5792,t5793,t5795,t5797,t5798,t5799,t5800,t5801,t5802,t5803,t5805,t5807,t5808,t5809,t5811,t5813,t5814,t5815,t5820,t5821,t5823,t5824,t5826,t5827,t5828,t5829,t5831,t5832,t5833,t5834,t5835,t5836,t5837,t5838,t5839,t5840,t5841,t5843,t5845,t5846,t5847,t5850,t5852,t5853,t5855,t5856,t5857,t5858,t5862,t5863,t5865,t5867,t5868,t5869,t587,t5870,t5871,t5872,t5873,t5874,t5875,t5880,t5881,t5883,t5885,t5887,t5889,t5890,t5891,t5894,t5895,t5898,t59,t5901,t5902,t5904,t5905,t5908,t5909,t5910,t5911,t5912,t5913,t5914,t5915,t5916,t5917,t5919,t5920,t5921,t5924,t5925,t5926,t5928,t5930,t5932,t5933,t5935,t5936,t5937,t5938,t5939,t5941,t5945,t5946,t5947,t5948,t5949,t595,t5951,t5953,t5955,t5956,t5958,t5959,t5960,t5962,t5963,t5964,t5965,t5968,t5969,t5970,t5971,t5972,t5973,t5974,t5975,t5976,t5977,t5978,t5980,t5981,t5982,t5983,t5984,t5985,t5986,t5987,t5988,t5989,t5990,t5991,t5992,t5993,t5994,t5995,t5996,t5998,t6000,t6002,t6004,t6006,t6008,t6010,t6011,t6013,t6014,t6016,t6018,t6021,t6022,t6023,t6024,t6027,t6028,t6029,t603,t6030,t6031,t6032,t6036,t6037,t6039,t6042,t6043,t6045,t6049,t6051,t6052,t6054,t6057,t6058,t6059,t6060,t6062,t6064,t6066,t6069,t6071,t6073,t6074,t6075,t6079,t6086,t6088,t6089,t6090,t6091,t6092,t6095,t6099,t61,t6101,t6103,t6104,t6105,t6106,t6110,t6113,t6114,t6116,t6117,t6118,t6124,t6125,t6127,t6128,t6129,t6137,t6138,t614,t6140,t6143,t6144,t6150,t6158,t6160,t6161,t6164,t6166,t6171,t6174,t6176,t6181,t6182,t6183,t6184,t6188,t6189,t6190,t6191,t6195,t6196,t6197,t6199,t6201,t6202,t6203,t6204,t6205,t6206,t6207,t6208,t6210,t6211,t6212,t6216,t6217,t6218,t6219,t6220,t6221,t6222,t6223,t6224,t6225,t6228,t6229,t6230,t6231,t6233,t6234,t6235,t6236,t6238,t6239,t6240,t6241,t6243,t6245,t6248,t6249,t6250,t6251,t6252,t6253,t6255,t6257,t6258,t6259,t6260,t6261,t6264,t6265,t6269,t6271,t6272,t6273,t6274,t6276,t6277,t6278,t6279,t628,t6280,t6281,t6282,t6283,t6284,t6285,t6286,t6289,t629,t6290,t6293,t6294,t6295,t6296,t6298,t6299,t6302,t6303,t6304,t6305,t6307,t6309,t6310,t6311,t6314,t6315,t6316,t6317,t6319,t6322,t6323,t6324,t6325,t6328,t6330,t6332,t6333,t6334,t6335,t6336,t6337,t6339,t634,t6340,t6341,t6343,t6344,t6345,t6346,t6347,t6348,t6349,t6350,t6351,t6353,t6354,t6355,t6356,t6358,t6360,t6361,t6362,t6364,t6365,t6366,t6367,t6368,t6369,t6370,t6371,t6372,t6373,t6375,t6378,t6379,t6380,t6381,t6382,t6383,t6385,t6386,t6387,t6388,t6389,t6392,t6393,t6394,t6395,t6396,t6398,t6399,t6400,t6401,t6402,t6403,t6404,t6405,t6406,t6407,t6408,t6409,t641,t6410,t6411,t6412,t6413,t6414,t6416,t6418,t6420,t6421,t6422,t6423,t6425,t6426,t6427,t6428,t6430,t6432,t6433,t6434,t6435,t6436,t6437,t6438,t6440,t6441,t6442,t6444,t6445,t6446,t6447,t6448,t6449,t6450,t6451,t6452,t6454,t6455,t6456,t6457,t6458,t6460,t6461,t6463,t6464,t6469,t6470,t6471,t6473,t6474,t6478,t6479,t6481,t6482,t6483,t6484,t6485,t6486,t6487,t6488,t6491,t6495,t6497,t6498,t6499,t65,t6500,t6501,t6503,t6504,t6505,t6506,t6507,t6508,t6509,t651,t6511,t6512,t6513,t6520,t6523,t6525,t6526,t6527,t6529,t6532,t6533,t6536,t6540,t6541,t6542,t6543,t6547,t6549,t655,t6550,t6551,t6552,t6561,t6562,t6563,t6565,t6567,t6569,t657,t6571,t6572,t6577,t6578,t6580,t6581,t6583,t6584,t6588,t6590,t6591,t6592,t6593,t6598,t6602,t6603,t6604,t6605,t6607,t6608,t6609,t6610,t6611,t6612,t6613,t6614,t6615,t6616,t6617,t6618,t6619,t6620,t6631,t6632,t6634,t6635,t6636,t6637,t6638,t664,t6640,t6641,t6645,t6646,t6647,t665,t6653,t6654,t6658,t6659,t666,t6661,t6664,t6666,t6668,t6669,t667,t6673,t6675,t6676,t6677,t6679,t668,t6681,t6682,t6683,t6684,t6685,t6689,t669,t6690,t6691,t6693,t6694,t6699,t6700,t6701,t6702,t6703,t6704,t6706,t6709,t6710,t6713,t6714,t6715,t6716,t6718,t6720,t6721,t6722,t6723,t6724,t6725,t6727,t6728,t6729,t6730,t6731,t6732,t6733,t6734,t6736,t6737,t6738,t6740,t6741,t6742,t6743,t6744,t6745,t6746,t6747,t6748,t675,t6750,t6751,t6754,t6755,t6756,t6758,t6759,t6760,t6761,t6762,t6763,t6764,t6765,t6766,t6768,t6769,t6770,t6772,t6773,t6774,t6775,t6776,t6778,t6779,t6780,t6781,t6792,t6797,t6798,t68,t693,t7,t71,t721,t724,t73,t731,t732,t736,t741,t753,t754,t755,t757,t765,t769,t772,t774,t776,t778,t795,t797,t799,t8,t802,t803,t806,t817,t818,t820,t828,t831,t838,t843,t852,t853,t855,t865,t867,t868,t870,t871,t872,t876,t886,t888,t9,t901,t902,t903,t904,t907,t909,t914,t925,t926,t947,t949,t952,t964,t972,t977,t983,t991,t992,t993,t994,t995});
end
function C = ft_13(ct)
B_cg_H = ct{1};
ITail = ct{2};
Mb = ct{3};
Mm = ct{4};
Mt = ct{5};
T_cg_H = ct{6};
dphi1 = ct{7};
dphi2 = ct{8};
dpsi1 = ct{9};
dth1 = ct{10};
dth2 = ct{11};
dx = ct{12};
dy = ct{13};
dz = ct{14};
t10 = ct{15};
t1005 = ct{16};
t1007 = ct{17};
t1008 = ct{18};
t1009 = ct{19};
t1013 = ct{20};
t1016 = ct{21};
t1017 = ct{22};
t1018 = ct{23};
t1019 = ct{24};
t1023 = ct{25};
t1029 = ct{26};
t103 = ct{27};
t1037 = ct{28};
t1047 = ct{29};
t105 = ct{30};
t1050 = ct{31};
t1053 = ct{32};
t1059 = ct{33};
t1060 = ct{34};
t1064 = ct{35};
t1071 = ct{36};
t1072 = ct{37};
t1075 = ct{38};
t1078 = ct{39};
t1079 = ct{40};
t1084 = ct{41};
t1086 = ct{42};
t1088 = ct{43};
t1097 = ct{44};
t1099 = ct{45};
t11 = ct{46};
t1102 = ct{47};
t1108 = ct{48};
t1113 = ct{49};
t1121 = ct{50};
t1129 = ct{51};
t1135 = ct{52};
t1137 = ct{53};
t1138 = ct{54};
t1139 = ct{55};
t1141 = ct{56};
t1142 = ct{57};
t1143 = ct{58};
t1147 = ct{59};
t1149 = ct{60};
t1153 = ct{61};
t1157 = ct{62};
t1159 = ct{63};
t1167 = ct{64};
t1169 = ct{65};
t1170 = ct{66};
t1173 = ct{67};
t1176 = ct{68};
t1178 = ct{69};
t1179 = ct{70};
t1181 = ct{71};
t1185 = ct{72};
t1186 = ct{73};
t1189 = ct{74};
t1193 = ct{75};
t1194 = ct{76};
t1195 = ct{77};
t1196 = ct{78};
t120 = ct{79};
t1203 = ct{80};
t1205 = ct{81};
t1206 = ct{82};
t1215 = ct{83};
t1221 = ct{84};
t1223 = ct{85};
t1224 = ct{86};
t1225 = ct{87};
t1228 = ct{88};
t1229 = ct{89};
t1230 = ct{90};
t1234 = ct{91};
t1240 = ct{92};
t1242 = ct{93};
t1245 = ct{94};
t1246 = ct{95};
t1247 = ct{96};
t1250 = ct{97};
t1252 = ct{98};
t1253 = ct{99};
t1255 = ct{100};
t1260 = ct{101};
t1261 = ct{102};
t1262 = ct{103};
t1264 = ct{104};
t1265 = ct{105};
t1268 = ct{106};
t1280 = ct{107};
t1283 = ct{108};
t1291 = ct{109};
t130 = ct{110};
t1301 = ct{111};
t1302 = ct{112};
t1303 = ct{113};
t1304 = ct{114};
t1305 = ct{115};
t1307 = ct{116};
t1309 = ct{117};
t1322 = ct{118};
t1328 = ct{119};
t1331 = ct{120};
t1332 = ct{121};
t1334 = ct{122};
t1337 = ct{123};
t1338 = ct{124};
t134 = ct{125};
t1343 = ct{126};
t1344 = ct{127};
t1345 = ct{128};
t1348 = ct{129};
t1352 = ct{130};
t1354 = ct{131};
t1355 = ct{132};
t1360 = ct{133};
t1362 = ct{134};
t1365 = ct{135};
t1366 = ct{136};
t1368 = ct{137};
t1370 = ct{138};
t1371 = ct{139};
t1373 = ct{140};
t1374 = ct{141};
t1378 = ct{142};
t1381 = ct{143};
t1382 = ct{144};
t1384 = ct{145};
t1386 = ct{146};
t1388 = ct{147};
t1389 = ct{148};
t1391 = ct{149};
t1393 = ct{150};
t1394 = ct{151};
t1395 = ct{152};
t1396 = ct{153};
t1397 = ct{154};
t1412 = ct{155};
t1413 = ct{156};
t1415 = ct{157};
t1421 = ct{158};
t1426 = ct{159};
t1427 = ct{160};
t1430 = ct{161};
t1431 = ct{162};
t1433 = ct{163};
t1435 = ct{164};
t144 = ct{165};
t1441 = ct{166};
t1443 = ct{167};
t1444 = ct{168};
t1446 = ct{169};
t1453 = ct{170};
t1455 = ct{171};
t1456 = ct{172};
t1458 = ct{173};
t1460 = ct{174};
t1465 = ct{175};
t1466 = ct{176};
t1470 = ct{177};
t1481 = ct{178};
t1486 = ct{179};
t1487 = ct{180};
t1495 = ct{181};
t15 = ct{182};
t1505 = ct{183};
t1506 = ct{184};
t1510 = ct{185};
t1512 = ct{186};
t1513 = ct{187};
t1518 = ct{188};
t1521 = ct{189};
t1525 = ct{190};
t1526 = ct{191};
t1528 = ct{192};
t1529 = ct{193};
t1531 = ct{194};
t1535 = ct{195};
t1540 = ct{196};
t1544 = ct{197};
t1552 = ct{198};
t1558 = ct{199};
t1568 = ct{200};
t1575 = ct{201};
t1578 = ct{202};
t1581 = ct{203};
t1586 = ct{204};
t1593 = ct{205};
t1596 = ct{206};
t1597 = ct{207};
t1598 = ct{208};
t1609 = ct{209};
t161 = ct{210};
t1612 = ct{211};
t1618 = ct{212};
t1619 = ct{213};
t162 = ct{214};
t1620 = ct{215};
t1624 = ct{216};
t1628 = ct{217};
t1635 = ct{218};
t1639 = ct{219};
t1640 = ct{220};
t1645 = ct{221};
t1646 = ct{222};
t1651 = ct{223};
t1652 = ct{224};
t1654 = ct{225};
t1657 = ct{226};
t1660 = ct{227};
t1661 = ct{228};
t1664 = ct{229};
t1665 = ct{230};
t1667 = ct{231};
t1672 = ct{232};
t1676 = ct{233};
t1681 = ct{234};
t1685 = ct{235};
t1692 = ct{236};
t1693 = ct{237};
t1694 = ct{238};
t1698 = ct{239};
t1701 = ct{240};
t1702 = ct{241};
t1703 = ct{242};
t1705 = ct{243};
t1706 = ct{244};
t1718 = ct{245};
t1720 = ct{246};
t1722 = ct{247};
t1725 = ct{248};
t1727 = ct{249};
t1730 = ct{250};
t1734 = ct{251};
t1735 = ct{252};
t1742 = ct{253};
t1746 = ct{254};
t1747 = ct{255};
t1751 = ct{256};
t1759 = ct{257};
t1761 = ct{258};
t1763 = ct{259};
t1764 = ct{260};
t1771 = ct{261};
t1774 = ct{262};
t1777 = ct{263};
t1778 = ct{264};
t1779 = ct{265};
t1784 = ct{266};
t1785 = ct{267};
t1786 = ct{268};
t1787 = ct{269};
t1789 = ct{270};
t1790 = ct{271};
t1792 = ct{272};
t1799 = ct{273};
t1802 = ct{274};
t1806 = ct{275};
t1809 = ct{276};
t1810 = ct{277};
t1813 = ct{278};
t1832 = ct{279};
t1840 = ct{280};
t1843 = ct{281};
t1846 = ct{282};
t1851 = ct{283};
t1853 = ct{284};
t1855 = ct{285};
t1857 = ct{286};
t1858 = ct{287};
t1860 = ct{288};
t1865 = ct{289};
t1866 = ct{290};
t1867 = ct{291};
t1882 = ct{292};
t1883 = ct{293};
t1896 = ct{294};
t1898 = ct{295};
t1899 = ct{296};
t1907 = ct{297};
t1910 = ct{298};
t1915 = ct{299};
t1917 = ct{300};
t1918 = ct{301};
t1928 = ct{302};
t1929 = ct{303};
t1932 = ct{304};
t1938 = ct{305};
t1939 = ct{306};
t1942 = ct{307};
t195 = ct{308};
t1952 = ct{309};
t1956 = ct{310};
t1957 = ct{311};
t1959 = ct{312};
t1962 = ct{313};
t1964 = ct{314};
t1965 = ct{315};
t197 = ct{316};
t1970 = ct{317};
t1971 = ct{318};
t1974 = ct{319};
t1976 = ct{320};
t1977 = ct{321};
t1979 = ct{322};
t1981 = ct{323};
t1983 = ct{324};
t1993 = ct{325};
t1997 = ct{326};
t2 = ct{327};
t2000 = ct{328};
t2002 = ct{329};
t2007 = ct{330};
t2008 = ct{331};
t2013 = ct{332};
t2015 = ct{333};
t2016 = ct{334};
t2020 = ct{335};
t2023 = ct{336};
t2024 = ct{337};
t2032 = ct{338};
t2037 = ct{339};
t2038 = ct{340};
t2047 = ct{341};
t2049 = ct{342};
t2057 = ct{343};
t2058 = ct{344};
t2059 = ct{345};
t2061 = ct{346};
t2062 = ct{347};
t2064 = ct{348};
t2065 = ct{349};
t2067 = ct{350};
t2068 = ct{351};
t2069 = ct{352};
t2072 = ct{353};
t2075 = ct{354};
t2076 = ct{355};
t2082 = ct{356};
t2083 = ct{357};
t2086 = ct{358};
t2087 = ct{359};
t2088 = ct{360};
t2096 = ct{361};
t2104 = ct{362};
t2106 = ct{363};
t2107 = ct{364};
t2108 = ct{365};
t2110 = ct{366};
t2111 = ct{367};
t2113 = ct{368};
t2117 = ct{369};
t2123 = ct{370};
t2131 = ct{371};
t2134 = ct{372};
t2135 = ct{373};
t2137 = ct{374};
t2139 = ct{375};
t214 = ct{376};
t2141 = ct{377};
t2147 = ct{378};
t2148 = ct{379};
t2150 = ct{380};
t2152 = ct{381};
t2153 = ct{382};
t2155 = ct{383};
t2156 = ct{384};
t2158 = ct{385};
t2161 = ct{386};
t2174 = ct{387};
t2175 = ct{388};
t2188 = ct{389};
t2189 = ct{390};
t2190 = ct{391};
t2191 = ct{392};
t2192 = ct{393};
t2196 = ct{394};
t2197 = ct{395};
t2202 = ct{396};
t2203 = ct{397};
t2206 = ct{398};
t2208 = ct{399};
t2210 = ct{400};
t2212 = ct{401};
t2215 = ct{402};
t2218 = ct{403};
t2220 = ct{404};
t2222 = ct{405};
t2225 = ct{406};
t2227 = ct{407};
t2237 = ct{408};
t2240 = ct{409};
t2241 = ct{410};
t2242 = ct{411};
t2243 = ct{412};
t2247 = ct{413};
t2248 = ct{414};
t2254 = ct{415};
t2259 = ct{416};
t2268 = ct{417};
t2269 = ct{418};
t2271 = ct{419};
t2274 = ct{420};
t2276 = ct{421};
t2281 = ct{422};
t2282 = ct{423};
t2285 = ct{424};
t2286 = ct{425};
t2287 = ct{426};
t2289 = ct{427};
t2293 = ct{428};
t2305 = ct{429};
t2308 = ct{430};
t2312 = ct{431};
t2316 = ct{432};
t2317 = ct{433};
t2319 = ct{434};
t2322 = ct{435};
t2325 = ct{436};
t2329 = ct{437};
t2334 = ct{438};
t2336 = ct{439};
t2338 = ct{440};
t2339 = ct{441};
t2341 = ct{442};
t2342 = ct{443};
t2345 = ct{444};
t2347 = ct{445};
t2348 = ct{446};
t2352 = ct{447};
t2360 = ct{448};
t2361 = ct{449};
t2364 = ct{450};
t2368 = ct{451};
t2376 = ct{452};
t2387 = ct{453};
t2388 = ct{454};
t2389 = ct{455};
t2390 = ct{456};
t2391 = ct{457};
t2397 = ct{458};
t24 = ct{459};
t2401 = ct{460};
t2404 = ct{461};
t2406 = ct{462};
t2409 = ct{463};
t2410 = ct{464};
t2412 = ct{465};
t2413 = ct{466};
t2419 = ct{467};
t2420 = ct{468};
t2426 = ct{469};
t2427 = ct{470};
t2430 = ct{471};
t2434 = ct{472};
t2435 = ct{473};
t2436 = ct{474};
t2438 = ct{475};
t2447 = ct{476};
t2449 = ct{477};
t2458 = ct{478};
t2463 = ct{479};
t2465 = ct{480};
t2468 = ct{481};
t2471 = ct{482};
t2472 = ct{483};
t2479 = ct{484};
t2483 = ct{485};
t2487 = ct{486};
t2489 = ct{487};
t2495 = ct{488};
t2496 = ct{489};
t25 = ct{490};
t2501 = ct{491};
t2503 = ct{492};
t2504 = ct{493};
t2512 = ct{494};
t2514 = ct{495};
t2516 = ct{496};
t2518 = ct{497};
t2524 = ct{498};
t2526 = ct{499};
t2527 = ct{500};
t2528 = ct{501};
t2536 = ct{502};
t2547 = ct{503};
t2563 = ct{504};
t2564 = ct{505};
t2567 = ct{506};
t2568 = ct{507};
t2569 = ct{508};
t2571 = ct{509};
t2573 = ct{510};
t2574 = ct{511};
t2576 = ct{512};
t2578 = ct{513};
t2579 = ct{514};
t2582 = ct{515};
t2587 = ct{516};
t2589 = ct{517};
t259 = ct{518};
t2590 = ct{519};
t2591 = ct{520};
t2597 = ct{521};
t26 = ct{522};
t260 = ct{523};
t2600 = ct{524};
t2605 = ct{525};
t2613 = ct{526};
t2616 = ct{527};
t2617 = ct{528};
t2621 = ct{529};
t2627 = ct{530};
t2632 = ct{531};
t2636 = ct{532};
t2637 = ct{533};
t2638 = ct{534};
t2646 = ct{535};
t2657 = ct{536};
t2660 = ct{537};
t2663 = ct{538};
t2665 = ct{539};
t2667 = ct{540};
t2669 = ct{541};
t2679 = ct{542};
t2684 = ct{543};
t2688 = ct{544};
t2692 = ct{545};
t2696 = ct{546};
t2699 = ct{547};
t27 = ct{548};
t2700 = ct{549};
t2706 = ct{550};
t2708 = ct{551};
t2712 = ct{552};
t2715 = ct{553};
t2717 = ct{554};
t2718 = ct{555};
t2722 = ct{556};
t2723 = ct{557};
t2728 = ct{558};
t2730 = ct{559};
t2733 = ct{560};
t2734 = ct{561};
t2735 = ct{562};
t2737 = ct{563};
t2738 = ct{564};
t2743 = ct{565};
t2746 = ct{566};
t2754 = ct{567};
t2759 = ct{568};
t276 = ct{569};
t2763 = ct{570};
t277 = ct{571};
t2778 = ct{572};
t2785 = ct{573};
t2787 = ct{574};
t2790 = ct{575};
t2791 = ct{576};
t2794 = ct{577};
t2796 = ct{578};
t2797 = ct{579};
t2798 = ct{580};
t2799 = ct{581};
t2803 = ct{582};
t2805 = ct{583};
t2811 = ct{584};
t2816 = ct{585};
t2818 = ct{586};
t2819 = ct{587};
t2821 = ct{588};
t2823 = ct{589};
t2824 = ct{590};
t2825 = ct{591};
t2829 = ct{592};
t283 = ct{593};
t2831 = ct{594};
t2833 = ct{595};
t2834 = ct{596};
t2836 = ct{597};
t2839 = ct{598};
t284 = ct{599};
t2842 = ct{600};
t2843 = ct{601};
t2844 = ct{602};
t2845 = ct{603};
t2847 = ct{604};
t2849 = ct{605};
t285 = ct{606};
t286 = ct{607};
t2860 = ct{608};
t2861 = ct{609};
t2868 = ct{610};
t287 = ct{611};
t2871 = ct{612};
t2875 = ct{613};
t2876 = ct{614};
t2877 = ct{615};
t2878 = ct{616};
t2879 = ct{617};
t288 = ct{618};
t2883 = ct{619};
t2887 = ct{620};
t2889 = ct{621};
t289 = ct{622};
t2899 = ct{623};
t290 = ct{624};
t291 = ct{625};
t2912 = ct{626};
t2913 = ct{627};
t2914 = ct{628};
t2915 = ct{629};
t2917 = ct{630};
t2918 = ct{631};
t292 = ct{632};
t2920 = ct{633};
t2921 = ct{634};
t2927 = ct{635};
t293 = ct{636};
t2930 = ct{637};
t2936 = ct{638};
t2937 = ct{639};
t294 = ct{640};
t2942 = ct{641};
t2944 = ct{642};
t2945 = ct{643};
t2950 = ct{644};
t2952 = ct{645};
t2956 = ct{646};
t2962 = ct{647};
t2963 = ct{648};
t2965 = ct{649};
t2970 = ct{650};
t2972 = ct{651};
t2977 = ct{652};
t2978 = ct{653};
t2981 = ct{654};
t2994 = ct{655};
t2996 = ct{656};
t2997 = ct{657};
t3 = ct{658};
t3008 = ct{659};
t3009 = ct{660};
t3012 = ct{661};
t3022 = ct{662};
t3027 = ct{663};
t3030 = ct{664};
t3031 = ct{665};
t3034 = ct{666};
t304 = ct{667};
t3040 = ct{668};
t3050 = ct{669};
t3054 = ct{670};
t3062 = ct{671};
t3064 = ct{672};
t3070 = ct{673};
t3076 = ct{674};
t3080 = ct{675};
t3082 = ct{676};
t3084 = ct{677};
t3086 = ct{678};
t3087 = ct{679};
t3091 = ct{680};
t3093 = ct{681};
t3094 = ct{682};
t3096 = ct{683};
t3105 = ct{684};
t3107 = ct{685};
t3109 = ct{686};
t3110 = ct{687};
t3113 = ct{688};
t3121 = ct{689};
t3122 = ct{690};
t3131 = ct{691};
t3138 = ct{692};
t3139 = ct{693};
t3147 = ct{694};
t3149 = ct{695};
t3155 = ct{696};
t3160 = ct{697};
t3161 = ct{698};
t3167 = ct{699};
t3169 = ct{700};
t3170 = ct{701};
t3171 = ct{702};
t3177 = ct{703};
t3178 = ct{704};
t3180 = ct{705};
t3186 = ct{706};
t3192 = ct{707};
t3199 = ct{708};
t3206 = ct{709};
t3207 = ct{710};
t3222 = ct{711};
t3232 = ct{712};
t3235 = ct{713};
t3236 = ct{714};
t3244 = ct{715};
t3247 = ct{716};
t3248 = ct{717};
t3252 = ct{718};
t3256 = ct{719};
t3261 = ct{720};
t3262 = ct{721};
t3263 = ct{722};
t3265 = ct{723};
t3266 = ct{724};
t3270 = ct{725};
t3276 = ct{726};
t3278 = ct{727};
t3286 = ct{728};
t3287 = ct{729};
t3289 = ct{730};
t3299 = ct{731};
t3302 = ct{732};
t3304 = ct{733};
t3307 = ct{734};
t3311 = ct{735};
t3312 = ct{736};
t3315 = ct{737};
t3321 = ct{738};
t3325 = ct{739};
t3326 = ct{740};
t3329 = ct{741};
t3330 = ct{742};
t3331 = ct{743};
t3333 = ct{744};
t3341 = ct{745};
t3344 = ct{746};
t3347 = ct{747};
t3357 = ct{748};
t3378 = ct{749};
t3379 = ct{750};
t3387 = ct{751};
t3390 = ct{752};
t3391 = ct{753};
t3392 = ct{754};
t3397 = ct{755};
t3403 = ct{756};
t3407 = ct{757};
t3412 = ct{758};
t3413 = ct{759};
t3414 = ct{760};
t3415 = ct{761};
t3419 = ct{762};
t3423 = ct{763};
t3424 = ct{764};
t3427 = ct{765};
t3431 = ct{766};
t3432 = ct{767};
t3433 = ct{768};
t3437 = ct{769};
t3438 = ct{770};
t3439 = ct{771};
t3442 = ct{772};
t3445 = ct{773};
t3448 = ct{774};
t3449 = ct{775};
t3458 = ct{776};
t3460 = ct{777};
t3467 = ct{778};
t3471 = ct{779};
t3475 = ct{780};
t3481 = ct{781};
t3482 = ct{782};
t3483 = ct{783};
t3485 = ct{784};
t3486 = ct{785};
t3487 = ct{786};
t3489 = ct{787};
t3490 = ct{788};
t3494 = ct{789};
t3499 = ct{790};
t3501 = ct{791};
t3504 = ct{792};
t3506 = ct{793};
t3510 = ct{794};
t3512 = ct{795};
t3516 = ct{796};
t3521 = ct{797};
t3522 = ct{798};
t3523 = ct{799};
t3524 = ct{800};
t3526 = ct{801};
t3528 = ct{802};
t3529 = ct{803};
t3530 = ct{804};
t3531 = ct{805};
t3534 = ct{806};
t3541 = ct{807};
t3543 = ct{808};
t3544 = ct{809};
t3545 = ct{810};
t3548 = ct{811};
t3550 = ct{812};
t3552 = ct{813};
t3553 = ct{814};
t3556 = ct{815};
t3557 = ct{816};
t3563 = ct{817};
t3575 = ct{818};
t3576 = ct{819};
t3578 = ct{820};
t3582 = ct{821};
t3583 = ct{822};
t3584 = ct{823};
t3587 = ct{824};
t3594 = ct{825};
t3597 = ct{826};
t3598 = ct{827};
t3600 = ct{828};
t3602 = ct{829};
t3609 = ct{830};
t3614 = ct{831};
t3617 = ct{832};
t3621 = ct{833};
t3627 = ct{834};
t3632 = ct{835};
t3634 = ct{836};
t3638 = ct{837};
t3644 = ct{838};
t3647 = ct{839};
t3648 = ct{840};
t3649 = ct{841};
t3652 = ct{842};
t3657 = ct{843};
t3659 = ct{844};
t3661 = ct{845};
t3667 = ct{846};
t3671 = ct{847};
t3672 = ct{848};
t3678 = ct{849};
t3679 = ct{850};
t3680 = ct{851};
t3682 = ct{852};
t3684 = ct{853};
t3697 = ct{854};
t3698 = ct{855};
t3701 = ct{856};
t3704 = ct{857};
t3709 = ct{858};
t3716 = ct{859};
t3719 = ct{860};
t3720 = ct{861};
t3721 = ct{862};
t3722 = ct{863};
t3724 = ct{864};
t3735 = ct{865};
t3738 = ct{866};
t3739 = ct{867};
t3744 = ct{868};
t3745 = ct{869};
t3746 = ct{870};
t3749 = ct{871};
t3750 = ct{872};
t3756 = ct{873};
t376 = ct{874};
t3764 = ct{875};
t3769 = ct{876};
t377 = ct{877};
t3770 = ct{878};
t3771 = ct{879};
t3772 = ct{880};
t3773 = ct{881};
t3774 = ct{882};
t3777 = ct{883};
t3780 = ct{884};
t3784 = ct{885};
t3787 = ct{886};
t3791 = ct{887};
t3792 = ct{888};
t3793 = ct{889};
t3794 = ct{890};
t3802 = ct{891};
t381 = ct{892};
t3811 = ct{893};
t3814 = ct{894};
t3815 = ct{895};
t3817 = ct{896};
t382 = ct{897};
t3823 = ct{898};
t3827 = ct{899};
t3828 = ct{900};
t383 = ct{901};
t3832 = ct{902};
t3834 = ct{903};
t3836 = ct{904};
t3837 = ct{905};
t3841 = ct{906};
t3845 = ct{907};
t3847 = ct{908};
t3848 = ct{909};
t3851 = ct{910};
t3855 = ct{911};
t3856 = ct{912};
t3858 = ct{913};
t3859 = ct{914};
t3862 = ct{915};
t3868 = ct{916};
t3870 = ct{917};
t3879 = ct{918};
t3880 = ct{919};
t3882 = ct{920};
t3883 = ct{921};
t3889 = ct{922};
t390 = ct{923};
t3902 = ct{924};
t3903 = ct{925};
t3906 = ct{926};
t3907 = ct{927};
t3908 = ct{928};
t3909 = ct{929};
t3912 = ct{930};
t3915 = ct{931};
t3916 = ct{932};
t3920 = ct{933};
t3921 = ct{934};
t3923 = ct{935};
t3926 = ct{936};
t3928 = ct{937};
t3929 = ct{938};
t3930 = ct{939};
t3931 = ct{940};
t3932 = ct{941};
t3933 = ct{942};
t3934 = ct{943};
t3936 = ct{944};
t3937 = ct{945};
t3938 = ct{946};
t3939 = ct{947};
t394 = ct{948};
t3940 = ct{949};
t3944 = ct{950};
t3947 = ct{951};
t3948 = ct{952};
t3949 = ct{953};
t3950 = ct{954};
t3951 = ct{955};
t3952 = ct{956};
t3953 = ct{957};
t3954 = ct{958};
t3955 = ct{959};
t3956 = ct{960};
t3957 = ct{961};
t3959 = ct{962};
t3960 = ct{963};
t3961 = ct{964};
t3962 = ct{965};
t3964 = ct{966};
t3965 = ct{967};
t3966 = ct{968};
t3967 = ct{969};
t3969 = ct{970};
t3971 = ct{971};
t3972 = ct{972};
t3973 = ct{973};
t3974 = ct{974};
t3975 = ct{975};
t3976 = ct{976};
t3977 = ct{977};
t3980 = ct{978};
t3981 = ct{979};
t3982 = ct{980};
t3983 = ct{981};
t3985 = ct{982};
t3986 = ct{983};
t3992 = ct{984};
t3993 = ct{985};
t3995 = ct{986};
t3996 = ct{987};
t3998 = ct{988};
t4 = ct{989};
t4000 = ct{990};
t4001 = ct{991};
t4003 = ct{992};
t4005 = ct{993};
t4006 = ct{994};
t4007 = ct{995};
t4008 = ct{996};
t4009 = ct{997};
t4010 = ct{998};
t4012 = ct{999};
t4014 = ct{1000};
t4018 = ct{1001};
t4019 = ct{1002};
t4020 = ct{1003};
t4023 = ct{1004};
t4024 = ct{1005};
t4025 = ct{1006};
t4026 = ct{1007};
t4027 = ct{1008};
t4028 = ct{1009};
t4033 = ct{1010};
t4034 = ct{1011};
t4036 = ct{1012};
t4037 = ct{1013};
t4038 = ct{1014};
t4039 = ct{1015};
t4041 = ct{1016};
t4042 = ct{1017};
t4047 = ct{1018};
t4048 = ct{1019};
t4051 = ct{1020};
t4052 = ct{1021};
t4054 = ct{1022};
t4056 = ct{1023};
t4058 = ct{1024};
t4059 = ct{1025};
t4061 = ct{1026};
t4064 = ct{1027};
t4065 = ct{1028};
t4068 = ct{1029};
t4070 = ct{1030};
t4071 = ct{1031};
t4072 = ct{1032};
t4073 = ct{1033};
t4074 = ct{1034};
t4077 = ct{1035};
t4078 = ct{1036};
t4081 = ct{1037};
t4083 = ct{1038};
t4084 = ct{1039};
t4085 = ct{1040};
t4086 = ct{1041};
t4087 = ct{1042};
t4089 = ct{1043};
t4090 = ct{1044};
t4091 = ct{1045};
t4092 = ct{1046};
t4095 = ct{1047};
t4096 = ct{1048};
t4097 = ct{1049};
t4098 = ct{1050};
t4099 = ct{1051};
t410 = ct{1052};
t4100 = ct{1053};
t4104 = ct{1054};
t4105 = ct{1055};
t4107 = ct{1056};
t4108 = ct{1057};
t4109 = ct{1058};
t411 = ct{1059};
t4111 = ct{1060};
t4112 = ct{1061};
t4115 = ct{1062};
t4116 = ct{1063};
t4117 = ct{1064};
t4119 = ct{1065};
t412 = ct{1066};
t4120 = ct{1067};
t4121 = ct{1068};
t4126 = ct{1069};
t4127 = ct{1070};
t4129 = ct{1071};
t413 = ct{1072};
t4132 = ct{1073};
t4133 = ct{1074};
t4135 = ct{1075};
t4137 = ct{1076};
t4138 = ct{1077};
t4139 = ct{1078};
t414 = ct{1079};
t4140 = ct{1080};
t4141 = ct{1081};
t4143 = ct{1082};
t4144 = ct{1083};
t4145 = ct{1084};
t4147 = ct{1085};
t415 = ct{1086};
t4152 = ct{1087};
t4153 = ct{1088};
t4154 = ct{1089};
t4155 = ct{1090};
t4156 = ct{1091};
t4160 = ct{1092};
t4162 = ct{1093};
t4164 = ct{1094};
t4165 = ct{1095};
t4169 = ct{1096};
t4170 = ct{1097};
t4171 = ct{1098};
t4173 = ct{1099};
t4179 = ct{1100};
t4182 = ct{1101};
t4183 = ct{1102};
t4184 = ct{1103};
t4186 = ct{1104};
t4187 = ct{1105};
t4189 = ct{1106};
t4190 = ct{1107};
t4196 = ct{1108};
t4197 = ct{1109};
t420 = ct{1110};
t4200 = ct{1111};
t4201 = ct{1112};
t4204 = ct{1113};
t4205 = ct{1114};
t4206 = ct{1115};
t4208 = ct{1116};
t421 = ct{1117};
t4210 = ct{1118};
t4211 = ct{1119};
t4212 = ct{1120};
t4213 = ct{1121};
t4214 = ct{1122};
t4215 = ct{1123};
t4216 = ct{1124};
t4217 = ct{1125};
t4218 = ct{1126};
t4219 = ct{1127};
t4220 = ct{1128};
t4222 = ct{1129};
t4223 = ct{1130};
t4224 = ct{1131};
t4225 = ct{1132};
t4227 = ct{1133};
t4228 = ct{1134};
t4231 = ct{1135};
t4232 = ct{1136};
t4233 = ct{1137};
t4234 = ct{1138};
t4236 = ct{1139};
t4237 = ct{1140};
t4238 = ct{1141};
t4239 = ct{1142};
t4240 = ct{1143};
t4241 = ct{1144};
t4243 = ct{1145};
t4245 = ct{1146};
t4247 = ct{1147};
t425 = ct{1148};
t4250 = ct{1149};
t4253 = ct{1150};
t4255 = ct{1151};
t4256 = ct{1152};
t4257 = ct{1153};
t4258 = ct{1154};
t4262 = ct{1155};
t4263 = ct{1156};
t4268 = ct{1157};
t4269 = ct{1158};
t4271 = ct{1159};
t4272 = ct{1160};
t4273 = ct{1161};
t4274 = ct{1162};
t4276 = ct{1163};
t4277 = ct{1164};
t4278 = ct{1165};
t4280 = ct{1166};
t4281 = ct{1167};
t4282 = ct{1168};
t4286 = ct{1169};
t4291 = ct{1170};
t4296 = ct{1171};
t430 = ct{1172};
t4300 = ct{1173};
t4301 = ct{1174};
t4302 = ct{1175};
t4303 = ct{1176};
t4305 = ct{1177};
t4307 = ct{1178};
t4309 = ct{1179};
t431 = ct{1180};
t4310 = ct{1181};
t4311 = ct{1182};
t4312 = ct{1183};
t4313 = ct{1184};
t4314 = ct{1185};
t4315 = ct{1186};
t4316 = ct{1187};
